simulink model "Adaptive_CT_ur10v"  (R2021b)
(part 5 of 20)

Y = ft_5({t100,t1002,t1003,t1004,t1005,t1006,t1007,t1008,t1009,t101,t1010,t1011,t1012,t1013,t1014,t1015,t1016,t1017,t1018,t1019,t1020,t1021,t1022,t1023,t1024,t1025,t1026,t1028,t1029,t1030,t1033,t1034,t1035,t1036,t1038,t104,t1041,t1045,t1046,t1047,t1048,t1049,t1050,t1051,t1052,t1053,t1054,t1055,t1056,t1058,t1059,t106,t1062,t1065,t1066,t1068,t1069,t107,t1070,t1071,t1073,t1074,t1079,t108,t1080,t1082,t1085,t1086,t1087,t1089,t1092,t1093,t1094,t1096,t1097,t1098,t1099,t1106,t1108,t111,t1111,t1119,t112,t1121,t1122,t1123,t1125,t1126,t1128,t1129,t113,t1130,t1131,t1133,t1134,t1135,t1137,t1138,t1139,t1140,t1152,t1153,t1155,t1156,t1157,t1158,t1159,t1161,t1164,t1166,t1167,t1168,t1171,t1172,t1173,t1174,t1178,t1179,t1183,t1184,t1185,t1186,t1187,t1189,t1192,t1193,t1196,t1198,t1199,t12,t1201,t1202,t1203,t1204,t1205,t1208,t1209,t1210,t1211,t1216,t1218,t1219,t1220,t1221,t1222,t1224,t1225,t1226,t1227,t1229,t1230,t1231,t1232,t1233,t1235,t1236,t1237,t1238,t124,t1242,t1245,t1246,t1248,t1250,t1251,t1252,t1255,t1261,t1264,t1265,t1267,t1268,t1269,t127,t1270,t1274,t1277,t1278,t128,t1280,t1283,t1284,t1285,t1287,t1288,t1292,t1294,t1297,t1298,t13,t1300,t1302,t1306,t1307,t131,t1310,t1311,t1313,t1314,t1315,t1316,t1318,t132,t1321,t1323,t1324,t1325,t1328,t1329,t1330,t1331,t1332,t1333,t1334,t1335,t1336,t1337,t1338,t1339,t134,t1341,t1343,t1344,t1345,t1352,t1353,t1354,t1355,t1357,t1358,t136,t1360,t1362,t1366,t1368,t1369,t137,t1370,t1371,t1374,t1375,t1376,t1378,t138,t1382,t1383,t1387,t1389,t1390,t1391,t1392,t1393,t1396,t1398,t1399,t14,t1400,t1402,t1403,t1406,t1407,t1409,t1410,t1411,t1413,t1414,t1415,t1416,t1417,t1418,t1419,t1420,t1421,t1422,t1423,t1425,t1426,t1427,t1434,t1435,t1436,t1437,t1440,t1445,t1446,t1451,t1456,t1458,t1459,t1461,t1462,t1463,t1468,t1470,t1471,t1472,t1474,t1475,t1478,t1483,t1485,t1486,t1491,t1492,t1493,t1494,t1495,t1497,t1499,t15,t150,t1500,t1501,t1503,t1504,t1506,t1507,t1508,t1509,t1516,t1517,t1518,t1519,t152,t1520,t1521,t1523,t1524,t1525,t1527,t1528,t1529,t1531,t1532,t1533,t1534,t1535,t1536,t1537,t1538,t1543,t1545,t1546,t1547,t155,t1552,t1553,t1554,t156,t1574,t158,t1580,t1583,t1585,t1586,t1587,t1588,t1589,t159,t1590,t1591,t1593,t1594,t1599,t1606,t1607,t1610,t1615,t1616,t1618,t162,t1625,t1627,t1628,t163,t1630,t1631,t1632,t1633,t1634,t1635,t1636,t1637,t164,t1644,t1645,t1646,t165,t1650,t1651,t1652,t1653,t1655,t1657,t1659,t1661,t1666,t1667,t1668,t1669,t1670,t1672,t1674,t1675,t1676,t1677,t1678,t1680,t1683,t1684,t1687,t1688,t1690,t1692,t1693,t1695,t1699,t1701,t1704,t1706,t1708,t1709,t171,t1710,t1713,t1714,t1715,t1723,t1724,t1726,t1727,t173,t1733,t1736,t1739,t174,t1740,t1741,t1742,t1743,t1749,t175,t1750,t1751,t1752,t1754,t1755,t1756,t1758,t1759,t1761,t1762,t1768,t1769,t177,t1770,t1771,t1773,t1774,t1775,t1776,t1777,t1778,t1779,t1780,t1781,t1783,t1784,t1786,t1792,t1793,t1794,t1795,t1797,t1799,t18,t1800,t1801,t1805,t1806,t1807,t1808,t1809,t1814,t1815,t1816,t1818,t1819,t1820,t1825,t1826,t1827,t1829,t1830,t1832,t1834,t1835,t1837,t1840,t1844,t1845,t1846,t1848,t1855,t1856,t1861,t1862,t1863,t1865,t1866,t1867,t1868,t1869,t187,t1871,t1874,t1875,t1876,t1877,t1878,t1880,t1881,t1882,t1886,t1888,t1889,t1890,t1891,t1893,t1895,t1897,t1898,t19,t1905,t1907,t1909,t191,t1910,t1916,t1919,t1920,t1921,t1922,t1924,t1925,t1928,t1930,t1931,t1932,t1935,t1937,t1938,t1944,t1947,t1949,t1953,t1959,t196,t1961,t1962,t1963,t1965,t1966,t1968,t1969,t1971,t1972,t1973,t1976,t1977,t1983,t1984,t1985,t1988,t199,t1990,t1995,t1996,t1999,t1d,t1dd,t200,t201,t2017,t202,t2023,t2027,t2028,t2030,t2032,t2037,t2044,t2049,t2058,t2059,t206,t2060,t2061,t2063,t2064,t2067,t2068,t2070,t2074,t2075,t2078,t2079,t2080,t2081,t2082,t2085,t2086,t2087,t2090,t2091,t2092,t2093,t2094,t2096,t2097,t21,t210,t2100,t2101,t2103,t2109,t2110,t2112,t2113,t2117,t2118,t2119,t2121,t2122,t2123,t2124,t2127,t2128,t2131,t2132,t2133,t2134,t2135,t2136,t2137,t2138,t2139,t2140,t2141,t2142,t2144,t2145,t2147,t215,t2150,t2153,t2155,t2156,t2159,t2160,t2161,t2162,t2167,t2168,t2169,t2170,t2171,t2172,t2173,t2174,t2177,t2178,t2180,t2181,t2183,t2184,t2189,t219,t2190,t2193,t2194,t2196,t2198,t2199,t22,t220,t2200,t2202,t2204,t2206,t2207,t221,t2210,t2211,t2212,t2216,t2219,t2221,t2222,t2225,t2227,t2228,t2233,t2235,t2240,t2241,t2243,t2244,t2245,t2247,t2256,t2257,t2259,t226,t2260,t2261,t2262,t2263,t2264,t2265,t2267,t2270,t2279,t2281,t2283,t2286,t229,t2292,t2294,t2298,t23,t2300,t231,t2311,t2315,t2318,t232,t2323,t233,t2335,t2339,t2340,t2343,t2344,t2345,t2346,t2347,t2348,t2352,t2353,t2354,t2357,t2359,t2363,t2365,t2366,t2368,t2370,t2371,t2372,t2374,t2379,t2380,t2382,t2385,t2388,t2389,t2390,t2391,t2393,t2395,t2397,t2398,t2399,t24,t2400,t2401,t2402,t2403,t2405,t2406,t2407,t2408,t2409,t2410,t2412,t2413,t2414,t2416,t2417,t2423,t2424,t2426,t2428,t243,t2434,t2438,t2439,t244,t2440,t2441,t2447,t2448,t245,t2453,t2454,t2457,t2458,t2462,t2467,t247,t2471,t2472,t2473,t2474,t2475,t2477,t2478,t248,t2480,t2481,t2484,t2485,t249,t2490,t2497,t25,t2505,t2507,t2508,t2509,t2511,t2515,t2516,t2518,t2519,t2520,t2523,t2524,t2527,t2529,t2530,t2547,t255,t2553,t2554,t2557,t256,t2560,t2565,t2571,t2572,t2576,t2578,t258,t2580,t2581,t2593,t2599,t26,t2606,t2608,t2611,t2619,t2623,t2628,t2630,t2631,t2635,t2642,t2644,t2648,t2649,t2650,t2651,t2653,t2654,t2655,t2658,t2659,t2662,t2663,t2664,t2666,t2671,t2672,t2678,t2680,t2682,t2686,t2687,t2688,t2690,t2694,t2695,t27,t2702,t2704,t2705,t2708,t2711,t2715,t2718,t2719,t2723,t2724,t2727,t2729,t2731,t2736,t2737,t2739,t2741,t2743,t2744,t2745,t2747,t2749,t2750,t2753,t2755,t2760,t2761,t2762,t2764,t2765,t2766,t2768,t2772,t2775,t2776,t2777,t2779,t2780,t2781,t2783,t279,t2790,t2794,t2796,t2798,t2799,t28,t2807,t2813,t2824,t2826,t283,t2838,t2839,t2841,t2843,t2849,t2860,t2862,t2863,t2868,t2871,t2876,t2877,t2879,t2894,t2897,t29,t2901,t2912,t2914,t2915,t2916,t2919,t2925,t2927,t2929,t2934,t2936,t2937,t2946,t2947,t2951,t2952,t2953,t2954,t2956,t2959,t2966,t2970,t2971,t2978,t2979,t2983,t2985,t2989,t299,t2992,t2995,t2996,t2999,t2d,t2dd,t30,t3007,t3008,t301,t3012,t3013,t3014,t3018,t3023,t3028,t303,t3030,t3031,t3032,t3033,t3035,t3038,t3039,t3042,t3043,t3059,t3060,t3066,t3069,t3071,t3072,t3073,t3078,t3079,t308,t3080,t3082,t3083,t3086,t3087,t3088,t309,t3099,t31,t3101,t3102,t3103,t3122,t3123,t3125,t3129,t3130,t3148,t315,t3154,t3160,t3163,t3166,t3168,t3169,t317,t3175,t3176,t3177,t318,t3183,t3185,t319,t320,t3207,t321,t3214,t3230,t3232,t3234,t3237,t325,t3250,t3251,t3259,t3260,t3272,t3288,t3289,t329,t3291,t3292,t3298,t330,t3306,t3308,t331,t3318,t332,t3321,t333,t3330,t3331,t3332,t3335,t334,t3340,t3341,t3342,t3343,t3345,t3348,t3349,t3351,t3354,t3355,t3360,t3368,t3381,t3383,t3384,t3388,t3391,t3399,t34,t3400,t3401,t3404,t3405,t341,t3414,t3415,t3416,t342,t3421,t3429,t343,t3431,t3432,t3433,t3439,t344,t3440,t3445,t345,t3452,t3456,t3457,t3458,t3459,t346,t3460,t3461,t3466,t3467,t3468,t3469,t347,t3488,t3498,t35,t3500,t3504,t3509,t3510,t3513,t3516,t3517,t3523,t3531,t354,t3543,t3544,t3546,t3556,t3557,t3567,t3568,t3574,t3575,t3578,t3579,t3580,t3582,t3590,t3598,t36,t3601,t3606,t3612,t3617,t3622,t3628,t3630,t364,t3649,t365,t3674,t3678,t368,t3683,t3685,t3686,t3687,t3697,t37,t3701,t3704,t3712,t3716,t3721,t3724,t3734,t3741,t3743,t3744,t3745,t3747,t3750,t3751,t3758,t3761,t3768,t3769,t3770,t3771,t3779,t3785,t3786,t3792,t3796,t38,t3813,t3817,t3821,t3822,t3830,t384,t3840,t3843,t3846,t3852,t3853,t3871,t3872,t3875,t3877,t3878,t3897,t39,t3903,t3906,t3907,t392,t3923,t393,t394,t3940,t3941,t3943,t395,t3d,t3dd,t401,t402,t4025,t403,t404,t4059,t4069,t4071,t4075,t4076,t4084,t4086,t4098,t41,t410,t411,t412,t4126,t4129,t413,t4133,t4134,t4135,t4139,t414,t4140,t4144,t4146,t4147,t415,t4150,t4152,t4157,t4159,t416,t4172,t418,t419,t42,t420,t4203,t4207,t4212,t4230,t4236,t425,t4299,t43,t4304,t431,t4325,t4332,t434,t437,t441,t442,t443,t444,t446,t4466,t453,t4538,t454,t455,t4551,t4579,t459,t467,t470,t478,t48,t483,t484,t486,t487,t488,t489,t492,t493,t494,t495,t496,t497,t498,t499,t4d,t4dd,t50,t501,t502,t503,t508,t51,t514,t515,t516,t519,t523,t524,t529,t53,t530,t531,t532,t537,t542,t543,t544,t546,t547,t548,t549,t55,t550,t552,t553,t554,t56,t562,t566,t569,t57,t570,t58,t580,t582,t587,t588,t589,t590,t591,t593,t595,t596,t598,t5d,t5dd,t600,t601,t602,t604,t605,t608,t609,t61,t612,t614,t615,t616,t617,t623,t627,t63,t631,t632,t633,t634,t635,t636,t637,t639,t641,t642,t643,t644,t645,t646,t647,t648,t649,t650,t651,t652,t653,t654,t655,t658,t659,t660,t662,t663,t664,t665,t667,t668,t669,t670,t671,t673,t675,t680,t681,t682,t684,t685,t687,t689,t69,t690,t694,t695,t696,t698,t699,t6d,t6dd,t701,t702,t703,t705,t706,t71,t711,t712,t713,t714,t720,t721,t723,t724,t725,t726,t729,t731,t732,t733,t735,t736,t738,t739,t740,t742,t745,t746,t747,t748,t749,t75,t752,t755,t759,t760,t761,t763,t764,t772,t774,t775,t776,t780,t781,t782,t785,t788,t789,t793,t799,t8,t802,t805,t806,t807,t808,t817,t82,t820,t823,t824,t825,t826,t827,t828,t830,t831,t832,t833,t835,t836,t838,t842,t843,t844,t846,t848,t849,t850,t851,t852,t853,t854,t855,t859,t861,t865,t866,t869,t870,t871,t873,t874,t879,t88,t880,t882,t883,t884,t885,t887,t888,t889,t890,t891,t892,t895,t896,t897,t898,t899,t9,t900,t904,t907,t908,t909,t910,t911,t912,t915,t917,t919,t922,t923,t927,t928,t931,t932,t937,t938,t943,t944,t945,t952,t954,t955,t956,t959,t960,t961,t962,t963,t964,t965,t966,t968,t969,t970,t972,t973,t974,t975,t978,t979,t980,t981,t982,t983,t984,t985,t986,t987,t989,t992,t993,t994,t997,t999});
end
function Y = ft_5(ct)
t100 = ct{1};
t1002 = ct{2};
t1003 = ct{3};
t1004 = ct{4};
t1005 = ct{5};
t1006 = ct{6};
t1007 = ct{7};
t1008 = ct{8};
t1009 = ct{9};
t101 = ct{10};
t1010 = ct{11};
t1011 = ct{12};
t1012 = ct{13};
t1013 = ct{14};
t1014 = ct{15};
t1015 = ct{16};
t1016 = ct{17};
t1017 = ct{18};
t1018 = ct{19};
t1019 = ct{20};
t1020 = ct{21};
t1021 = ct{22};
t1022 = ct{23};
t1023 = ct{24};
t1024 = ct{25};
t1025 = ct{26};
t1026 = ct{27};
t1028 = ct{28};
t1029 = ct{29};
t1030 = ct{30};
t1033 = ct{31};
t1034 = ct{32};
t1035 = ct{33};
t1036 = ct{34};
t1038 = ct{35};
t104 = ct{36};
t1041 = ct{37};
t1045 = ct{38};
t1046 = ct{39};
t1047 = ct{40};
t1048 = ct{41};
t1049 = ct{42};
t1050 = ct{43};
t1051 = ct{44};
t1052 = ct{45};
t1053 = ct{46};
t1054 = ct{47};
t1055 = ct{48};
t1056 = ct{49};
t1058 = ct{50};
t1059 = ct{51};
t106 = ct{52};
t1062 = ct{53};
t1065 = ct{54};
t1066 = ct{55};
t1068 = ct{56};
t1069 = ct{57};
t107 = ct{58};
t1070 = ct{59};
t1071 = ct{60};
t1073 = ct{61};
t1074 = ct{62};
t1079 = ct{63};
t108 = ct{64};
t1080 = ct{65};
t1082 = ct{66};
t1085 = ct{67};
t1086 = ct{68};
t1087 = ct{69};
t1089 = ct{70};
t1092 = ct{71};
t1093 = ct{72};
t1094 = ct{73};
t1096 = ct{74};
t1097 = ct{75};
t1098 = ct{76};
t1099 = ct{77};
t1106 = ct{78};
t1108 = ct{79};
t111 = ct{80};
t1111 = ct{81};
t1119 = ct{82};
t112 = ct{83};
t1121 = ct{84};
t1122 = ct{85};
t1123 = ct{86};
t1125 = ct{87};
t1126 = ct{88};
t1128 = ct{89};
t1129 = ct{90};
t113 = ct{91};
t1130 = ct{92};
t1131 = ct{93};
t1133 = ct{94};
t1134 = ct{95};
t1135 = ct{96};
t1137 = ct{97};
t1138 = ct{98};
t1139 = ct{99};
t1140 = ct{100};
t1152 = ct{101};
t1153 = ct{102};
t1155 = ct{103};
t1156 = ct{104};
t1157 = ct{105};
t1158 = ct{106};
t1159 = ct{107};
t1161 = ct{108};
t1164 = ct{109};
t1166 = ct{110};
t1167 = ct{111};
t1168 = ct{112};
t1171 = ct{113};
t1172 = ct{114};
t1173 = ct{115};
t1174 = ct{116};
t1178 = ct{117};
t1179 = ct{118};
t1183 = ct{119};
t1184 = ct{120};
t1185 = ct{121};
t1186 = ct{122};
t1187 = ct{123};
t1189 = ct{124};
t1192 = ct{125};
t1193 = ct{126};
t1196 = ct{127};
t1198 = ct{128};
t1199 = ct{129};
t12 = ct{130};
t1201 = ct{131};
t1202 = ct{132};
t1203 = ct{133};
t1204 = ct{134};
t1205 = ct{135};
t1208 = ct{136};
t1209 = ct{137};
t1210 = ct{138};
t1211 = ct{139};
t1216 = ct{140};
t1218 = ct{141};
t1219 = ct{142};
t1220 = ct{143};
t1221 = ct{144};
t1222 = ct{145};
t1224 = ct{146};
t1225 = ct{147};
t1226 = ct{148};
t1227 = ct{149};
t1229 = ct{150};
t1230 = ct{151};
t1231 = ct{152};
t1232 = ct{153};
t1233 = ct{154};
t1235 = ct{155};
t1236 = ct{156};
t1237 = ct{157};
t1238 = ct{158};
t124 = ct{159};
t1242 = ct{160};
t1245 = ct{161};
t1246 = ct{162};
t1248 = ct{163};
t1250 = ct{164};
t1251 = ct{165};
t1252 = ct{166};
t1255 = ct{167};
t1261 = ct{168};
t1264 = ct{169};
t1265 = ct{170};
t1267 = ct{171};
t1268 = ct{172};
t1269 = ct{173};
t127 = ct{174};
t1270 = ct{175};
t1274 = ct{176};
t1277 = ct{177};
t1278 = ct{178};
t128 = ct{179};
t1280 = ct{180};
t1283 = ct{181};
t1284 = ct{182};
t1285 = ct{183};
t1287 = ct{184};
t1288 = ct{185};
t1292 = ct{186};
t1294 = ct{187};
t1297 = ct{188};
t1298 = ct{189};
t13 = ct{190};
t1300 = ct{191};
t1302 = ct{192};
t1306 = ct{193};
t1307 = ct{194};
t131 = ct{195};
t1310 = ct{196};
t1311 = ct{197};
t1313 = ct{198};
t1314 = ct{199};
t1315 = ct{200};
t1316 = ct{201};
t1318 = ct{202};
t132 = ct{203};
t1321 = ct{204};
t1323 = ct{205};
t1324 = ct{206};
t1325 = ct{207};
t1328 = ct{208};
t1329 = ct{209};
t1330 = ct{210};
t1331 = ct{211};
t1332 = ct{212};
t1333 = ct{213};
t1334 = ct{214};
t1335 = ct{215};
t1336 = ct{216};
t1337 = ct{217};
t1338 = ct{218};
t1339 = ct{219};
t134 = ct{220};
t1341 = ct{221};
t1343 = ct{222};
t1344 = ct{223};
t1345 = ct{224};
t1352 = ct{225};
t1353 = ct{226};
t1354 = ct{227};
t1355 = ct{228};
t1357 = ct{229};
t1358 = ct{230};
t136 = ct{231};
t1360 = ct{232};
t1362 = ct{233};
t1366 = ct{234};
t1368 = ct{235};
t1369 = ct{236};
t137 = ct{237};
t1370 = ct{238};
t1371 = ct{239};
t1374 = ct{240};
t1375 = ct{241};
t1376 = ct{242};
t1378 = ct{243};
t138 = ct{244};
t1382 = ct{245};
t1383 = ct{246};
t1387 = ct{247};
t1389 = ct{248};
t1390 = ct{249};
t1391 = ct{250};
t1392 = ct{251};
t1393 = ct{252};
t1396 = ct{253};
t1398 = ct{254};
t1399 = ct{255};
t14 = ct{256};
t1400 = ct{257};
t1402 = ct{258};
t1403 = ct{259};
t1406 = ct{260};
t1407 = ct{261};
t1409 = ct{262};
t1410 = ct{263};
t1411 = ct{264};
t1413 = ct{265};
t1414 = ct{266};
t1415 = ct{267};
t1416 = ct{268};
t1417 = ct{269};
t1418 = ct{270};
t1419 = ct{271};
t1420 = ct{272};
t1421 = ct{273};
t1422 = ct{274};
t1423 = ct{275};
t1425 = ct{276};
t1426 = ct{277};
t1427 = ct{278};
t1434 = ct{279};
t1435 = ct{280};
t1436 = ct{281};
t1437 = ct{282};
t1440 = ct{283};
t1445 = ct{284};
t1446 = ct{285};
t1451 = ct{286};
t1456 = ct{287};
t1458 = ct{288};
t1459 = ct{289};
t1461 = ct{290};
t1462 = ct{291};
t1463 = ct{292};
t1468 = ct{293};
t1470 = ct{294};
t1471 = ct{295};
t1472 = ct{296};
t1474 = ct{297};
t1475 = ct{298};
t1478 = ct{299};
t1483 = ct{300};
t1485 = ct{301};
t1486 = ct{302};
t1491 = ct{303};
t1492 = ct{304};
t1493 = ct{305};
t1494 = ct{306};
t1495 = ct{307};
t1497 = ct{308};
t1499 = ct{309};
t15 = ct{310};
t150 = ct{311};
t1500 = ct{312};
t1501 = ct{313};
t1503 = ct{314};
t1504 = ct{315};
t1506 = ct{316};
t1507 = ct{317};
t1508 = ct{318};
t1509 = ct{319};
t1516 = ct{320};
t1517 = ct{321};
t1518 = ct{322};
t1519 = ct{323};
t152 = ct{324};
t1520 = ct{325};
t1521 = ct{326};
t1523 = ct{327};
t1524 = ct{328};
t1525 = ct{329};
t1527 = ct{330};
t1528 = ct{331};
t1529 = ct{332};
t1531 = ct{333};
t1532 = ct{334};
t1533 = ct{335};
t1534 = ct{336};
t1535 = ct{337};
t1536 = ct{338};
t1537 = ct{339};
t1538 = ct{340};
t1543 = ct{341};
t1545 = ct{342};
t1546 = ct{343};
t1547 = ct{344};
t155 = ct{345};
t1552 = ct{346};
t1553 = ct{347};
t1554 = ct{348};
t156 = ct{349};
t1574 = ct{350};
t158 = ct{351};
t1580 = ct{352};
t1583 = ct{353};
t1585 = ct{354};
t1586 = ct{355};
t1587 = ct{356};
t1588 = ct{357};
t1589 = ct{358};
t159 = ct{359};
t1590 = ct{360};
t1591 = ct{361};
t1593 = ct{362};
t1594 = ct{363};
t1599 = ct{364};
t1606 = ct{365};
t1607 = ct{366};
t1610 = ct{367};
t1615 = ct{368};
t1616 = ct{369};
t1618 = ct{370};
t162 = ct{371};
t1625 = ct{372};
t1627 = ct{373};
t1628 = ct{374};
t163 = ct{375};
t1630 = ct{376};
t1631 = ct{377};
t1632 = ct{378};
t1633 = ct{379};
t1634 = ct{380};
t1635 = ct{381};
t1636 = ct{382};
t1637 = ct{383};
t164 = ct{384};
t1644 = ct{385};
t1645 = ct{386};
t1646 = ct{387};
t165 = ct{388};
t1650 = ct{389};
t1651 = ct{390};
t1652 = ct{391};
t1653 = ct{392};
t1655 = ct{393};
t1657 = ct{394};
t1659 = ct{395};
t1661 = ct{396};
t1666 = ct{397};
t1667 = ct{398};
t1668 = ct{399};
t1669 = ct{400};
t1670 = ct{401};
t1672 = ct{402};
t1674 = ct{403};
t1675 = ct{404};
t1676 = ct{405};
t1677 = ct{406};
t1678 = ct{407};
t1680 = ct{408};
t1683 = ct{409};
t1684 = ct{410};
t1687 = ct{411};
t1688 = ct{412};
t1690 = ct{413};
t1692 = ct{414};
t1693 = ct{415};
t1695 = ct{416};
t1699 = ct{417};
t1701 = ct{418};
t1704 = ct{419};
t1706 = ct{420};
t1708 = ct{421};
t1709 = ct{422};
t171 = ct{423};
t1710 = ct{424};
t1713 = ct{425};
t1714 = ct{426};
t1715 = ct{427};
t1723 = ct{428};
t1724 = ct{429};
t1726 = ct{430};
t1727 = ct{431};
t173 = ct{432};
t1733 = ct{433};
t1736 = ct{434};
t1739 = ct{435};
t174 = ct{436};
t1740 = ct{437};
t1741 = ct{438};
t1742 = ct{439};
t1743 = ct{440};
t1749 = ct{441};
t175 = ct{442};
t1750 = ct{443};
t1751 = ct{444};
t1752 = ct{445};
t1754 = ct{446};
t1755 = ct{447};
t1756 = ct{448};
t1758 = ct{449};
t1759 = ct{450};
t1761 = ct{451};
t1762 = ct{452};
t1768 = ct{453};
t1769 = ct{454};
t177 = ct{455};
t1770 = ct{456};
t1771 = ct{457};
t1773 = ct{458};
t1774 = ct{459};
t1775 = ct{460};
t1776 = ct{461};
t1777 = ct{462};
t1778 = ct{463};
t1779 = ct{464};
t1780 = ct{465};
t1781 = ct{466};
t1783 = ct{467};
t1784 = ct{468};
t1786 = ct{469};
t1792 = ct{470};
t1793 = ct{471};
t1794 = ct{472};
t1795 = ct{473};
t1797 = ct{474};
t1799 = ct{475};
t18 = ct{476};
t1800 = ct{477};
t1801 = ct{478};
t1805 = ct{479};
t1806 = ct{480};
t1807 = ct{481};
t1808 = ct{482};
t1809 = ct{483};
t1814 = ct{484};
t1815 = ct{485};
t1816 = ct{486};
t1818 = ct{487};
t1819 = ct{488};
t1820 = ct{489};
t1825 = ct{490};
t1826 = ct{491};
t1827 = ct{492};
t1829 = ct{493};
t1830 = ct{494};
t1832 = ct{495};
t1834 = ct{496};
t1835 = ct{497};
t1837 = ct{498};
t1840 = ct{499};
t1844 = ct{500};
t1845 = ct{501};
t1846 = ct{502};
t1848 = ct{503};
t1855 = ct{504};
t1856 = ct{505};
t1861 = ct{506};
t1862 = ct{507};
t1863 = ct{508};
t1865 = ct{509};
t1866 = ct{510};
t1867 = ct{511};
t1868 = ct{512};
t1869 = ct{513};
t187 = ct{514};
t1871 = ct{515};
t1874 = ct{516};
t1875 = ct{517};
t1876 = ct{518};
t1877 = ct{519};
t1878 = ct{520};
t1880 = ct{521};
t1881 = ct{522};
t1882 = ct{523};
t1886 = ct{524};
t1888 = ct{525};
t1889 = ct{526};
t1890 = ct{527};
t1891 = ct{528};
t1893 = ct{529};
t1895 = ct{530};
t1897 = ct{531};
t1898 = ct{532};
t19 = ct{533};
t1905 = ct{534};
t1907 = ct{535};
t1909 = ct{536};
t191 = ct{537};
t1910 = ct{538};
t1916 = ct{539};
t1919 = ct{540};
t1920 = ct{541};
t1921 = ct{542};
t1922 = ct{543};
t1924 = ct{544};
t1925 = ct{545};
t1928 = ct{546};
t1930 = ct{547};
t1931 = ct{548};
t1932 = ct{549};
t1935 = ct{550};
t1937 = ct{551};
t1938 = ct{552};
t1944 = ct{553};
t1947 = ct{554};
t1949 = ct{555};
t1953 = ct{556};
t1959 = ct{557};
t196 = ct{558};
t1961 = ct{559};
t1962 = ct{560};
t1963 = ct{561};
t1965 = ct{562};
t1966 = ct{563};
t1968 = ct{564};
t1969 = ct{565};
t1971 = ct{566};
t1972 = ct{567};
t1973 = ct{568};
t1976 = ct{569};
t1977 = ct{570};
t1983 = ct{571};
t1984 = ct{572};
t1985 = ct{573};
t1988 = ct{574};
t199 = ct{575};
t1990 = ct{576};
t1995 = ct{577};
t1996 = ct{578};
t1999 = ct{579};
t1d = ct{580};
t1dd = ct{581};
t200 = ct{582};
t201 = ct{583};
t2017 = ct{584};
t202 = ct{585};
t2023 = ct{586};
t2027 = ct{587};
t2028 = ct{588};
t2030 = ct{589};
t2032 = ct{590};
t2037 = ct{591};
t2044 = ct{592};
t2049 = ct{593};
t2058 = ct{594};
t2059 = ct{595};
t206 = ct{596};
t2060 = ct{597};
t2061 = ct{598};
t2063 = ct{599};
t2064 = ct{600};
t2067 = ct{601};
t2068 = ct{602};
t2070 = ct{603};
t2074 = ct{604};
t2075 = ct{605};
t2078 = ct{606};
t2079 = ct{607};
t2080 = ct{608};
t2081 = ct{609};
t2082 = ct{610};
t2085 = ct{611};
t2086 = ct{612};
t2087 = ct{613};
t2090 = ct{614};
t2091 = ct{615};
t2092 = ct{616};
t2093 = ct{617};
t2094 = ct{618};
t2096 = ct{619};
t2097 = ct{620};
t21 = ct{621};
t210 = ct{622};
t2100 = ct{623};
t2101 = ct{624};
t2103 = ct{625};
t2109 = ct{626};
t2110 = ct{627};
t2112 = ct{628};
t2113 = ct{629};
t2117 = ct{630};
t2118 = ct{631};
t2119 = ct{632};
t2121 = ct{633};
t2122 = ct{634};
t2123 = ct{635};
t2124 = ct{636};
t2127 = ct{637};
t2128 = ct{638};
t2131 = ct{639};
t2132 = ct{640};
t2133 = ct{641};
t2134 = ct{642};
t2135 = ct{643};
t2136 = ct{644};
t2137 = ct{645};
t2138 = ct{646};
t2139 = ct{647};
t2140 = ct{648};
t2141 = ct{649};
t2142 = ct{650};
t2144 = ct{651};
t2145 = ct{652};
t2147 = ct{653};
t215 = ct{654};
t2150 = ct{655};
t2153 = ct{656};
t2155 = ct{657};
t2156 = ct{658};
t2159 = ct{659};
t2160 = ct{660};
t2161 = ct{661};
t2162 = ct{662};
t2167 = ct{663};
t2168 = ct{664};
t2169 = ct{665};
t2170 = ct{666};
t2171 = ct{667};
t2172 = ct{668};
t2173 = ct{669};
t2174 = ct{670};
t2177 = ct{671};
t2178 = ct{672};
t2180 = ct{673};
t2181 = ct{674};
t2183 = ct{675};
t2184 = ct{676};
t2189 = ct{677};
t219 = ct{678};
t2190 = ct{679};
t2193 = ct{680};
t2194 = ct{681};
t2196 = ct{682};
t2198 = ct{683};
t2199 = ct{684};
t22 = ct{685};
t220 = ct{686};
t2200 = ct{687};
t2202 = ct{688};
t2204 = ct{689};
t2206 = ct{690};
t2207 = ct{691};
t221 = ct{692};
t2210 = ct{693};
t2211 = ct{694};
t2212 = ct{695};
t2216 = ct{696};
t2219 = ct{697};
t2221 = ct{698};
t2222 = ct{699};
t2225 = ct{700};
t2227 = ct{701};
t2228 = ct{702};
t2233 = ct{703};
t2235 = ct{704};
t2240 = ct{705};
t2241 = ct{706};
t2243 = ct{707};
t2244 = ct{708};
t2245 = ct{709};
t2247 = ct{710};
t2256 = ct{711};
t2257 = ct{712};
t2259 = ct{713};
t226 = ct{714};
t2260 = ct{715};
t2261 = ct{716};
t2262 = ct{717};
t2263 = ct{718};
t2264 = ct{719};
t2265 = ct{720};
t2267 = ct{721};
t2270 = ct{722};
t2279 = ct{723};
t2281 = ct{724};
t2283 = ct{725};
t2286 = ct{726};
t229 = ct{727};
t2292 = ct{728};
t2294 = ct{729};
t2298 = ct{730};
t23 = ct{731};
t2300 = ct{732};
t231 = ct{733};
t2311 = ct{734};
t2315 = ct{735};
t2318 = ct{736};
t232 = ct{737};
t2323 = ct{738};
t233 = ct{739};
t2335 = ct{740};
t2339 = ct{741};
t2340 = ct{742};
t2343 = ct{743};
t2344 = ct{744};
t2345 = ct{745};
t2346 = ct{746};
t2347 = ct{747};
t2348 = ct{748};
t2352 = ct{749};
t2353 = ct{750};
t2354 = ct{751};
t2357 = ct{752};
t2359 = ct{753};
t2363 = ct{754};
t2365 = ct{755};
t2366 = ct{756};
t2368 = ct{757};
t2370 = ct{758};
t2371 = ct{759};
t2372 = ct{760};
t2374 = ct{761};
t2379 = ct{762};
t2380 = ct{763};
t2382 = ct{764};
t2385 = ct{765};
t2388 = ct{766};
t2389 = ct{767};
t2390 = ct{768};
t2391 = ct{769};
t2393 = ct{770};
t2395 = ct{771};
t2397 = ct{772};
t2398 = ct{773};
t2399 = ct{774};
t24 = ct{775};
t2400 = ct{776};
t2401 = ct{777};
t2402 = ct{778};
t2403 = ct{779};
t2405 = ct{780};
t2406 = ct{781};
t2407 = ct{782};
t2408 = ct{783};
t2409 = ct{784};
t2410 = ct{785};
t2412 = ct{786};
t2413 = ct{787};
t2414 = ct{788};
t2416 = ct{789};
t2417 = ct{790};
t2423 = ct{791};
t2424 = ct{792};
t2426 = ct{793};
t2428 = ct{794};
t243 = ct{795};
t2434 = ct{796};
t2438 = ct{797};
t2439 = ct{798};
t244 = ct{799};
t2440 = ct{800};
t2441 = ct{801};
t2447 = ct{802};
t2448 = ct{803};
t245 = ct{804};
t2453 = ct{805};
t2454 = ct{806};
t2457 = ct{807};
t2458 = ct{808};
t2462 = ct{809};
t2467 = ct{810};
t247 = ct{811};
t2471 = ct{812};
t2472 = ct{813};
t2473 = ct{814};
t2474 = ct{815};
t2475 = ct{816};
t2477 = ct{817};
t2478 = ct{818};
t248 = ct{819};
t2480 = ct{820};
t2481 = ct{821};
t2484 = ct{822};
t2485 = ct{823};
t249 = ct{824};
t2490 = ct{825};
t2497 = ct{826};
t25 = ct{827};
t2505 = ct{828};
t2507 = ct{829};
t2508 = ct{830};
t2509 = ct{831};
t2511 = ct{832};
t2515 = ct{833};
t2516 = ct{834};
t2518 = ct{835};
t2519 = ct{836};
t2520 = ct{837};
t2523 = ct{838};
t2524 = ct{839};
t2527 = ct{840};
t2529 = ct{841};
t2530 = ct{842};
t2547 = ct{843};
t255 = ct{844};
t2553 = ct{845};
t2554 = ct{846};
t2557 = ct{847};
t256 = ct{848};
t2560 = ct{849};
t2565 = ct{850};
t2571 = ct{851};
t2572 = ct{852};
t2576 = ct{853};
t2578 = ct{854};
t258 = ct{855};
t2580 = ct{856};
t2581 = ct{857};
t2593 = ct{858};
t2599 = ct{859};
t26 = ct{860};
t2606 = ct{861};
t2608 = ct{862};
t2611 = ct{863};
t2619 = ct{864};
t2623 = ct{865};
t2628 = ct{866};
t2630 = ct{867};
t2631 = ct{868};
t2635 = ct{869};
t2642 = ct{870};
t2644 = ct{871};
t2648 = ct{872};
t2649 = ct{873};
t2650 = ct{874};
t2651 = ct{875};
t2653 = ct{876};
t2654 = ct{877};
t2655 = ct{878};
t2658 = ct{879};
t2659 = ct{880};
t2662 = ct{881};
t2663 = ct{882};
t2664 = ct{883};
t2666 = ct{884};
t2671 = ct{885};
t2672 = ct{886};
t2678 = ct{887};
t2680 = ct{888};
t2682 = ct{889};
t2686 = ct{890};
t2687 = ct{891};
t2688 = ct{892};
t2690 = ct{893};
t2694 = ct{894};
t2695 = ct{895};
t27 = ct{896};
t2702 = ct{897};
t2704 = ct{898};
t2705 = ct{899};
t2708 = ct{900};
t2711 = ct{901};
t2715 = ct{902};
t2718 = ct{903};
t2719 = ct{904};
t2723 = ct{905};
t2724 = ct{906};
t2727 = ct{907};
t2729 = ct{908};
t2731 = ct{909};
t2736 = ct{910};
t2737 = ct{911};
t2739 = ct{912};
t2741 = ct{913};
t2743 = ct{914};
t2744 = ct{915};
t2745 = ct{916};
t2747 = ct{917};
t2749 = ct{918};
t2750 = ct{919};
t2753 = ct{920};
t2755 = ct{921};
t2760 = ct{922};
t2761 = ct{923};
t2762 = ct{924};
t2764 = ct{925};
t2765 = ct{926};
t2766 = ct{927};
t2768 = ct{928};
t2772 = ct{929};
t2775 = ct{930};
t2776 = ct{931};
t2777 = ct{932};
t2779 = ct{933};
t2780 = ct{934};
t2781 = ct{935};
t2783 = ct{936};
t279 = ct{937};
t2790 = ct{938};
t2794 = ct{939};
t2796 = ct{940};
t2798 = ct{941};
t2799 = ct{942};
t28 = ct{943};
t2807 = ct{944};
t2813 = ct{945};
t2824 = ct{946};
t2826 = ct{947};
t283 = ct{948};
t2838 = ct{949};
t2839 = ct{950};
t2841 = ct{951};
t2843 = ct{952};
t2849 = ct{953};
t2860 = ct{954};
t2862 = ct{955};
t2863 = ct{956};
t2868 = ct{957};
t2871 = ct{958};
t2876 = ct{959};
t2877 = ct{960};
t2879 = ct{961};
t2894 = ct{962};
t2897 = ct{963};
t29 = ct{964};
t2901 = ct{965};
t2912 = ct{966};
t2914 = ct{967};
t2915 = ct{968};
t2916 = ct{969};
t2919 = ct{970};
t2925 = ct{971};
t2927 = ct{972};
t2929 = ct{973};
t2934 = ct{974};
t2936 = ct{975};
t2937 = ct{976};
t2946 = ct{977};
t2947 = ct{978};
t2951 = ct{979};
t2952 = ct{980};
t2953 = ct{981};
t2954 = ct{982};
t2956 = ct{983};
t2959 = ct{984};
t2966 = ct{985};
t2970 = ct{986};
t2971 = ct{987};
t2978 = ct{988};
t2979 = ct{989};
t2983 = ct{990};
t2985 = ct{991};
t2989 = ct{992};
t299 = ct{993};
t2992 = ct{994};
t2995 = ct{995};
t2996 = ct{996};
t2999 = ct{997};
t2d = ct{998};
t2dd = ct{999};
t30 = ct{1000};
t3007 = ct{1001};
t3008 = ct{1002};
t301 = ct{1003};
t3012 = ct{1004};
t3013 = ct{1005};
t3014 = ct{1006};
t3018 = ct{1007};
t3023 = ct{1008};
t3028 = ct{1009};
t303 = ct{1010};
t3030 = ct{1011};
t3031 = ct{1012};
t3032 = ct{1013};
t3033 = ct{1014};
t3035 = ct{1015};
t3038 = ct{1016};
t3039 = ct{1017};
t3042 = ct{1018};
t3043 = ct{1019};
t3059 = ct{1020};
t3060 = ct{1021};
t3066 = ct{1022};
t3069 = ct{1023};
t3071 = ct{1024};
t3072 = ct{1025};
t3073 = ct{1026};
t3078 = ct{1027};
t3079 = ct{1028};
t308 = ct{1029};
t3080 = ct{1030};
t3082 = ct{1031};
t3083 = ct{1032};
t3086 = ct{1033};
t3087 = ct{1034};
t3088 = ct{1035};
t309 = ct{1036};
t3099 = ct{1037};
t31 = ct{1038};
t3101 = ct{1039};
t3102 = ct{1040};
t3103 = ct{1041};
t3122 = ct{1042};
t3123 = ct{1043};
t3125 = ct{1044};
t3129 = ct{1045};
t3130 = ct{1046};
t3148 = ct{1047};
t315 = ct{1048};
t3154 = ct{1049};
t3160 = ct{1050};
t3163 = ct{1051};
t3166 = ct{1052};
t3168 = ct{1053};
t3169 = ct{1054};
t317 = ct{1055};
t3175 = ct{1056};
t3176 = ct{1057};
t3177 = ct{1058};
t318 = ct{1059};
t3183 = ct{1060};
t3185 = ct{1061};
t319 = ct{1062};
t320 = ct{1063};
t3207 = ct{1064};
t321 = ct{1065};
t3214 = ct{1066};
t3230 = ct{1067};
t3232 = ct{1068};
t3234 = ct{1069};
t3237 = ct{1070};
t325 = ct{1071};
t3250 = ct{1072};
t3251 = ct{1073};
t3259 = ct{1074};
t3260 = ct{1075};
t3272 = ct{1076};
t3288 = ct{1077};
t3289 = ct{1078};
t329 = ct{1079};
t3291 = ct{1080};
t3292 = ct{1081};
t3298 = ct{1082};
t330 = ct{1083};
t3306 = ct{1084};
t3308 = ct{1085};
t331 = ct{1086};
t3318 = ct{1087};
t332 = ct{1088};
t3321 = ct{1089};
t333 = ct{1090};
t3330 = ct{1091};
t3331 = ct{1092};
t3332 = ct{1093};
t3335 = ct{1094};
t334 = ct{1095};
t3340 = ct{1096};
t3341 = ct{1097};
t3342 = ct{1098};
t3343 = ct{1099};
t3345 = ct{1100};
t3348 = ct{1101};
t3349 = ct{1102};
t3351 = ct{1103};
t3354 = ct{1104};
t3355 = ct{1105};
t3360 = ct{1106};
t3368 = ct{1107};
t3381 = ct{1108};
t3383 = ct{1109};
t3384 = ct{1110};
t3388 = ct{1111};
t3391 = ct{1112};
t3399 = ct{1113};
t34 = ct{1114};
t3400 = ct{1115};
t3401 = ct{1116};
t3404 = ct{1117};
t3405 = ct{1118};
t341 = ct{1119};
t3414 = ct{1120};
t3415 = ct{1121};
t3416 = ct{1122};
t342 = ct{1123};
t3421 = ct{1124};
t3429 = ct{1125};
t343 = ct{1126};
t3431 = ct{1127};
t3432 = ct{1128};
t3433 = ct{1129};
t3439 = ct{1130};
t344 = ct{1131};
t3440 = ct{1132};
t3445 = ct{1133};
t345 = ct{1134};
t3452 = ct{1135};
t3456 = ct{1136};
t3457 = ct{1137};
t3458 = ct{1138};
t3459 = ct{1139};
t346 = ct{1140};
t3460 = ct{1141};
t3461 = ct{1142};
t3466 = ct{1143};
t3467 = ct{1144};
t3468 = ct{1145};
t3469 = ct{1146};
t347 = ct{1147};
t3488 = ct{1148};
t3498 = ct{1149};
t35 = ct{1150};
t3500 = ct{1151};
t3504 = ct{1152};
t3509 = ct{1153};
t3510 = ct{1154};
t3513 = ct{1155};
t3516 = ct{1156};
t3517 = ct{1157};
t3523 = ct{1158};
t3531 = ct{1159};
t354 = ct{1160};
t3543 = ct{1161};
t3544 = ct{1162};
t3546 = ct{1163};
t3556 = ct{1164};
t3557 = ct{1165};
t3567 = ct{1166};
t3568 = ct{1167};
t3574 = ct{1168};
t3575 = ct{1169};
t3578 = ct{1170};
t3579 = ct{1171};
t3580 = ct{1172};
t3582 = ct{1173};
t3590 = ct{1174};
t3598 = ct{1175};
t36 = ct{1176};
t3601 = ct{1177};
t3606 = ct{1178};
t3612 = ct{1179};
t3617 = ct{1180};
t3622 = ct{1181};
t3628 = ct{1182};
t3630 = ct{1183};
t364 = ct{1184};
t3649 = ct{1185};
t365 = ct{1186};
t3674 = ct{1187};
t3678 = ct{1188};
t368 = ct{1189};
t3683 = ct{1190};
t3685 = ct{1191};
t3686 = ct{1192};
t3687 = ct{1193};
t3697 = ct{1194};
t37 = ct{1195};
t3701 = ct{1196};
t3704 = ct{1197};
t3712 = ct{1198};
t3716 = ct{1199};
t3721 = ct{1200};
t3724 = ct{1201};
t3734 = ct{1202};
t3741 = ct{1203};
t3743 = ct{1204};
t3744 = ct{1205};
t3745 = ct{1206};
t3747 = ct{1207};
t3750 = ct{1208};
t3751 = ct{1209};
t3758 = ct{1210};
t3761 = ct{1211};
t3768 = ct{1212};
t3769 = ct{1213};
t3770 = ct{1214};
t3771 = ct{1215};
t3779 = ct{1216};
t3785 = ct{1217};
t3786 = ct{1218};
t3792 = ct{1219};
t3796 = ct{1220};
t38 = ct{1221};
t3813 = ct{1222};
t3817 = ct{1223};
t3821 = ct{1224};
t3822 = ct{1225};
t3830 = ct{1226};
t384 = ct{1227};
t3840 = ct{1228};
t3843 = ct{1229};
t3846 = ct{1230};
t3852 = ct{1231};
t3853 = ct{1232};
t3871 = ct{1233};
t3872 = ct{1234};
t3875 = ct{1235};
t3877 = ct{1236};
t3878 = ct{1237};
t3897 = ct{1238};
t39 = ct{1239};
t3903 = ct{1240};
t3906 = ct{1241};
t3907 = ct{1242};
t392 = ct{1243};
t3923 = ct{1244};
t393 = ct{1245};
t394 = ct{1246};
t3940 = ct{1247};
t3941 = ct{1248};
t3943 = ct{1249};
t395 = ct{1250};
t3d = ct{1251};
t3dd = ct{1252};
t401 = ct{1253};
t402 = ct{1254};
t4025 = ct{1255};
t403 = ct{1256};
t404 = ct{1257};
t4059 = ct{1258};
t4069 = ct{1259};
t4071 = ct{1260};
t4075 = ct{1261};
t4076 = ct{1262};
t4084 = ct{1263};
t4086 = ct{1264};
t4098 = ct{1265};
t41 = ct{1266};
t410 = ct{1267};
t411 = ct{1268};
t412 = ct{1269};
t4126 = ct{1270};
t4129 = ct{1271};
t413 = ct{1272};
t4133 = ct{1273};
t4134 = ct{1274};
t4135 = ct{1275};
t4139 = ct{1276};
t414 = ct{1277};
t4140 = ct{1278};
t4144 = ct{1279};
t4146 = ct{1280};
t4147 = ct{1281};
t415 = ct{1282};
t4150 = ct{1283};
t4152 = ct{1284};
t4157 = ct{1285};
t4159 = ct{1286};
t416 = ct{1287};
t4172 = ct{1288};
t418 = ct{1289};
t419 = ct{1290};
t42 = ct{1291};
t420 = ct{1292};
t4203 = ct{1293};
t4207 = ct{1294};
t4212 = ct{1295};
t4230 = ct{1296};
t4236 = ct{1297};
t425 = ct{1298};
t4299 = ct{1299};
t43 = ct{1300};
t4304 = ct{1301};
t431 = ct{1302};
t4325 = ct{1303};
t4332 = ct{1304};
t434 = ct{1305};
t437 = ct{1306};
t441 = ct{1307};
t442 = ct{1308};
t443 = ct{1309};
t444 = ct{1310};
t446 = ct{1311};
t4466 = ct{1312};
t453 = ct{1313};
t4538 = ct{1314};
t454 = ct{1315};
t455 = ct{1316};
t4551 = ct{1317};
t4579 = ct{1318};
t459 = ct{1319};
t467 = ct{1320};
t470 = ct{1321};
t478 = ct{1322};
t48 = ct{1323};
t483 = ct{1324};
t484 = ct{1325};
t486 = ct{1326};
t487 = ct{1327};
t488 = ct{1328};
t489 = ct{1329};
t492 = ct{1330};
t493 = ct{1331};
t494 = ct{1332};
t495 = ct{1333};
t496 = ct{1334};
t497 = ct{1335};
t498 = ct{1336};
t499 = ct{1337};
t4d = ct{1338};
t4dd = ct{1339};
t50 = ct{1340};
t501 = ct{1341};
t502 = ct{1342};
t503 = ct{1343};
t508 = ct{1344};
t51 = ct{1345};
t514 = ct{1346};
t515 = ct{1347};
t516 = ct{1348};
t519 = ct{1349};
t523 = ct{1350};
t524 = ct{1351};
t529 = ct{1352};
t53 = ct{1353};
t530 = ct{1354};
t531 = ct{1355};
t532 = ct{1356};
t537 = ct{1357};
t542 = ct{1358};
t543 = ct{1359};
t544 = ct{1360};
t546 = ct{1361};
t547 = ct{1362};
t548 = ct{1363};
t549 = ct{1364};
t55 = ct{1365};
t550 = ct{1366};
t552 = ct{1367};
t553 = ct{1368};
t554 = ct{1369};
t56 = ct{1370};
t562 = ct{1371};
t566 = ct{1372};
t569 = ct{1373};
t57 = ct{1374};
t570 = ct{1375};
t58 = ct{1376};
t580 = ct{1377};
t582 = ct{1378};
t587 = ct{1379};
t588 = ct{1380};
t589 = ct{1381};
t590 = ct{1382};
t591 = ct{1383};
t593 = ct{1384};
t595 = ct{1385};
t596 = ct{1386};
t598 = ct{1387};
t5d = ct{1388};
t5dd = ct{1389};
t600 = ct{1390};
t601 = ct{1391};
t602 = ct{1392};
t604 = ct{1393};
t605 = ct{1394};
t608 = ct{1395};
t609 = ct{1396};
t61 = ct{1397};
t612 = ct{1398};
t614 = ct{1399};
t615 = ct{1400};
t616 = ct{1401};
t617 = ct{1402};
t623 = ct{1403};
t627 = ct{1404};
t63 = ct{1405};
t631 = ct{1406};
t632 = ct{1407};
t633 = ct{1408};
t634 = ct{1409};
t635 = ct{1410};
t636 = ct{1411};
t637 = ct{1412};
t639 = ct{1413};
t641 = ct{1414};
t642 = ct{1415};
t643 = ct{1416};
t644 = ct{1417};
t645 = ct{1418};
t646 = ct{1419};
t647 = ct{1420};
t648 = ct{1421};
t649 = ct{1422};
t650 = ct{1423};
t651 = ct{1424};
t652 = ct{1425};
t653 = ct{1426};
t654 = ct{1427};
t655 = ct{1428};
t658 = ct{1429};
t659 = ct{1430};
t660 = ct{1431};
t662 = ct{1432};
t663 = ct{1433};
t664 = ct{1434};
t665 = ct{1435};
t667 = ct{1436};
t668 = ct{1437};
t669 = ct{1438};
t670 = ct{1439};
t671 = ct{1440};
t673 = ct{1441};
t675 = ct{1442};
t680 = ct{1443};
t681 = ct{1444};
t682 = ct{1445};
t684 = ct{1446};
t685 = ct{1447};
t687 = ct{1448};
t689 = ct{1449};
t69 = ct{1450};
t690 = ct{1451};
t694 = ct{1452};
t695 = ct{1453};
t696 = ct{1454};
t698 = ct{1455};
t699 = ct{1456};
t6d = ct{1457};
t6dd = ct{1458};
t701 = ct{1459};
t702 = ct{1460};
t703 = ct{1461};
t705 = ct{1462};
t706 = ct{1463};
t71 = ct{1464};
t711 = ct{1465};
t712 = ct{1466};
t713 = ct{1467};
t714 = ct{1468};
t720 = ct{1469};
t721 = ct{1470};
t723 = ct{1471};
t724 = ct{1472};
t725 = ct{1473};
t726 = ct{1474};
t729 = ct{1475};
t731 = ct{1476};
t732 = ct{1477};
t733 = ct{1478};
t735 = ct{1479};
t736 = ct{1480};
t738 = ct{1481};
t739 = ct{1482};
t740 = ct{1483};
t742 = ct{1484};
t745 = ct{1485};
t746 = ct{1486};
t747 = ct{1487};
t748 = ct{1488};
t749 = ct{1489};
t75 = ct{1490};
t752 = ct{1491};
t755 = ct{1492};
t759 = ct{1493};
t760 = ct{1494};
t761 = ct{1495};
t763 = ct{1496};
t764 = ct{1497};
t772 = ct{1498};
t774 = ct{1499};
t775 = ct{1500};
t776 = ct{1501};
t780 = ct{1502};
t781 = ct{1503};
t782 = ct{1504};
t785 = ct{1505};
t788 = ct{1506};
t789 = ct{1507};
t793 = ct{1508};
t799 = ct{1509};
t8 = ct{1510};
t802 = ct{1511};
t805 = ct{1512};
t806 = ct{1513};
t807 = ct{1514};
t808 = ct{1515};
t817 = ct{1516};
t82 = ct{1517};
t820 = ct{1518};
t823 = ct{1519};
t824 = ct{1520};
t825 = ct{1521};
t826 = ct{1522};
t827 = ct{1523};
t828 = ct{1524};
t830 = ct{1525};
t831 = ct{1526};
t832 = ct{1527};
t833 = ct{1528};
t835 = ct{1529};
t836 = ct{1530};
t838 = ct{1531};
t842 = ct{1532};
t843 = ct{1533};
t844 = ct{1534};
t846 = ct{1535};
t848 = ct{1536};
t849 = ct{1537};
t850 = ct{1538};
t851 = ct{1539};
t852 = ct{1540};
t853 = ct{1541};
t854 = ct{1542};
t855 = ct{1543};
t859 = ct{1544};
t861 = ct{1545};
t865 = ct{1546};
t866 = ct{1547};
t869 = ct{1548};
t870 = ct{1549};
t871 = ct{1550};
t873 = ct{1551};
t874 = ct{1552};
t879 = ct{1553};
t88 = ct{1554};
t880 = ct{1555};
t882 = ct{1556};
t883 = ct{1557};
t884 = ct{1558};
t885 = ct{1559};
t887 = ct{1560};
t888 = ct{1561};
t889 = ct{1562};
t890 = ct{1563};
t891 = ct{1564};
t892 = ct{1565};
t895 = ct{1566};
t896 = ct{1567};
t897 = ct{1568};
t898 = ct{1569};
t899 = ct{1570};
t9 = ct{1571};
t900 = ct{1572};
t904 = ct{1573};
t907 = ct{1574};
t908 = ct{1575};
t909 = ct{1576};
t910 = ct{1577};
t911 = ct{1578};
t912 = ct{1579};
t915 = ct{1580};
t917 = ct{1581};
t919 = ct{1582};
t922 = ct{1583};
t923 = ct{1584};
t927 = ct{1585};
t928 = ct{1586};
t931 = ct{1587};
t932 = ct{1588};
t937 = ct{1589};
t938 = ct{1590};
t943 = ct{1591};
t944 = ct{1592};
t945 = ct{1593};
t952 = ct{1594};
t954 = ct{1595};
t955 = ct{1596};
t956 = ct{1597};
t959 = ct{1598};
t960 = ct{1599};
t961 = ct{1600};
t962 = ct{1601};
t963 = ct{1602};
t964 = ct{1603};
t965 = ct{1604};
t966 = ct{1605};
t968 = ct{1606};
t969 = ct{1607};
t970 = ct{1608};
t972 = ct{1609};
t973 = ct{1610};
t974 = ct{1611};
t975 = ct{1612};
t978 = ct{1613};
t979 = ct{1614};
t980 = ct{1615};
t981 = ct{1616};
t982 = ct{1617};
t983 = ct{1618};
t984 = ct{1619};
t985 = ct{1620};
t986 = ct{1621};
t987 = ct{1622};
t989 = ct{1623};
t992 = ct{1624};
t993 = ct{1625};
t994 = ct{1626};
t997 = ct{1627};
t999 = ct{1628};
t3949 = t8.*t2113.*t2658;
t3956 = (t14.*(t1070.*(t100-t364)+t330.*(t544-t1021+t330.*(t100-t364))))./2.0;
t3967 = -t8.*t37.*(t1070.*(t100-t364)+t330.*(t544-t1021+t330.*(t100-t364)));
t3970 = -t8.*t39.*(t1070.*(t100-t364)+t330.*(t544-t1021+t330.*(t100-t364)));
t3976 = t8.*t2140.*t2658;
t3987 = -t35.*t39.*(t1070.*(t100-t364)+t330.*(t544-t1021+t330.*(t100-t364)));
t3997 = t8.*t37.*(t1070.*(t100-t364)+t330.*(t544-t1021+t330.*(t100-t364))).*(-1.0./2.0);
t4004 = (t2169.*t2658)./2.0;
t4006 = t35.*t39.*(t1070.*(t100-t364)+t330.*(t544-t1021+t330.*(t100-t364)));
t4028 = t8.*t2279.*t2658;
t4050 = t2519+t2572;
t4058 = (t8.*t2357.*t2658)./2.0;
t4080 = -t2655.*(t859-t1704);
t4096 = t8.*t1807.*t3230;
t4103 = t8.*t1818.*t3230;
t4107 = t4098.*(-1.0./2.0);
t4112 = t4098./2.0;
t4125 = t1976.*t3230;
t4130 = t2662+t2671;
t4131 = t2663+t2672;
t4142 = t2169.*(t873-t2434).*(-1.0./2.0);
t4143 = -t4135;
t4149 = t4135./2.0;
t4153 = t4150.*(-1.0./2.0);
t4158 = t4150./2.0;
t4160 = t8.*t2113.*t3230;
t4165 = t2270.*(t503.*1.383e-1+t731+t981+t999);
t4166 = t2173.*t3230;
t4169 = t8.*t2140.*t3230;
t4170 = (t2666.*t2749)./2.0;
t4176 = (t2300.*t3083)./2.0;
t4177 = t909+t938+t1470+t2505;
t4178 = t874+t955+t1506+t2474;
t4221 = -t4207;
t4226 = t8.*t2279.*t3230;
t4231 = t4207./2.0;
t4256 = (t2749.*t2813)./2.0;
t4290 = (t8.*t2357.*t3230)./2.0;
t4309 = -t4299;
t4321 = t4299./2.0;
t4326 = -t2658.*(t873-t2434);
t4334 = t1463+t1495+t1750+t1769;
t4335 = t489+t869+t2315+t2458;
t4348 = t2270.*t3404;
t4353 = t467+t904+t2347+t2485;
t4379 = t2749.*t3083;
t4381 = t2658.*t3230;
t4389 = t2813.*t3083;
t4416 = (t2270.*t3686)./2.0;
t4470 = -t5d.*(t8.*(t729-t785-t806+t18.*t61.*(t101-t401))+t14.*(t752-t781-t838+t18.*t63.*(t100-t364)));
t4475 = t2270.*t3821;
t4486 = -t3230.*(t873-t2434);
t4541 = t4538.*2.0;
t4547 = -t4538;
t4556 = t4551.*2.0;
t4580 = -t2655.*(t855-t885-t1427+t1706);
t4589 = -t4579;
t4591 = t2655.*(t855-t885-t1427+t1706);
t4595 = t4579./2.0;
t4785 = t1910+t1937+t2393+t2395;
t4787 = -t2658.*(t870-t909-t1470+t2472);
t4801 = t2658.*(t870-t909-t1470+t2472).*(-1.0./2.0);
t4831 = t8.*t1807.*t4466;
t4858 = t931+t954+t956+t2063+t2127+t2133;
t4862 = t8.*t2113.*t4466;
t4881 = t8.*t2279.*t4466;
t4903 = t3230.*(t870-t909-t1470+t2472).*(-1.0./2.0);
t4908 = (t3230.*(t870-t909-t1470+t2472))./2.0;
t4931 = t2658.*t4466;
t4950 = t2298+t2318+t2560+t2565;
t4979 = -t4466.*(t873-t2434);
t4985 = t4466.*(t873-t2434);
t5006 = t3230.*t4466;
t691 = -t680;
t930 = t210+t590;
t947 = -t889;
t949 = t215+t605;
t967 = t882./2.0;
t976 = t888./2.0;
t977 = t889./2.0;
t1031 = t1013.*t1dd;
t1032 = t1020.*t1dd;
t1039 = -t1006;
t1042 = t1013.*2.0;
t1043 = t1020.*2.0;
t1044 = t455+t531;
t1060 = -t1009;
t1063 = -t1011;
t1064 = -t1014;
t1067 = -t1019;
t1072 = -t1026;
t1078 = t997./2.0;
t1083 = -t1049;
t1084 = -t1050;
t1088 = t1010./2.0;
t1090 = t1011./2.0;
t1091 = t1014./2.0;
t1095 = t1019./2.0;
t1100 = t1025./2.0;
t1101 = t1026./2.0;
t1109 = (t1009.*t1d)./2.0;
t1110 = (t1012.*t1d)./2.0;
t1120 = t35.*t1023;
t1124 = t38.*t1023;
t1145 = -t1073;
t1146 = -t1074;
t1147 = t1073.*-2.0;
t1148 = t1074.*-2.0;
t1181 = -t1159;
t1182 = -t1161;
t1191 = -t1119;
t1206 = t28.*t1074;
t1207 = t1111./2.0;
t1212 = t1119./2.0;
t1217 = t8.*t1126;
t1234 = t43+t1033;
t1239 = t1192.*t2d;
t1240 = t1192.*t3d;
t1241 = t1192.*t4d;
t1247 = -t1221;
t1259 = t1216.*t2d;
t1260 = t1216.*t3d;
t1271 = -t1231;
t1272 = -t1232;
t1273 = -t1233;
t1282 = t1218./2.0;
t1286 = t1220./2.0;
t1289 = t566+t631;
t1290 = t595+t604;
t1301 = t580+t600;
t1304 = -t1261;
t1308 = t1269.*t1d;
t1312 = t14.*t37.*t1126;
t1317 = t14.*t39.*t1126;
t1326 = t1261./2.0;
t1361 = -t1336;
t1367 = t1300./2.0;
t1377 = -t1328;
t1379 = -t1354;
t1395 = t1328./2.0;
t1408 = -t1390;
t1429 = -t37.*(t569-t604);
t1430 = t1374./2.0;
t1438 = -t1402;
t1447 = -t1407;
t1448 = -t1421;
t1449 = t18.*t39.*t1274;
t1457 = t1402./2.0;
t1460 = t1407./2.0;
t1465 = -t18.*t39.*(t569-t604);
t1473 = -t1456;
t1476 = -t1459;
t1480 = t37.*(t569-t604).*(-1.0./2.0);
t1484 = t1437./2.0;
t1487 = t1446./2.0;
t1514 = t18.*t39.*(t569-t604).*(-1.0./2.0);
t1539 = -t1509;
t1549 = t1508./2.0;
t1550 = t1509./2.0;
t1555 = t8.*t1525;
t1556 = t12.*t1525;
t1557 = t8.*t1528;
t1558 = t14.*t1525;
t1559 = t8.*t1529;
t1560 = t12.*t1528;
t1561 = t18.*t1525;
t1562 = t14.*t1528;
t1563 = t8.*t1533;
t1564 = t14.*t1529;
t1565 = t18.*t1528;
t1566 = t12.*t1533;
t1567 = t18.*t1529;
t1568 = t14.*t1533;
t1569 = -t1529;
t1571 = -t1533;
t1572 = -t1543;
t1573 = t18.*t1533.*t1dd;
t1578 = t12.*t1529.*2.0;
t1579 = t18.*t1533.*2.0;
t1581 = t1529./2.0;
t1582 = t1533./2.0;
t1597 = t34.*t1529;
t1598 = t255.*t1274;
t1600 = t34.*t1533;
t1601 = t35.*t1529;
t1602 = t36.*t1529;
t1603 = t35.*t1533;
t1604 = t36.*t1533;
t1605 = t38.*t1529;
t1609 = t38.*t1533;
t1626 = -t1580;
t1639 = t330.*t1274;
t1641 = -t1606;
t1643 = t1580./2.0;
t1647 = t1586./2.0;
t1648 = t1588./2.0;
t1649 = t1589./2.0;
t1654 = t1599./2.0;
t1656 = t18.*t37.*t1503;
t1658 = t12.*t39.*t1503;
t1660 = t1607./2.0;
t1662 = t18.*t39.*t1503;
t1663 = t698+t817;
t1664 = t341.*t1274;
t1671 = -t1644;
t1673 = t1615./2.0;
t1682 = t1625./2.0;
t1686 = t28.*t39.*t1528;
t1689 = t35.*t39.*t1503;
t1691 = t18.*t61.*t1503;
t1694 = t38.*t39.*t1503;
t1696 = t18.*t63.*t1503;
t1697 = -t1655;
t1698 = -t1657;
t1702 = t402.*t1274;
t1707 = -t1684;
t1716 = t1655./2.0;
t1718 = t1657./2.0;
t1720 = t1661./2.0;
t1735 = t1687.*t5d;
t1737 = t1692.*t5d;
t1738 = t740+t895;
t1763 = t1690./2.0;
t1765 = t1695./2.0;
t1785 = -t1743;
t1790 = t1726./2.0;
t1791 = t1727./2.0;
t1798 = t14.*t1742;
t1810 = -t1784;
t1813 = t1774./2.0;
t1821 = t255.*t1503;
t1822 = t256.*t1503;
t1824 = -t1794;
t1828 = t8.*t1786;
t1842 = t1800./2.0;
t1843 = t882+t883;
t1851 = t13.*t1819;
t1853 = t19.*t1819;
t1857 = t329.*t1503;
t1858 = t330.*t1503;
t1859 = -t1820;
t1864 = t609.*t1274;
t1873 = -t1830;
t1879 = t1815./2.0;
t1884 = -t1832;
t1887 = -t1835;
t1892 = t1826./2.0;
t1894 = t341.*t1503;
t1896 = t342.*t1503;
t1903 = t37.*t1776;
t1904 = t1830./2.0;
t1911 = t1832./2.0;
t1912 = t13.*t1856;
t1914 = t19.*t1856;
t1917 = -t1855;
t1923 = -t1862;
t1926 = -t1274.*(t100-t364);
t1929 = t641.*t1274;
t1936 = t1844./2.0;
t1943 = t1861./2.0;
t1945 = t1867./2.0;
t1948 = t402.*t1503;
t1950 = t403.*t1503;
t1951 = -t1893;
t1954 = t18.*t39.*t1776;
t1960 = -t1909;
t1967 = -t1920;
t1970 = -t1924;
t1974 = -t1274.*(t101-t401);
t1978 = t1893./2.0;
t1979 = t1895./2.0;
t1981 = t1947.*2.0;
t1986 = t1909./2.0;
t1987 = t1947.*t1dd;
t1991 = t453.*t1503;
t1992 = t1920./2.0;
t1993 = t1921./2.0;
t1997 = t459.*t1503;
t1998 = t1924./2.0;
t2009 = -t1985;
t2015 = t1949./2.0;
t2020 = t494.*t1503;
t2021 = t496.*t1503;
t2024 = -t1983;
t2029 = t499.*t1503;
t2031 = t1966./2.0;
t2033 = t502.*t1503;
t2042 = t1983./2.0;
t2053 = t542.*t1503;
t2054 = t543.*t1503;
t2057 = t544.*t1503;
t2072 = t2023./2.0;
t2073 = t1013+t1020;
t2083 = t593.*t1503;
t2095 = -t2068;
t2104 = t2060./2.0;
t2111 = t609.*t1503;
t2114 = -t2097;
t2125 = t2079./2.0;
t2126 = t2080./2.0;
t2146 = t2103./2.0;
t2151 = t1503.*(t100-t364).*-2.0;
t2152 = t641.*t1503.*2.0;
t2163 = t694.*t1503;
t2164 = t695.*t1503;
t2165 = t1503.*(t100-t364).*2.0;
t2166 = -t1503.*(t101-t401);
t2195 = t1130+t1131;
t2208 = -t2180;
t2209 = t2161./2.0;
t2213 = t1178+t1179;
t2220 = -t2193;
t2226 = t8.*t2171;
t2229 = t2180./2.0;
t2246 = t782.*t1503;
t2248 = t749.*t1503;
t2249 = t755.*t1503;
t2250 = t764.*t1503;
t2258 = t1153+t1199;
t2268 = t14.*t2204;
t2271 = -t2235;
t2274 = t2211./2.0;
t2278 = t2221./2.0;
t2284 = t2228./2.0;
t2287 = t836.*t1503;
t2288 = t2235./2.0;
t2291 = t802.*t1503;
t2293 = t805.*t1503;
t2295 = t808.*t1503;
t2297 = t1218+t1220;
t2304 = t2240./2.0;
t2305 = t2241./2.0;
t2306 = t775+t1525;
t2307 = -t2265;
t2308 = t776+t1528;
t2313 = t2243./2.0;
t2316 = t8.*t37.*t1503.*(t100-t364).*(-1.0./2.0);
t2319 = t2257./2.0;
t2320 = t2261./2.0;
t2324 = t8.*t2259;
t2325 = t2263./2.0;
t2326 = t2265./2.0;
t2330 = t892.*t1503;
t2332 = (t8.*t37.*t1503.*(t100-t364))./2.0;
t2355 = t18.*t37.*t2198;
t2356 = t12.*t39.*t2198;
t2358 = t18.*t39.*t2198;
t2361 = t1242+t1280;
t2367 = -t2339;
t2373 = t2363.*(-1.0./2.0);
t2375 = t35.*t39.*t2198;
t2376 = t18.*t61.*t2198;
t2377 = t38.*t39.*t2198;
t2378 = t18.*t63.*t2198;
t2384 = t2339./2.0;
t2387 = t2343./2.0;
t2418 = -t2379;
t2420 = t2365./2.0;
t2421 = t2366./2.0;
t2427 = t1016.*t1503;
t2429 = t1021.*t1503;
t2432 = t2379./2.0;
t2437 = t2389./2.0;
t2442 = -t2408;
t2443 = t1277+t1345;
t2444 = t1278+t1344;
t2449 = -t2417;
t2451 = t8.*t2390;
t2452 = t14.*t2391;
t2455 = t2402./2.0;
t2459 = t1065.*t1503;
t2463 = t1068.*t1503;
t2464 = t2439.*(-1.0./2.0);
t2476 = t1066.*t1503.*(-1.0./2.0);
t2479 = t2439./2.0;
t2486 = t2475.*(-1.0./2.0);
t2488 = t255.*t2198;
t2489 = t256.*t2198;
t2498 = -t2471;
t2499 = t2480.*t2dd;
t2500 = t2481.*t2dd;
t2501 = t2480.*t3dd;
t2502 = t2481.*t3dd;
t2503 = t2480.*t4dd;
t2504 = t2481.*t4dd;
t2517 = t2471./2.0;
t2525 = t329.*t2198;
t2526 = t330.*t2198;
t2531 = t8.*t37.*t2391;
t2532 = t14.*t37.*t2390;
t2533 = t8.*t39.*t2391;
t2534 = t14.*t39.*t2390;
t2535 = -t2497;
t2538 = t2520.*(-1.0./2.0);
t2543 = t342.*t2198;
t2546 = t2516.*t5d;
t2548 = t2497./2.0;
t2549 = t2520./2.0;
t2550 = t19.*t2523;
t2555 = -t2524;
t2558 = t341.*t2198.*2.0;
t2559 = t2515./2.0;
t2573 = t13.*t2523;
t2582 = t402.*t2198;
t2583 = t403.*t2198;
t2590 = t19.*t2554;
t2592 = -t2553;
t2604 = t13.*t2554;
t2607 = t453.*t2198;
t2609 = t459.*t2198;
t2610 = t742.*t1935;
t2620 = t2580./2.0;
t2621 = t2581./2.0;
t2625 = t496.*t2198;
t2629 = t499.*t2198;
t2632 = t502.*t2198;
t2636 = -t2623;
t2646 = t2611./2.0;
t2647 = t542.*t2198;
t2652 = t255.*t2390;
t2673 = t330.*t2391;
t2677 = t18.*t37.*t2578;
t2679 = t12.*t39.*t2578;
t2681 = t18.*t39.*t2578;
t2684 = t609.*t2198;
t2693 = t8.*t2654;
t2696 = t2664./2.0;
t2697 = t35.*t39.*t2578;
t2699 = t18.*t61.*t2578;
t2701 = t38.*t39.*t2578;
t2703 = t18.*t63.*t2578;
t2709 = -t2690;
t2713 = -t2694;
t2716 = t2198.*(t100-t364).*-2.0;
t2717 = t641.*t2198.*2.0;
t2720 = t8.*t2688;
t2721 = t2690./2.0;
t2722 = t1267+t1727;
t2728 = -t2198.*(t101-t401);
t2734 = t1370+t1661;
t2735 = t915+t984+t1023;
t2738 = t694.*t2198;
t2740 = t695.*t2198;
t2742 = t917+t985+t1024;
t2751 = t2198.*(t101-t401);
t2769 = t14.*t2741;
t2782 = t255.*t2578;
t2784 = t256.*t2578;
t2789 = t14.*t39.*t2688;
t2795 = t231+t394+t395+t1897;
t2797 = t755.*t2198;
t2803 = t8.*t2753;
t2808 = t782.*t2198;
t2817 = t13.*t2783;
t2819 = t19.*t2783;
t2820 = t1446+t1695;
t2821 = t329.*t2578;
t2823 = t330.*t2578;
t2829 = t805.*t2198;
t2830 = t808.*t2198;
t2836 = t341.*t2578;
t2837 = t342.*t2578;
t2842 = t836.*t2198;
t2854 = t13.*t2824;
t2856 = t19.*t2824;
t2857 = t8.*t39.*t2741;
t2865 = t2807./2.0;
t2866 = t8.*t37.*t2198.*(t100-t364).*(-1.0./2.0);
t2878 = t403.*t2578;
t2882 = -t2841;
t2884 = (t8.*t37.*t2198.*(t100-t364))./2.0;
t2891 = t14.*t39.*t2753;
t2895 = t402.*t2578.*2.0;
t2899 = t2841./2.0;
t2900 = t892.*t2198.*(-1.0./2.0);
t2911 = t453.*t2578;
t2913 = t459.*t2578;
t2920 = t1310+t1953;
t2921 = t1362+t1898;
t2932 = t2916.*(-1.0./2.0);
t2940 = t255.*t2688;
t2942 = t499.*t2578;
t2944 = t502.*t2578;
t2949 = t2916./2.0;
t2964 = t1318+t1988;
t2967 = -t2952;
t2969 = t548.*t2578;
t2974 = -t8.*(t1315-t1898);
t2976 = t2946.*t5dd;
t2977 = t2947.*t5dd;
t2982 = t2970.*(-1.0./2.0);
t2991 = t587.*t2578;
t3002 = t2992.*(-1.0./2.0);
t3005 = t8.*(t1315-t1898).*(-1.0./2.0);
t3010 = t2992./2.0;
t3011 = t330.*t2741;
t3015 = t255.*t2753;
t3016 = t609.*t2578.*2.0;
t3020 = t669.*t2578;
t3021 = -t2578.*(t100-t364);
Y = ft_6({t100,t1002,t1003,t1004,t1005,t1007,t1008,t1009,t101,t1010,t1012,t1014,t1015,t1016,t1017,t1018,t1019,t1021,t1022,t1025,t1026,t1028,t1029,t1030,t1031,t1032,t1034,t1035,t1036,t1038,t1039,t104,t1041,t1042,t1043,t1044,t1045,t1046,t1047,t1048,t1049,t1051,t1052,t1053,t1054,t1055,t1056,t1058,t1059,t106,t1060,t1062,t1063,t1064,t1066,t1067,t1068,t1069,t107,t1070,t1071,t1072,t1078,t1079,t108,t1080,t1082,t1083,t1084,t1085,t1086,t1087,t1088,t1089,t1090,t1091,t1092,t1093,t1094,t1095,t1096,t1097,t1098,t1099,t1100,t1101,t1106,t1108,t1109,t111,t1110,t1111,t1119,t112,t1120,t1121,t1122,t1123,t1124,t1125,t1126,t1128,t1129,t113,t1133,t1134,t1135,t1137,t1138,t1139,t1140,t1145,t1146,t1147,t1148,t1152,t1155,t1156,t1157,t1158,t1164,t1166,t1167,t1168,t1171,t1172,t1173,t1174,t1181,t1182,t1183,t1184,t1185,t1186,t1187,t1189,t1191,t1193,t1196,t1198,t12,t1201,t1202,t1203,t1204,t1205,t1206,t1207,t1208,t1209,t1210,t1211,t1212,t1217,t1219,t1222,t1224,t1225,t1226,t1227,t1229,t1230,t1234,t1235,t1236,t1237,t1238,t1239,t124,t1240,t1241,t1245,t1246,t1247,t1248,t1250,t1251,t1252,t1255,t1259,t1260,t1264,t1265,t1268,t1269,t127,t1270,t1271,t1272,t1273,t1274,t128,t1282,t1283,t1284,t1285,t1286,t1287,t1288,t1289,t1292,t1294,t1297,t1298,t13,t1300,t1301,t1302,t1304,t1306,t1307,t1308,t131,t1311,t1312,t1313,t1314,t1315,t1316,t1317,t132,t1321,t1323,t1324,t1325,t1326,t1328,t1329,t1330,t1331,t1332,t1333,t1334,t1335,t1336,t1337,t1338,t1339,t134,t1341,t1343,t1352,t1353,t1355,t1357,t1358,t136,t1360,t1361,t1366,t1367,t1368,t1369,t137,t1371,t1374,t1375,t1376,t1377,t1378,t1379,t138,t1382,t1383,t1387,t1389,t1391,t1392,t1393,t1395,t1396,t1398,t1399,t14,t1400,t1402,t1403,t1406,t1408,t1409,t1410,t1411,t1413,t1414,t1415,t1416,t1417,t1418,t1419,t1420,t1422,t1423,t1425,t1426,t1427,t1429,t1430,t1434,t1435,t1436,t1437,t1438,t1440,t1445,t1447,t1448,t1449,t1451,t1457,t1458,t1460,t1461,t1462,t1465,t1468,t1470,t1471,t1472,t1473,t1474,t1475,t1476,t1478,t1480,t1483,t1484,t1485,t1486,t1487,t1491,t1492,t1493,t1494,t1497,t1499,t15,t150,t1500,t1501,t1503,t1504,t1507,t1508,t1514,t1516,t1517,t1518,t1519,t152,t1520,t1521,t1523,t1524,t1525,t1527,t1528,t1529,t1531,t1532,t1534,t1535,t1536,t1537,t1538,t1539,t1545,t1546,t1547,t1549,t155,t1550,t1552,t1553,t1554,t1555,t1556,t1557,t1558,t1559,t156,t1560,t1561,t1562,t1563,t1564,t1565,t1566,t1567,t1568,t1569,t1571,t1572,t1574,t1578,t1579,t158,t1580,t1581,t1582,t1583,t1585,t1586,t1587,t1588,t1589,t159,t1590,t1591,t1593,t1594,t1597,t1598,t1599,t1600,t1601,t1602,t1603,t1604,t1605,t1606,t1607,t1609,t1610,t1615,t1616,t1618,t162,t1625,t1626,t1627,t1628,t163,t1630,t1631,t1632,t1633,t1634,t1635,t1636,t1637,t1639,t164,t1641,t1643,t1645,t1646,t1647,t1648,t1649,t165,t1650,t1651,t1652,t1653,t1654,t1656,t1657,t1658,t1659,t1660,t1662,t1663,t1664,t1666,t1667,t1668,t1669,t1670,t1671,t1672,t1673,t1674,t1675,t1676,t1677,t1678,t1680,t1682,t1683,t1686,t1687,t1688,t1689,t1690,t1691,t1692,t1693,t1694,t1696,t1697,t1698,t1699,t1701,t1702,t1704,t1706,t1707,t1708,t1709,t171,t1710,t1713,t1714,t1715,t1716,t1718,t1720,t1723,t1724,t1726,t173,t1733,t1735,t1736,t1737,t1738,t1739,t174,t1740,t1741,t1742,t1743,t1749,t175,t1751,t1752,t1754,t1755,t1756,t1758,t1759,t1761,t1762,t1763,t1765,t1768,t177,t1770,t1771,t1773,t1774,t1775,t1776,t1777,t1778,t1779,t1780,t1781,t1783,t1784,t1785,t1786,t1790,t1791,t1792,t1793,t1794,t1795,t1797,t1798,t1799,t18,t1800,t1801,t1805,t1806,t1807,t1808,t1809,t1810,t1813,t1814,t1815,t1816,t1818,t1819,t1821,t1822,t1824,t1825,t1826,t1827,t1828,t1829,t1830,t1832,t1834,t1835,t1837,t1840,t1842,t1843,t1844,t1845,t1846,t1848,t1851,t1853,t1856,t1857,t1858,t1859,t1862,t1863,t1864,t1865,t1866,t1867,t1868,t1869,t187,t1871,t1873,t1874,t1875,t1876,t1877,t1878,t1879,t1880,t1881,t1882,t1884,t1886,t1887,t1888,t1889,t1890,t1891,t1892,t1893,t1894,t1895,t1896,t1898,t19,t1903,t1904,t1905,t1907,t191,t1911,t1912,t1914,t1916,t1917,t1919,t1920,t1921,t1922,t1923,t1925,t1926,t1928,t1929,t1930,t1931,t1932,t1935,t1936,t1938,t1943,t1944,t1945,t1947,t1948,t1949,t1950,t1951,t1954,t1959,t196,t1960,t1961,t1962,t1963,t1965,t1966,t1967,t1968,t1969,t1970,t1971,t1972,t1973,t1974,t1976,t1977,t1978,t1979,t1981,t1983,t1984,t1985,t1986,t1987,t1988,t199,t1990,t1991,t1992,t1993,t1995,t1996,t1997,t1998,t1999,t1d,t1dd,t200,t2009,t201,t2015,t2017,t202,t2020,t2021,t2023,t2024,t2027,t2028,t2029,t2030,t2031,t2032,t2033,t2037,t2042,t2044,t2049,t2053,t2054,t2057,t2058,t2059,t206,t2060,t2061,t2064,t2067,t2068,t2070,t2072,t2073,t2074,t2075,t2078,t2079,t2080,t2081,t2082,t2083,t2085,t2086,t2087,t2090,t2091,t2092,t2093,t2094,t2095,t2096,t21,t2100,t2101,t2103,t2104,t2109,t2110,t2111,t2112,t2113,t2114,t2117,t2118,t2119,t2121,t2122,t2123,t2124,t2125,t2126,t2128,t2131,t2132,t2134,t2135,t2136,t2137,t2138,t2139,t2140,t2141,t2142,t2144,t2145,t2146,t2147,t215,t2150,t2152,t2153,t2155,t2156,t2159,t2160,t2161,t2162,t2163,t2164,t2165,t2166,t2167,t2168,t2169,t2170,t2171,t2172,t2173,t2174,t2177,t2178,t2180,t2181,t2183,t2184,t2189,t219,t2190,t2193,t2194,t2195,t2196,t2198,t2199,t22,t220,t2200,t2202,t2204,t2206,t2207,t2208,t2209,t221,t2210,t2212,t2213,t2216,t2219,t2220,t2221,t2222,t2225,t2226,t2227,t2228,t2229,t2233,t2235,t2240,t2241,t2243,t2244,t2245,t2246,t2247,t2249,t2250,t2256,t2257,t2259,t226,t2260,t2261,t2262,t2263,t2264,t2265,t2267,t2268,t2270,t2271,t2274,t2278,t2279,t2281,t2283,t2284,t2286,t2288,t229,t2291,t2292,t2293,t2294,t2295,t2297,t23,t2300,t2304,t2305,t2306,t2307,t2308,t2311,t2313,t2319,t232,t2320,t2323,t2324,t2325,t2326,t233,t2330,t2332,t2335,t2339,t2340,t2343,t2344,t2345,t2346,t2348,t2352,t2353,t2354,t2355,t2356,t2357,t2358,t2359,t2361,t2363,t2365,t2366,t2367,t2368,t2370,t2371,t2372,t2373,t2374,t2375,t2376,t2377,t2378,t2379,t2380,t2382,t2384,t2385,t2387,t2388,t2393,t2395,t2397,t2398,t2399,t24,t2400,t2401,t2402,t2403,t2405,t2406,t2407,t2409,t2410,t2412,t2413,t2414,t2416,t2418,t2420,t2421,t2423,t2424,t2426,t2427,t2428,t2429,t243,t2432,t2434,t2437,t2438,t2439,t244,t2440,t2441,t2442,t2443,t2444,t2447,t2448,t2449,t245,t2451,t2452,t2453,t2454,t2455,t2457,t2459,t2462,t2463,t2467,t247,t2471,t2472,t2473,t2475,t2476,t2477,t2478,t2479,t248,t2484,t2486,t2488,t2489,t249,t2490,t2497,t2498,t2499,t25,t2500,t2501,t2502,t2503,t2504,t2507,t2508,t2509,t2511,t2515,t2517,t2518,t2520,t2523,t2525,t2526,t2527,t2529,t2530,t2531,t2532,t2533,t2534,t2535,t2543,t2546,t2547,t2548,t2549,t255,t2550,t2554,t2555,t2557,t2558,t2559,t256,t2571,t2573,t2576,t2578,t258,t2580,t2581,t2582,t2583,t2590,t2592,t2593,t2599,t26,t2604,t2606,t2607,t2608,t2609,t2610,t2611,t2619,t2620,t2621,t2625,t2628,t2629,t2630,t2631,t2632,t2635,t2636,t2642,t2644,t2646,t2647,t2648,t2649,t2650,t2651,t2652,t2653,t2654,t2655,t2658,t2659,t2664,t2666,t2673,t2677,t2678,t2679,t2680,t2681,t2682,t2684,t2686,t2687,t2690,t2693,t2695,t2696,t2697,t2699,t27,t2701,t2702,t2703,t2704,t2705,t2708,t2709,t2711,t2713,t2715,t2716,t2717,t2718,t2719,t2720,t2721,t2722,t2723,t2724,t2727,t2729,t2731,t2734,t2736,t2737,t2738,t2739,t2740,t2743,t2744,t2745,t2747,t2749,t2750,t2751,t2755,t2760,t2761,t2762,t2764,t2765,t2766,t2768,t2769,t2772,t2775,t2776,t2777,t2779,t2780,t2781,t2782,t2783,t2784,t2789,t279,t2790,t2794,t2795,t2796,t2797,t2798,t2799,t28,t2803,t2807,t2808,t2813,t2817,t2819,t2820,t2821,t2823,t2824,t2826,t2829,t283,t2830,t2836,t2837,t2838,t2839,t2841,t2842,t2843,t2849,t2854,t2856,t2857,t2860,t2862,t2863,t2865,t2868,t2871,t2876,t2877,t2878,t2879,t2882,t2884,t2891,t2894,t2895,t2897,t2899,t29,t2900,t2901,t2911,t2912,t2913,t2914,t2915,t2916,t2919,t2920,t2925,t2927,t2929,t2934,t2936,t2937,t2940,t2942,t2944,t2946,t2947,t2949,t2951,t2953,t2954,t2956,t2959,t2966,t2967,t2969,t2970,t2971,t2974,t2976,t2977,t2978,t2979,t2982,t2983,t2985,t2989,t299,t2991,t2992,t2995,t2996,t2999,t2d,t2dd,t30,t3005,t3007,t3008,t301,t3010,t3011,t3012,t3013,t3014,t3015,t3016,t3018,t3020,t3021,t3023,t3028,t303,t3030,t3031,t3032,t3033,t3035,t3038,t3039,t3042,t3043,t3059,t3060,t3066,t3069,t3071,t3072,t3073,t3078,t3079,t308,t3080,t3082,t3083,t3086,t3087,t3088,t309,t3099,t31,t3101,t3102,t3103,t3122,t3123,t3125,t3129,t3130,t3148,t315,t3154,t3160,t3163,t3166,t3168,t3169,t317,t3175,t3176,t3177,t318,t3183,t3185,t319,t320,t3207,t321,t3214,t3230,t3232,t3234,t3237,t325,t3250,t3251,t3259,t3260,t3272,t3288,t3289,t329,t3291,t3292,t3298,t330,t3306,t3308,t331,t3318,t332,t3321,t333,t3330,t3331,t3332,t3335,t334,t3340,t3341,t3342,t3343,t3345,t3348,t3349,t3351,t3354,t3355,t3360,t3368,t3381,t3383,t3384,t3388,t3391,t3399,t34,t3400,t3401,t3404,t3405,t341,t3414,t3415,t3416,t342,t3421,t3429,t343,t3431,t3432,t3433,t3439,t344,t3440,t3445,t345,t3452,t3456,t3457,t3458,t3459,t346,t3460,t3461,t3466,t3467,t3468,t3469,t347,t3488,t3498,t35,t3500,t3504,t3509,t3510,t3513,t3516,t3517,t3523,t3531,t354,t3543,t3544,t3546,t3556,t3557,t3567,t3568,t3574,t3575,t3578,t3579,t3580,t3582,t3590,t3598,t36,t3601,t3606,t3612,t3617,t3622,t3628,t3630,t364,t3649,t365,t3674,t3678,t368,t3683,t3685,t3686,t3687,t3697,t37,t3701,t3704,t3712,t3716,t3721,t3724,t3734,t3741,t3743,t3744,t3745,t3747,t3750,t3751,t3758,t3761,t3768,t3769,t3770,t3771,t3779,t3785,t3786,t3792,t3796,t38,t3813,t3817,t3821,t3822,t3830,t384,t3840,t3843,t3846,t3852,t3853,t3871,t3872,t3875,t3877,t3878,t3897,t39,t3903,t3906,t3907,t392,t3923,t393,t3940,t3941,t3943,t3949,t3956,t3967,t3976,t3997,t3d,t3dd,t4004,t4006,t401,t402,t4025,t4028,t403,t404,t4050,t4058,t4059,t4069,t4071,t4075,t4076,t4080,t4084,t4086,t4096,t4098,t41,t410,t4103,t411,t4112,t412,t4125,t4126,t4129,t413,t4130,t4131,t4133,t4134,t4139,t414,t4140,t4142,t4143,t4144,t4146,t4147,t4149,t415,t4150,t4152,t4157,t4158,t4159,t416,t4160,t4165,t4166,t4169,t4170,t4172,t4176,t4178,t418,t419,t42,t420,t4203,t4212,t4221,t4226,t4230,t4231,t4236,t425,t4256,t4290,t4299,t4304,t4309,t431,t4321,t4325,t4326,t4332,t4334,t4335,t434,t4348,t4353,t437,t4379,t4381,t4389,t441,t4416,t442,t443,t444,t446,t4470,t4475,t4486,t453,t4538,t454,t4541,t4547,t4551,t4556,t4579,t459,t4591,t4595,t470,t478,t4785,t4787,t48,t4801,t483,t4831,t484,t4858,t486,t4862,t487,t488,t4881,t4908,t492,t493,t4931,t494,t495,t4950,t496,t497,t4979,t498,t4985,t4d,t4dd,t50,t5006,t501,t503,t508,t51,t514,t515,t516,t519,t523,t524,t529,t53,t530,t532,t537,t543,t544,t546,t547,t548,t549,t55,t550,t552,t553,t554,t56,t562,t569,t57,t570,t58,t582,t588,t589,t591,t593,t596,t598,t5d,t5dd,t601,t602,t604,t608,t609,t61,t612,t614,t615,t616,t617,t623,t627,t63,t632,t633,t634,t635,t636,t637,t639,t641,t642,t643,t644,t645,t646,t647,t648,t649,t650,t651,t652,t653,t654,t655,t658,t659,t660,t662,t663,t664,t665,t667,t668,t670,t671,t673,t675,t680,t681,t682,t684,t685,t687,t689,t69,t690,t691,t694,t695,t696,t698,t699,t6d,t6dd,t701,t702,t703,t705,t706,t71,t711,t712,t713,t714,t720,t721,t723,t724,t725,t726,t729,t731,t732,t733,t735,t736,t738,t739,t742,t745,t746,t747,t748,t75,t752,t755,t759,t760,t761,t763,t764,t772,t774,t775,t776,t780,t781,t782,t785,t788,t789,t793,t799,t8,t802,t805,t806,t807,t808,t82,t820,t823,t824,t825,t826,t827,t828,t830,t831,t832,t833,t835,t838,t842,t843,t844,t846,t848,t849,t850,t851,t852,t853,t854,t855,t859,t861,t865,t866,t870,t871,t873,t879,t88,t880,t884,t885,t887,t888,t890,t891,t892,t896,t897,t898,t899,t9,t900,t907,t908,t909,t910,t911,t912,t915,t917,t919,t922,t923,t927,t928,t930,t932,t937,t943,t944,t945,t947,t949,t952,t959,t960,t961,t962,t963,t964,t965,t966,t967,t968,t969,t970,t972,t973,t974,t975,t976,t977,t978,t979,t980,t981,t982,t983,t986,t987,t989,t992,t993,t994,t997,t999});
end
function Y = ft_6(ct)
t100 = ct{1};
t1002 = ct{2};
t1003 = ct{3};
t1004 = ct{4};
t1005 = ct{5};
t1007 = ct{6};
t1008 = ct{7};
t1009 = ct{8};
t101 = ct{9};
t1010 = ct{10};
t1012 = ct{11};
t1014 = ct{12};
t1015 = ct{13};
t1016 = ct{14};
t1017 = ct{15};
t1018 = ct{16};
t1019 = ct{17};
t1021 = ct{18};
t1022 = ct{19};
t1025 = ct{20};
t1026 = ct{21};
t1028 = ct{22};
t1029 = ct{23};
t1030 = ct{24};
t1031 = ct{25};
t1032 = ct{26};
t1034 = ct{27};
t1035 = ct{28};
t1036 = ct{29};
t1038 = ct{30};
t1039 = ct{31};
t104 = ct{32};
t1041 = ct{33};
t1042 = ct{34};
t1043 = ct{35};
t1044 = ct{36};
t1045 = ct{37};
t1046 = ct{38};
t1047 = ct{39};
t1048 = ct{40};
t1049 = ct{41};
t1051 = ct{42};
t1052 = ct{43};
t1053 = ct{44};
t1054 = ct{45};
t1055 = ct{46};
t1056 = ct{47};
t1058 = ct{48};
t1059 = ct{49};
t106 = ct{50};
t1060 = ct{51};
t1062 = ct{52};
t1063 = ct{53};
t1064 = ct{54};
t1066 = ct{55};
t1067 = ct{56};
t1068 = ct{57};
t1069 = ct{58};
t107 = ct{59};
t1070 = ct{60};
t1071 = ct{61};
t1072 = ct{62};
t1078 = ct{63};
t1079 = ct{64};
t108 = ct{65};
t1080 = ct{66};
t1082 = ct{67};
t1083 = ct{68};
t1084 = ct{69};
t1085 = ct{70};
t1086 = ct{71};
t1087 = ct{72};
t1088 = ct{73};
t1089 = ct{74};
t1090 = ct{75};
t1091 = ct{76};
t1092 = ct{77};
t1093 = ct{78};
t1094 = ct{79};
t1095 = ct{80};
t1096 = ct{81};
t1097 = ct{82};
t1098 = ct{83};
t1099 = ct{84};
t1100 = ct{85};
t1101 = ct{86};
t1106 = ct{87};
t1108 = ct{88};
t1109 = ct{89};
t111 = ct{90};
t1110 = ct{91};
t1111 = ct{92};
t1119 = ct{93};
t112 = ct{94};
t1120 = ct{95};
t1121 = ct{96};
t1122 = ct{97};
t1123 = ct{98};
t1124 = ct{99};
t1125 = ct{100};
t1126 = ct{101};
t1128 = ct{102};
t1129 = ct{103};
t113 = ct{104};
t1133 = ct{105};
t1134 = ct{106};
t1135 = ct{107};
t1137 = ct{108};
t1138 = ct{109};
t1139 = ct{110};
t1140 = ct{111};
t1145 = ct{112};
t1146 = ct{113};
t1147 = ct{114};
t1148 = ct{115};
t1152 = ct{116};
t1155 = ct{117};
t1156 = ct{118};
t1157 = ct{119};
t1158 = ct{120};
t1164 = ct{121};
t1166 = ct{122};
t1167 = ct{123};
t1168 = ct{124};
t1171 = ct{125};
t1172 = ct{126};
t1173 = ct{127};
t1174 = ct{128};
t1181 = ct{129};
t1182 = ct{130};
t1183 = ct{131};
t1184 = ct{132};
t1185 = ct{133};
t1186 = ct{134};
t1187 = ct{135};
t1189 = ct{136};
t1191 = ct{137};
t1193 = ct{138};
t1196 = ct{139};
t1198 = ct{140};
t12 = ct{141};
t1201 = ct{142};
t1202 = ct{143};
t1203 = ct{144};
t1204 = ct{145};
t1205 = ct{146};
t1206 = ct{147};
t1207 = ct{148};
t1208 = ct{149};
t1209 = ct{150};
t1210 = ct{151};
t1211 = ct{152};
t1212 = ct{153};
t1217 = ct{154};
t1219 = ct{155};
t1222 = ct{156};
t1224 = ct{157};
t1225 = ct{158};
t1226 = ct{159};
t1227 = ct{160};
t1229 = ct{161};
t1230 = ct{162};
t1234 = ct{163};
t1235 = ct{164};
t1236 = ct{165};
t1237 = ct{166};
t1238 = ct{167};
t1239 = ct{168};
t124 = ct{169};
t1240 = ct{170};
t1241 = ct{171};
t1245 = ct{172};
t1246 = ct{173};
t1247 = ct{174};
t1248 = ct{175};
t1250 = ct{176};
t1251 = ct{177};
t1252 = ct{178};
t1255 = ct{179};
t1259 = ct{180};
t1260 = ct{181};
t1264 = ct{182};
t1265 = ct{183};
t1268 = ct{184};
t1269 = ct{185};
t127 = ct{186};
t1270 = ct{187};
t1271 = ct{188};
t1272 = ct{189};
t1273 = ct{190};
t1274 = ct{191};
t128 = ct{192};
t1282 = ct{193};
t1283 = ct{194};
t1284 = ct{195};
t1285 = ct{196};
t1286 = ct{197};
t1287 = ct{198};
t1288 = ct{199};
t1289 = ct{200};
t1292 = ct{201};
t1294 = ct{202};
t1297 = ct{203};
t1298 = ct{204};
t13 = ct{205};
t1300 = ct{206};
t1301 = ct{207};
t1302 = ct{208};
t1304 = ct{209};
t1306 = ct{210};
t1307 = ct{211};
t1308 = ct{212};
t131 = ct{213};
t1311 = ct{214};
t1312 = ct{215};
t1313 = ct{216};
t1314 = ct{217};
t1315 = ct{218};
t1316 = ct{219};
t1317 = ct{220};
t132 = ct{221};
t1321 = ct{222};
t1323 = ct{223};
t1324 = ct{224};
t1325 = ct{225};
t1326 = ct{226};
t1328 = ct{227};
t1329 = ct{228};
t1330 = ct{229};
t1331 = ct{230};
t1332 = ct{231};
t1333 = ct{232};
t1334 = ct{233};
t1335 = ct{234};
t1336 = ct{235};
t1337 = ct{236};
t1338 = ct{237};
t1339 = ct{238};
t134 = ct{239};
t1341 = ct{240};
t1343 = ct{241};
t1352 = ct{242};
t1353 = ct{243};
t1355 = ct{244};
t1357 = ct{245};
t1358 = ct{246};
t136 = ct{247};
t1360 = ct{248};
t1361 = ct{249};
t1366 = ct{250};
t1367 = ct{251};
t1368 = ct{252};
t1369 = ct{253};
t137 = ct{254};
t1371 = ct{255};
t1374 = ct{256};
t1375 = ct{257};
t1376 = ct{258};
t1377 = ct{259};
t1378 = ct{260};
t1379 = ct{261};
t138 = ct{262};
t1382 = ct{263};
t1383 = ct{264};
t1387 = ct{265};
t1389 = ct{266};
t1391 = ct{267};
t1392 = ct{268};
t1393 = ct{269};
t1395 = ct{270};
t1396 = ct{271};
t1398 = ct{272};
t1399 = ct{273};
t14 = ct{274};
t1400 = ct{275};
t1402 = ct{276};
t1403 = ct{277};
t1406 = ct{278};
t1408 = ct{279};
t1409 = ct{280};
t1410 = ct{281};
t1411 = ct{282};
t1413 = ct{283};
t1414 = ct{284};
t1415 = ct{285};
t1416 = ct{286};
t1417 = ct{287};
t1418 = ct{288};
t1419 = ct{289};
t1420 = ct{290};
t1422 = ct{291};
t1423 = ct{292};
t1425 = ct{293};
t1426 = ct{294};
t1427 = ct{295};
t1429 = ct{296};
t1430 = ct{297};
t1434 = ct{298};
t1435 = ct{299};
t1436 = ct{300};
t1437 = ct{301};
t1438 = ct{302};
t1440 = ct{303};
t1445 = ct{304};
t1447 = ct{305};
t1448 = ct{306};
t1449 = ct{307};
t1451 = ct{308};
t1457 = ct{309};
t1458 = ct{310};
t1460 = ct{311};
t1461 = ct{312};
t1462 = ct{313};
t1465 = ct{314};
t1468 = ct{315};
t1470 = ct{316};
t1471 = ct{317};
t1472 = ct{318};
t1473 = ct{319};
t1474 = ct{320};
t1475 = ct{321};
t1476 = ct{322};
t1478 = ct{323};
t1480 = ct{324};
t1483 = ct{325};
t1484 = ct{326};
t1485 = ct{327};
t1486 = ct{328};
t1487 = ct{329};
t1491 = ct{330};
t1492 = ct{331};
t1493 = ct{332};
t1494 = ct{333};
t1497 = ct{334};
t1499 = ct{335};
t15 = ct{336};
t150 = ct{337};
t1500 = ct{338};
t1501 = ct{339};
t1503 = ct{340};
t1504 = ct{341};
t1507 = ct{342};
t1508 = ct{343};
t1514 = ct{344};
t1516 = ct{345};
t1517 = ct{346};
t1518 = ct{347};
t1519 = ct{348};
t152 = ct{349};
t1520 = ct{350};
t1521 = ct{351};
t1523 = ct{352};
t1524 = ct{353};
t1525 = ct{354};
t1527 = ct{355};
t1528 = ct{356};
t1529 = ct{357};
t1531 = ct{358};
t1532 = ct{359};
t1534 = ct{360};
t1535 = ct{361};
t1536 = ct{362};
t1537 = ct{363};
t1538 = ct{364};
t1539 = ct{365};
t1545 = ct{366};
t1546 = ct{367};
t1547 = ct{368};
t1549 = ct{369};
t155 = ct{370};
t1550 = ct{371};
t1552 = ct{372};
t1553 = ct{373};
t1554 = ct{374};
t1555 = ct{375};
t1556 = ct{376};
t1557 = ct{377};
t1558 = ct{378};
t1559 = ct{379};
t156 = ct{380};
t1560 = ct{381};
t1561 = ct{382};
t1562 = ct{383};
t1563 = ct{384};
t1564 = ct{385};
t1565 = ct{386};
t1566 = ct{387};
t1567 = ct{388};
t1568 = ct{389};
t1569 = ct{390};
t1571 = ct{391};
t1572 = ct{392};
t1574 = ct{393};
t1578 = ct{394};
t1579 = ct{395};
t158 = ct{396};
t1580 = ct{397};
t1581 = ct{398};
t1582 = ct{399};
t1583 = ct{400};
t1585 = ct{401};
t1586 = ct{402};
t1587 = ct{403};
t1588 = ct{404};
t1589 = ct{405};
t159 = ct{406};
t1590 = ct{407};
t1591 = ct{408};
t1593 = ct{409};
t1594 = ct{410};
t1597 = ct{411};
t1598 = ct{412};
t1599 = ct{413};
t1600 = ct{414};
t1601 = ct{415};
t1602 = ct{416};
t1603 = ct{417};
t1604 = ct{418};
t1605 = ct{419};
t1606 = ct{420};
t1607 = ct{421};
t1609 = ct{422};
t1610 = ct{423};
t1615 = ct{424};
t1616 = ct{425};
t1618 = ct{426};
t162 = ct{427};
t1625 = ct{428};
t1626 = ct{429};
t1627 = ct{430};
t1628 = ct{431};
t163 = ct{432};
t1630 = ct{433};
t1631 = ct{434};
t1632 = ct{435};
t1633 = ct{436};
t1634 = ct{437};
t1635 = ct{438};
t1636 = ct{439};
t1637 = ct{440};
t1639 = ct{441};
t164 = ct{442};
t1641 = ct{443};
t1643 = ct{444};
t1645 = ct{445};
t1646 = ct{446};
t1647 = ct{447};
t1648 = ct{448};
t1649 = ct{449};
t165 = ct{450};
t1650 = ct{451};
t1651 = ct{452};
t1652 = ct{453};
t1653 = ct{454};
t1654 = ct{455};
t1656 = ct{456};
t1657 = ct{457};
t1658 = ct{458};
t1659 = ct{459};
t1660 = ct{460};
t1662 = ct{461};
t1663 = ct{462};
t1664 = ct{463};
t1666 = ct{464};
t1667 = ct{465};
t1668 = ct{466};
t1669 = ct{467};
t1670 = ct{468};
t1671 = ct{469};
t1672 = ct{470};
t1673 = ct{471};
t1674 = ct{472};
t1675 = ct{473};
t1676 = ct{474};
t1677 = ct{475};
t1678 = ct{476};
t1680 = ct{477};
t1682 = ct{478};
t1683 = ct{479};
t1686 = ct{480};
t1687 = ct{481};
t1688 = ct{482};
t1689 = ct{483};
t1690 = ct{484};
t1691 = ct{485};
t1692 = ct{486};
t1693 = ct{487};
t1694 = ct{488};
t1696 = ct{489};
t1697 = ct{490};
t1698 = ct{491};
t1699 = ct{492};
t1701 = ct{493};
t1702 = ct{494};
t1704 = ct{495};
t1706 = ct{496};
t1707 = ct{497};
t1708 = ct{498};
t1709 = ct{499};
t171 = ct{500};
t1710 = ct{501};
t1713 = ct{502};
t1714 = ct{503};
t1715 = ct{504};
t1716 = ct{505};
t1718 = ct{506};
t1720 = ct{507};
t1723 = ct{508};
t1724 = ct{509};
t1726 = ct{510};
t173 = ct{511};
t1733 = ct{512};
t1735 = ct{513};
t1736 = ct{514};
t1737 = ct{515};
t1738 = ct{516};
t1739 = ct{517};
t174 = ct{518};
t1740 = ct{519};
t1741 = ct{520};
t1742 = ct{521};
t1743 = ct{522};
t1749 = ct{523};
t175 = ct{524};
t1751 = ct{525};
t1752 = ct{526};
t1754 = ct{527};
t1755 = ct{528};
t1756 = ct{529};
t1758 = ct{530};
t1759 = ct{531};
t1761 = ct{532};
t1762 = ct{533};
t1763 = ct{534};
t1765 = ct{535};
t1768 = ct{536};
t177 = ct{537};
t1770 = ct{538};
t1771 = ct{539};
t1773 = ct{540};
t1774 = ct{541};
t1775 = ct{542};
t1776 = ct{543};
t1777 = ct{544};
t1778 = ct{545};
t1779 = ct{546};
t1780 = ct{547};
t1781 = ct{548};
t1783 = ct{549};
t1784 = ct{550};
t1785 = ct{551};
t1786 = ct{552};
t1790 = ct{553};
t1791 = ct{554};
t1792 = ct{555};
t1793 = ct{556};
t1794 = ct{557};
t1795 = ct{558};
t1797 = ct{559};
t1798 = ct{560};
t1799 = ct{561};
t18 = ct{562};
t1800 = ct{563};
t1801 = ct{564};
t1805 = ct{565};
t1806 = ct{566};
t1807 = ct{567};
t1808 = ct{568};
t1809 = ct{569};
t1810 = ct{570};
t1813 = ct{571};
t1814 = ct{572};
t1815 = ct{573};
t1816 = ct{574};
t1818 = ct{575};
t1819 = ct{576};
t1821 = ct{577};
t1822 = ct{578};
t1824 = ct{579};
t1825 = ct{580};
t1826 = ct{581};
t1827 = ct{582};
t1828 = ct{583};
t1829 = ct{584};
t1830 = ct{585};
t1832 = ct{586};
t1834 = ct{587};
t1835 = ct{588};
t1837 = ct{589};
t1840 = ct{590};
t1842 = ct{591};
t1843 = ct{592};
t1844 = ct{593};
t1845 = ct{594};
t1846 = ct{595};
t1848 = ct{596};
t1851 = ct{597};
t1853 = ct{598};
t1856 = ct{599};
t1857 = ct{600};
t1858 = ct{601};
t1859 = ct{602};
t1862 = ct{603};
t1863 = ct{604};
t1864 = ct{605};
t1865 = ct{606};
t1866 = ct{607};
t1867 = ct{608};
t1868 = ct{609};
t1869 = ct{610};
t187 = ct{611};
t1871 = ct{612};
t1873 = ct{613};
t1874 = ct{614};
t1875 = ct{615};
t1876 = ct{616};
t1877 = ct{617};
t1878 = ct{618};
t1879 = ct{619};
t1880 = ct{620};
t1881 = ct{621};
t1882 = ct{622};
t1884 = ct{623};
t1886 = ct{624};
t1887 = ct{625};
t1888 = ct{626};
t1889 = ct{627};
t1890 = ct{628};
t1891 = ct{629};
t1892 = ct{630};
t1893 = ct{631};
t1894 = ct{632};
t1895 = ct{633};
t1896 = ct{634};
t1898 = ct{635};
t19 = ct{636};
t1903 = ct{637};
t1904 = ct{638};
t1905 = ct{639};
t1907 = ct{640};
t191 = ct{641};
t1911 = ct{642};
t1912 = ct{643};
t1914 = ct{644};
t1916 = ct{645};
t1917 = ct{646};
t1919 = ct{647};
t1920 = ct{648};
t1921 = ct{649};
t1922 = ct{650};
t1923 = ct{651};
t1925 = ct{652};
t1926 = ct{653};
t1928 = ct{654};
t1929 = ct{655};
t1930 = ct{656};
t1931 = ct{657};
t1932 = ct{658};
t1935 = ct{659};
t1936 = ct{660};
t1938 = ct{661};
t1943 = ct{662};
t1944 = ct{663};
t1945 = ct{664};
t1947 = ct{665};
t1948 = ct{666};
t1949 = ct{667};
t1950 = ct{668};
t1951 = ct{669};
t1954 = ct{670};
t1959 = ct{671};
t196 = ct{672};
t1960 = ct{673};
t1961 = ct{674};
t1962 = ct{675};
t1963 = ct{676};
t1965 = ct{677};
t1966 = ct{678};
t1967 = ct{679};
t1968 = ct{680};
t1969 = ct{681};
t1970 = ct{682};
t1971 = ct{683};
t1972 = ct{684};
t1973 = ct{685};
t1974 = ct{686};
t1976 = ct{687};
t1977 = ct{688};
t1978 = ct{689};
t1979 = ct{690};
t1981 = ct{691};
t1983 = ct{692};
t1984 = ct{693};
t1985 = ct{694};
t1986 = ct{695};
t1987 = ct{696};
t1988 = ct{697};
t199 = ct{698};
t1990 = ct{699};
t1991 = ct{700};
t1992 = ct{701};
t1993 = ct{702};
t1995 = ct{703};
t1996 = ct{704};
t1997 = ct{705};
t1998 = ct{706};
t1999 = ct{707};
t1d = ct{708};
t1dd = ct{709};
t200 = ct{710};
t2009 = ct{711};
t201 = ct{712};
t2015 = ct{713};
t2017 = ct{714};
t202 = ct{715};
t2020 = ct{716};
t2021 = ct{717};
t2023 = ct{718};
t2024 = ct{719};
t2027 = ct{720};
t2028 = ct{721};
t2029 = ct{722};
t2030 = ct{723};
t2031 = ct{724};
t2032 = ct{725};
t2033 = ct{726};
t2037 = ct{727};
t2042 = ct{728};
t2044 = ct{729};
t2049 = ct{730};
t2053 = ct{731};
t2054 = ct{732};
t2057 = ct{733};
t2058 = ct{734};
t2059 = ct{735};
t206 = ct{736};
t2060 = ct{737};
t2061 = ct{738};
t2064 = ct{739};
t2067 = ct{740};
t2068 = ct{741};
t2070 = ct{742};
t2072 = ct{743};
t2073 = ct{744};
t2074 = ct{745};
t2075 = ct{746};
t2078 = ct{747};
t2079 = ct{748};
t2080 = ct{749};
t2081 = ct{750};
t2082 = ct{751};
t2083 = ct{752};
t2085 = ct{753};
t2086 = ct{754};
t2087 = ct{755};
t2090 = ct{756};
t2091 = ct{757};
t2092 = ct{758};
t2093 = ct{759};
t2094 = ct{760};
t2095 = ct{761};
t2096 = ct{762};
t21 = ct{763};
t2100 = ct{764};
t2101 = ct{765};
t2103 = ct{766};
t2104 = ct{767};
t2109 = ct{768};
t2110 = ct{769};
t2111 = ct{770};
t2112 = ct{771};
t2113 = ct{772};
t2114 = ct{773};
t2117 = ct{774};
t2118 = ct{775};
t2119 = ct{776};
t2121 = ct{777};
t2122 = ct{778};
t2123 = ct{779};
t2124 = ct{780};
t2125 = ct{781};
t2126 = ct{782};
t2128 = ct{783};
t2131 = ct{784};
t2132 = ct{785};
t2134 = ct{786};
t2135 = ct{787};
t2136 = ct{788};
t2137 = ct{789};
t2138 = ct{790};
t2139 = ct{791};
t2140 = ct{792};
t2141 = ct{793};
t2142 = ct{794};
t2144 = ct{795};
t2145 = ct{796};
t2146 = ct{797};
t2147 = ct{798};
t215 = ct{799};
t2150 = ct{800};
t2152 = ct{801};
t2153 = ct{802};
t2155 = ct{803};
t2156 = ct{804};
t2159 = ct{805};
t2160 = ct{806};
t2161 = ct{807};
t2162 = ct{808};
t2163 = ct{809};
t2164 = ct{810};
t2165 = ct{811};
t2166 = ct{812};
t2167 = ct{813};
t2168 = ct{814};
t2169 = ct{815};
t2170 = ct{816};
t2171 = ct{817};
t2172 = ct{818};
t2173 = ct{819};
t2174 = ct{820};
t2177 = ct{821};
t2178 = ct{822};
t2180 = ct{823};
t2181 = ct{824};
t2183 = ct{825};
t2184 = ct{826};
t2189 = ct{827};
t219 = ct{828};
t2190 = ct{829};
t2193 = ct{830};
t2194 = ct{831};
t2195 = ct{832};
t2196 = ct{833};
t2198 = ct{834};
t2199 = ct{835};
t22 = ct{836};
t220 = ct{837};
t2200 = ct{838};
t2202 = ct{839};
t2204 = ct{840};
t2206 = ct{841};
t2207 = ct{842};
t2208 = ct{843};
t2209 = ct{844};
t221 = ct{845};
t2210 = ct{846};
t2212 = ct{847};
t2213 = ct{848};
t2216 = ct{849};
t2219 = ct{850};
t2220 = ct{851};
t2221 = ct{852};
t2222 = ct{853};
t2225 = ct{854};
t2226 = ct{855};
t2227 = ct{856};
t2228 = ct{857};
t2229 = ct{858};
t2233 = ct{859};
t2235 = ct{860};
t2240 = ct{861};
t2241 = ct{862};
t2243 = ct{863};
t2244 = ct{864};
t2245 = ct{865};
t2246 = ct{866};
t2247 = ct{867};
t2249 = ct{868};
t2250 = ct{869};
t2256 = ct{870};
t2257 = ct{871};
t2259 = ct{872};
t226 = ct{873};
t2260 = ct{874};
t2261 = ct{875};
t2262 = ct{876};
t2263 = ct{877};
t2264 = ct{878};
t2265 = ct{879};
t2267 = ct{880};
t2268 = ct{881};
t2270 = ct{882};
t2271 = ct{883};
t2274 = ct{884};
t2278 = ct{885};
t2279 = ct{886};
t2281 = ct{887};
t2283 = ct{888};
t2284 = ct{889};
t2286 = ct{890};
t2288 = ct{891};
t229 = ct{892};
t2291 = ct{893};
t2292 = ct{894};
t2293 = ct{895};
t2294 = ct{896};
t2295 = ct{897};
t2297 = ct{898};
t23 = ct{899};
t2300 = ct{900};
t2304 = ct{901};
t2305 = ct{902};
t2306 = ct{903};
t2307 = ct{904};
t2308 = ct{905};
t2311 = ct{906};
t2313 = ct{907};
t2319 = ct{908};
t232 = ct{909};
t2320 = ct{910};
t2323 = ct{911};
t2324 = ct{912};
t2325 = ct{913};
t2326 = ct{914};
t233 = ct{915};
t2330 = ct{916};
t2332 = ct{917};
t2335 = ct{918};
t2339 = ct{919};
t2340 = ct{920};
t2343 = ct{921};
t2344 = ct{922};
t2345 = ct{923};
t2346 = ct{924};
t2348 = ct{925};
t2352 = ct{926};
t2353 = ct{927};
t2354 = ct{928};
t2355 = ct{929};
t2356 = ct{930};
t2357 = ct{931};
t2358 = ct{932};
t2359 = ct{933};
t2361 = ct{934};
t2363 = ct{935};
t2365 = ct{936};
t2366 = ct{937};
t2367 = ct{938};
t2368 = ct{939};
t2370 = ct{940};
t2371 = ct{941};
t2372 = ct{942};
t2373 = ct{943};
t2374 = ct{944};
t2375 = ct{945};
t2376 = ct{946};
t2377 = ct{947};
t2378 = ct{948};
t2379 = ct{949};
t2380 = ct{950};
t2382 = ct{951};
t2384 = ct{952};
t2385 = ct{953};
t2387 = ct{954};
t2388 = ct{955};
t2393 = ct{956};
t2395 = ct{957};
t2397 = ct{958};
t2398 = ct{959};
t2399 = ct{960};
t24 = ct{961};
t2400 = ct{962};
t2401 = ct{963};
t2402 = ct{964};
t2403 = ct{965};
t2405 = ct{966};
t2406 = ct{967};
t2407 = ct{968};
t2409 = ct{969};
t2410 = ct{970};
t2412 = ct{971};
t2413 = ct{972};
t2414 = ct{973};
t2416 = ct{974};
t2418 = ct{975};
t2420 = ct{976};
t2421 = ct{977};
t2423 = ct{978};
t2424 = ct{979};
t2426 = ct{980};
t2427 = ct{981};
t2428 = ct{982};
t2429 = ct{983};
t243 = ct{984};
t2432 = ct{985};
t2434 = ct{986};
t2437 = ct{987};
t2438 = ct{988};
t2439 = ct{989};
t244 = ct{990};
t2440 = ct{991};
t2441 = ct{992};
t2442 = ct{993};
t2443 = ct{994};
t2444 = ct{995};
t2447 = ct{996};
t2448 = ct{997};
t2449 = ct{998};
t245 = ct{999};
t2451 = ct{1000};
t2452 = ct{1001};
t2453 = ct{1002};
t2454 = ct{1003};
t2455 = ct{1004};
t2457 = ct{1005};
t2459 = ct{1006};
t2462 = ct{1007};
t2463 = ct{1008};
t2467 = ct{1009};
t247 = ct{1010};
t2471 = ct{1011};
t2472 = ct{1012};
t2473 = ct{1013};
t2475 = ct{1014};
t2476 = ct{1015};
t2477 = ct{1016};
t2478 = ct{1017};
t2479 = ct{1018};
t248 = ct{1019};
t2484 = ct{1020};
t2486 = ct{1021};
t2488 = ct{1022};
t2489 = ct{1023};
t249 = ct{1024};
t2490 = ct{1025};
t2497 = ct{1026};
t2498 = ct{1027};
t2499 = ct{1028};
t25 = ct{1029};
t2500 = ct{1030};
t2501 = ct{1031};
t2502 = ct{1032};
t2503 = ct{1033};
t2504 = ct{1034};
t2507 = ct{1035};
t2508 = ct{1036};
t2509 = ct{1037};
t2511 = ct{1038};
t2515 = ct{1039};
t2517 = ct{1040};
t2518 = ct{1041};
t2520 = ct{1042};
t2523 = ct{1043};
t2525 = ct{1044};
t2526 = ct{1045};
t2527 = ct{1046};
t2529 = ct{1047};
t2530 = ct{1048};
t2531 = ct{1049};
t2532 = ct{1050};
t2533 = ct{1051};
t2534 = ct{1052};
t2535 = ct{1053};
t2543 = ct{1054};
t2546 = ct{1055};
t2547 = ct{1056};
t2548 = ct{1057};
t2549 = ct{1058};
t255 = ct{1059};
t2550 = ct{1060};
t2554 = ct{1061};
t2555 = ct{1062};
t2557 = ct{1063};
t2558 = ct{1064};
t2559 = ct{1065};
t256 = ct{1066};
t2571 = ct{1067};
t2573 = ct{1068};
t2576 = ct{1069};
t2578 = ct{1070};
t258 = ct{1071};
t2580 = ct{1072};
t2581 = ct{1073};
t2582 = ct{1074};
t2583 = ct{1075};
t2590 = ct{1076};
t2592 = ct{1077};
t2593 = ct{1078};
t2599 = ct{1079};
t26 = ct{1080};
t2604 = ct{1081};
t2606 = ct{1082};
t2607 = ct{1083};
t2608 = ct{1084};
t2609 = ct{1085};
t2610 = ct{1086};
t2611 = ct{1087};
t2619 = ct{1088};
t2620 = ct{1089};
t2621 = ct{1090};
t2625 = ct{1091};
t2628 = ct{1092};
t2629 = ct{1093};
t2630 = ct{1094};
t2631 = ct{1095};
t2632 = ct{1096};
t2635 = ct{1097};
t2636 = ct{1098};
t2642 = ct{1099};
t2644 = ct{1100};
t2646 = ct{1101};
t2647 = ct{1102};
t2648 = ct{1103};
t2649 = ct{1104};
t2650 = ct{1105};
t2651 = ct{1106};
t2652 = ct{1107};
t2653 = ct{1108};
t2654 = ct{1109};
t2655 = ct{1110};
t2658 = ct{1111};
t2659 = ct{1112};
t2664 = ct{1113};
t2666 = ct{1114};
t2673 = ct{1115};
t2677 = ct{1116};
t2678 = ct{1117};
t2679 = ct{1118};
t2680 = ct{1119};
t2681 = ct{1120};
t2682 = ct{1121};
t2684 = ct{1122};
t2686 = ct{1123};
t2687 = ct{1124};
t2690 = ct{1125};
t2693 = ct{1126};
t2695 = ct{1127};
t2696 = ct{1128};
t2697 = ct{1129};
t2699 = ct{1130};
t27 = ct{1131};
t2701 = ct{1132};
t2702 = ct{1133};
t2703 = ct{1134};
t2704 = ct{1135};
t2705 = ct{1136};
t2708 = ct{1137};
t2709 = ct{1138};
t2711 = ct{1139};
t2713 = ct{1140};
t2715 = ct{1141};
t2716 = ct{1142};
t2717 = ct{1143};
t2718 = ct{1144};
t2719 = ct{1145};
t2720 = ct{1146};
t2721 = ct{1147};
t2722 = ct{1148};
t2723 = ct{1149};
t2724 = ct{1150};
t2727 = ct{1151};
t2729 = ct{1152};
t2731 = ct{1153};
t2734 = ct{1154};
t2736 = ct{1155};
t2737 = ct{1156};
t2738 = ct{1157};
t2739 = ct{1158};
t2740 = ct{1159};
t2743 = ct{1160};
t2744 = ct{1161};
t2745 = ct{1162};
t2747 = ct{1163};
t2749 = ct{1164};
t2750 = ct{1165};
t2751 = ct{1166};
t2755 = ct{1167};
t2760 = ct{1168};
t2761 = ct{1169};
t2762 = ct{1170};
t2764 = ct{1171};
t2765 = ct{1172};
t2766 = ct{1173};
t2768 = ct{1174};
t2769 = ct{1175};
t2772 = ct{1176};
t2775 = ct{1177};
t2776 = ct{1178};
t2777 = ct{1179};
t2779 = ct{1180};
t2780 = ct{1181};
t2781 = ct{1182};
t2782 = ct{1183};
t2783 = ct{1184};
t2784 = ct{1185};
t2789 = ct{1186};
t279 = ct{1187};
t2790 = ct{1188};
t2794 = ct{1189};
t2795 = ct{1190};
t2796 = ct{1191};
t2797 = ct{1192};
t2798 = ct{1193};
t2799 = ct{1194};
t28 = ct{1195};
t2803 = ct{1196};
t2807 = ct{1197};
t2808 = ct{1198};
t2813 = ct{1199};
t2817 = ct{1200};
t2819 = ct{1201};
t2820 = ct{1202};
t2821 = ct{1203};
t2823 = ct{1204};
t2824 = ct{1205};
t2826 = ct{1206};
t2829 = ct{1207};
t283 = ct{1208};
t2830 = ct{1209};
t2836 = ct{1210};
t2837 = ct{1211};
t2838 = ct{1212};
t2839 = ct{1213};
t2841 = ct{1214};
t2842 = ct{1215};
t2843 = ct{1216};
t2849 = ct{1217};
t2854 = ct{1218};
t2856 = ct{1219};
t2857 = ct{1220};
t2860 = ct{1221};
t2862 = ct{1222};
t2863 = ct{1223};
t2865 = ct{1224};
t2868 = ct{1225};
t2871 = ct{1226};
t2876 = ct{1227};
t2877 = ct{1228};
t2878 = ct{1229};
t2879 = ct{1230};
t2882 = ct{1231};
t2884 = ct{1232};
t2891 = ct{1233};
t2894 = ct{1234};
t2895 = ct{1235};
t2897 = ct{1236};
t2899 = ct{1237};
t29 = ct{1238};
t2900 = ct{1239};
t2901 = ct{1240};
t2911 = ct{1241};
t2912 = ct{1242};
t2913 = ct{1243};
t2914 = ct{1244};
t2915 = ct{1245};
t2916 = ct{1246};
t2919 = ct{1247};
t2920 = ct{1248};
t2925 = ct{1249};
t2927 = ct{1250};
t2929 = ct{1251};
t2934 = ct{1252};
t2936 = ct{1253};
t2937 = ct{1254};
t2940 = ct{1255};
t2942 = ct{1256};
t2944 = ct{1257};
t2946 = ct{1258};
t2947 = ct{1259};
t2949 = ct{1260};
t2951 = ct{1261};
t2953 = ct{1262};
t2954 = ct{1263};
t2956 = ct{1264};
t2959 = ct{1265};
t2966 = ct{1266};
t2967 = ct{1267};
t2969 = ct{1268};
t2970 = ct{1269};
t2971 = ct{1270};
t2974 = ct{1271};
t2976 = ct{1272};
t2977 = ct{1273};
t2978 = ct{1274};
t2979 = ct{1275};
t2982 = ct{1276};
t2983 = ct{1277};
t2985 = ct{1278};
t2989 = ct{1279};
t299 = ct{1280};
t2991 = ct{1281};
t2992 = ct{1282};
t2995 = ct{1283};
t2996 = ct{1284};
t2999 = ct{1285};
t2d = ct{1286};
t2dd = ct{1287};
t30 = ct{1288};
t3005 = ct{1289};
t3007 = ct{1290};
t3008 = ct{1291};
t301 = ct{1292};
t3010 = ct{1293};
t3011 = ct{1294};
t3012 = ct{1295};
t3013 = ct{1296};
t3014 = ct{1297};
t3015 = ct{1298};
t3016 = ct{1299};
t3018 = ct{1300};
t3020 = ct{1301};
t3021 = ct{1302};
t3023 = ct{1303};
t3028 = ct{1304};
t303 = ct{1305};
t3030 = ct{1306};
t3031 = ct{1307};
t3032 = ct{1308};
t3033 = ct{1309};
t3035 = ct{1310};
t3038 = ct{1311};
t3039 = ct{1312};
t3042 = ct{1313};
t3043 = ct{1314};
t3059 = ct{1315};
t3060 = ct{1316};
t3066 = ct{1317};
t3069 = ct{1318};
t3071 = ct{1319};
t3072 = ct{1320};
t3073 = ct{1321};
t3078 = ct{1322};
t3079 = ct{1323};
t308 = ct{1324};
t3080 = ct{1325};
t3082 = ct{1326};
t3083 = ct{1327};
t3086 = ct{1328};
t3087 = ct{1329};
t3088 = ct{1330};
t309 = ct{1331};
t3099 = ct{1332};
t31 = ct{1333};
t3101 = ct{1334};
t3102 = ct{1335};
t3103 = ct{1336};
t3122 = ct{1337};
t3123 = ct{1338};
t3125 = ct{1339};
t3129 = ct{1340};
t3130 = ct{1341};
t3148 = ct{1342};
t315 = ct{1343};
t3154 = ct{1344};
t3160 = ct{1345};
t3163 = ct{1346};
t3166 = ct{1347};
t3168 = ct{1348};
t3169 = ct{1349};
t317 = ct{1350};
t3175 = ct{1351};
t3176 = ct{1352};
t3177 = ct{1353};
t318 = ct{1354};
t3183 = ct{1355};
t3185 = ct{1356};
t319 = ct{1357};
t320 = ct{1358};
t3207 = ct{1359};
t321 = ct{1360};
t3214 = ct{1361};
t3230 = ct{1362};
t3232 = ct{1363};
t3234 = ct{1364};
t3237 = ct{1365};
t325 = ct{1366};
t3250 = ct{1367};
t3251 = ct{1368};
t3259 = ct{1369};
t3260 = ct{1370};
t3272 = ct{1371};
t3288 = ct{1372};
t3289 = ct{1373};
t329 = ct{1374};
t3291 = ct{1375};
t3292 = ct{1376};
t3298 = ct{1377};
t330 = ct{1378};
t3306 = ct{1379};
t3308 = ct{1380};
t331 = ct{1381};
t3318 = ct{1382};
t332 = ct{1383};
t3321 = ct{1384};
t333 = ct{1385};
t3330 = ct{1386};
t3331 = ct{1387};
t3332 = ct{1388};
t3335 = ct{1389};
t334 = ct{1390};
t3340 = ct{1391};
t3341 = ct{1392};
t3342 = ct{1393};
t3343 = ct{1394};
t3345 = ct{1395};
t3348 = ct{1396};
t3349 = ct{1397};
t3351 = ct{1398};
t3354 = ct{1399};
t3355 = ct{1400};
t3360 = ct{1401};
t3368 = ct{1402};
t3381 = ct{1403};
t3383 = ct{1404};
t3384 = ct{1405};
t3388 = ct{1406};
t3391 = ct{1407};
t3399 = ct{1408};
t34 = ct{1409};
t3400 = ct{1410};
t3401 = ct{1411};
t3404 = ct{1412};
t3405 = ct{1413};
t341 = ct{1414};
t3414 = ct{1415};
t3415 = ct{1416};
t3416 = ct{1417};
t342 = ct{1418};
t3421 = ct{1419};
t3429 = ct{1420};
t343 = ct{1421};
t3431 = ct{1422};
t3432 = ct{1423};
t3433 = ct{1424};
t3439 = ct{1425};
t344 = ct{1426};
t3440 = ct{1427};
t3445 = ct{1428};
t345 = ct{1429};
t3452 = ct{1430};
t3456 = ct{1431};
t3457 = ct{1432};
t3458 = ct{1433};
t3459 = ct{1434};
t346 = ct{1435};
t3460 = ct{1436};
t3461 = ct{1437};
t3466 = ct{1438};
t3467 = ct{1439};
t3468 = ct{1440};
t3469 = ct{1441};
t347 = ct{1442};
t3488 = ct{1443};
t3498 = ct{1444};
t35 = ct{1445};
t3500 = ct{1446};
t3504 = ct{1447};
t3509 = ct{1448};
t3510 = ct{1449};
t3513 = ct{1450};
t3516 = ct{1451};
t3517 = ct{1452};
t3523 = ct{1453};
t3531 = ct{1454};
t354 = ct{1455};
t3543 = ct{1456};
t3544 = ct{1457};
t3546 = ct{1458};
t3556 = ct{1459};
t3557 = ct{1460};
t3567 = ct{1461};
t3568 = ct{1462};
t3574 = ct{1463};
t3575 = ct{1464};
t3578 = ct{1465};
t3579 = ct{1466};
t3580 = ct{1467};
t3582 = ct{1468};
t3590 = ct{1469};
t3598 = ct{1470};
t36 = ct{1471};
t3601 = ct{1472};
t3606 = ct{1473};
t3612 = ct{1474};
t3617 = ct{1475};
t3622 = ct{1476};
t3628 = ct{1477};
t3630 = ct{1478};
t364 = ct{1479};
t3649 = ct{1480};
t365 = ct{1481};
t3674 = ct{1482};
t3678 = ct{1483};
t368 = ct{1484};
t3683 = ct{1485};
t3685 = ct{1486};
t3686 = ct{1487};
t3687 = ct{1488};
t3697 = ct{1489};
t37 = ct{1490};
t3701 = ct{1491};
t3704 = ct{1492};
t3712 = ct{1493};
t3716 = ct{1494};
t3721 = ct{1495};
t3724 = ct{1496};
t3734 = ct{1497};
t3741 = ct{1498};
t3743 = ct{1499};
t3744 = ct{1500};
t3745 = ct{1501};
t3747 = ct{1502};
t3750 = ct{1503};
t3751 = ct{1504};
t3758 = ct{1505};
t3761 = ct{1506};
t3768 = ct{1507};
t3769 = ct{1508};
t3770 = ct{1509};
t3771 = ct{1510};
t3779 = ct{1511};
t3785 = ct{1512};
t3786 = ct{1513};
t3792 = ct{1514};
t3796 = ct{1515};
t38 = ct{1516};
t3813 = ct{1517};
t3817 = ct{1518};
t3821 = ct{1519};
t3822 = ct{1520};
t3830 = ct{1521};
t384 = ct{1522};
t3840 = ct{1523};
t3843 = ct{1524};
t3846 = ct{1525};
t3852 = ct{1526};
t3853 = ct{1527};
t3871 = ct{1528};
t3872 = ct{1529};
t3875 = ct{1530};
t3877 = ct{1531};
t3878 = ct{1532};
t3897 = ct{1533};
t39 = ct{1534};
t3903 = ct{1535};
t3906 = ct{1536};
t3907 = ct{1537};
t392 = ct{1538};
t3923 = ct{1539};
t393 = ct{1540};
t3940 = ct{1541};
t3941 = ct{1542};
t3943 = ct{1543};
t3949 = ct{1544};
t3956 = ct{1545};
t3967 = ct{1546};
t3976 = ct{1547};
t3997 = ct{1548};
t3d = ct{1549};
t3dd = ct{1550};
t4004 = ct{1551};
t4006 = ct{1552};
t401 = ct{1553};
t402 = ct{1554};
t4025 = ct{1555};
t4028 = ct{1556};
t403 = ct{1557};
t404 = ct{1558};
t4050 = ct{1559};
t4058 = ct{1560};
t4059 = ct{1561};
t4069 = ct{1562};
t4071 = ct{1563};
t4075 = ct{1564};
t4076 = ct{1565};
t4080 = ct{1566};
t4084 = ct{1567};
t4086 = ct{1568};
t4096 = ct{1569};
t4098 = ct{1570};
t41 = ct{1571};
t410 = ct{1572};
t4103 = ct{1573};
t411 = ct{1574};
t4112 = ct{1575};
t412 = ct{1576};
t4125 = ct{1577};
t4126 = ct{1578};
t4129 = ct{1579};
t413 = ct{1580};
t4130 = ct{1581};
t4131 = ct{1582};
t4133 = ct{1583};
t4134 = ct{1584};
t4139 = ct{1585};
t414 = ct{1586};
t4140 = ct{1587};
t4142 = ct{1588};
t4143 = ct{1589};
t4144 = ct{1590};
t4146 = ct{1591};
t4147 = ct{1592};
t4149 = ct{1593};
t415 = ct{1594};
t4150 = ct{1595};
t4152 = ct{1596};
t4157 = ct{1597};
t4158 = ct{1598};
t4159 = ct{1599};
t416 = ct{1600};
t4160 = ct{1601};
t4165 = ct{1602};
t4166 = ct{1603};
t4169 = ct{1604};
t4170 = ct{1605};
t4172 = ct{1606};
t4176 = ct{1607};
t4178 = ct{1608};
t418 = ct{1609};
t419 = ct{1610};
t42 = ct{1611};
t420 = ct{1612};
t4203 = ct{1613};
t4212 = ct{1614};
t4221 = ct{1615};
t4226 = ct{1616};
t4230 = ct{1617};
t4231 = ct{1618};
t4236 = ct{1619};
t425 = ct{1620};
t4256 = ct{1621};
t4290 = ct{1622};
t4299 = ct{1623};
t4304 = ct{1624};
t4309 = ct{1625};
t431 = ct{1626};
t4321 = ct{1627};
t4325 = ct{1628};
t4326 = ct{1629};
t4332 = ct{1630};
t4334 = ct{1631};
t4335 = ct{1632};
t434 = ct{1633};
t4348 = ct{1634};
t4353 = ct{1635};
t437 = ct{1636};
t4379 = ct{1637};
t4381 = ct{1638};
t4389 = ct{1639};
t441 = ct{1640};
t4416 = ct{1641};
t442 = ct{1642};
t443 = ct{1643};
t444 = ct{1644};
t446 = ct{1645};
t4470 = ct{1646};
t4475 = ct{1647};
t4486 = ct{1648};
t453 = ct{1649};
t4538 = ct{1650};
t454 = ct{1651};
t4541 = ct{1652};
t4547 = ct{1653};
t4551 = ct{1654};
t4556 = ct{1655};
t4579 = ct{1656};
t459 = ct{1657};
t4591 = ct{1658};
t4595 = ct{1659};
t470 = ct{1660};
t478 = ct{1661};
t4785 = ct{1662};
t4787 = ct{1663};
t48 = ct{1664};
t4801 = ct{1665};
t483 = ct{1666};
t4831 = ct{1667};
t484 = ct{1668};
t4858 = ct{1669};
t486 = ct{1670};
t4862 = ct{1671};
t487 = ct{1672};
t488 = ct{1673};
t4881 = ct{1674};
t4908 = ct{1675};
t492 = ct{1676};
t493 = ct{1677};
t4931 = ct{1678};
t494 = ct{1679};
t495 = ct{1680};
t4950 = ct{1681};
t496 = ct{1682};
t497 = ct{1683};
t4979 = ct{1684};
t498 = ct{1685};
t4985 = ct{1686};
t4d = ct{1687};
t4dd = ct{1688};
t50 = ct{1689};
t5006 = ct{1690};
t501 = ct{1691};
t503 = ct{1692};
t508 = ct{1693};
t51 = ct{1694};
t514 = ct{1695};
t515 = ct{1696};
t516 = ct{1697};
t519 = ct{1698};
t523 = ct{1699};
t524 = ct{1700};
t529 = ct{1701};
t53 = ct{1702};
t530 = ct{1703};
t532 = ct{1704};
t537 = ct{1705};
t543 = ct{1706};
t544 = ct{1707};
t546 = ct{1708};
t547 = ct{1709};
t548 = ct{1710};
t549 = ct{1711};
t55 = ct{1712};
t550 = ct{1713};
t552 = ct{1714};
t553 = ct{1715};
t554 = ct{1716};
t56 = ct{1717};
t562 = ct{1718};
t569 = ct{1719};
t57 = ct{1720};
t570 = ct{1721};
t58 = ct{1722};
t582 = ct{1723};
t588 = ct{1724};
t589 = ct{1725};
t591 = ct{1726};
t593 = ct{1727};
t596 = ct{1728};
t598 = ct{1729};
t5d = ct{1730};
t5dd = ct{1731};
t601 = ct{1732};
t602 = ct{1733};
t604 = ct{1734};
t608 = ct{1735};
t609 = ct{1736};
t61 = ct{1737};
t612 = ct{1738};
t614 = ct{1739};
t615 = ct{1740};
t616 = ct{1741};
t617 = ct{1742};
t623 = ct{1743};
t627 = ct{1744};
t63 = ct{1745};
t632 = ct{1746};
t633 = ct{1747};
t634 = ct{1748};
t635 = ct{1749};
t636 = ct{1750};
t637 = ct{1751};
t639 = ct{1752};
t641 = ct{1753};
t642 = ct{1754};
t643 = ct{1755};
t644 = ct{1756};
t645 = ct{1757};
t646 = ct{1758};
t647 = ct{1759};
t648 = ct{1760};
t649 = ct{1761};
t650 = ct{1762};
t651 = ct{1763};
t652 = ct{1764};
t653 = ct{1765};
t654 = ct{1766};
t655 = ct{1767};
t658 = ct{1768};
t659 = ct{1769};
t660 = ct{1770};
t662 = ct{1771};
t663 = ct{1772};
t664 = ct{1773};
t665 = ct{1774};
t667 = ct{1775};
t668 = ct{1776};
t670 = ct{1777};
t671 = ct{1778};
t673 = ct{1779};
t675 = ct{1780};
t680 = ct{1781};
t681 = ct{1782};
t682 = ct{1783};
t684 = ct{1784};
t685 = ct{1785};
t687 = ct{1786};
t689 = ct{1787};
t69 = ct{1788};
t690 = ct{1789};
t691 = ct{1790};
t694 = ct{1791};
t695 = ct{1792};
t696 = ct{1793};
t698 = ct{1794};
t699 = ct{1795};
t6d = ct{1796};
t6dd = ct{1797};
t701 = ct{1798};
t702 = ct{1799};
t703 = ct{1800};
t705 = ct{1801};
t706 = ct{1802};
t71 = ct{1803};
t711 = ct{1804};
t712 = ct{1805};
t713 = ct{1806};
t714 = ct{1807};
t720 = ct{1808};
t721 = ct{1809};
t723 = ct{1810};
t724 = ct{1811};
t725 = ct{1812};
t726 = ct{1813};
t729 = ct{1814};
t731 = ct{1815};
t732 = ct{1816};
t733 = ct{1817};
t735 = ct{1818};
t736 = ct{1819};
t738 = ct{1820};
t739 = ct{1821};
t742 = ct{1822};
t745 = ct{1823};
t746 = ct{1824};
t747 = ct{1825};
t748 = ct{1826};
t75 = ct{1827};
t752 = ct{1828};
t755 = ct{1829};
t759 = ct{1830};
t760 = ct{1831};
t761 = ct{1832};
t763 = ct{1833};
t764 = ct{1834};
t772 = ct{1835};
t774 = ct{1836};
t775 = ct{1837};
t776 = ct{1838};
t780 = ct{1839};
t781 = ct{1840};
t782 = ct{1841};
t785 = ct{1842};
t788 = ct{1843};
t789 = ct{1844};
t793 = ct{1845};
t799 = ct{1846};
t8 = ct{1847};
t802 = ct{1848};
t805 = ct{1849};
t806 = ct{1850};
t807 = ct{1851};
t808 = ct{1852};
t82 = ct{1853};
t820 = ct{1854};
t823 = ct{1855};
t824 = ct{1856};
t825 = ct{1857};
t826 = ct{1858};
t827 = ct{1859};
t828 = ct{1860};
t830 = ct{1861};
t831 = ct{1862};
t832 = ct{1863};
t833 = ct{1864};
t835 = ct{1865};
t838 = ct{1866};
t842 = ct{1867};
t843 = ct{1868};
t844 = ct{1869};
t846 = ct{1870};
t848 = ct{1871};
t849 = ct{1872};
t850 = ct{1873};
t851 = ct{1874};
t852 = ct{1875};
t853 = ct{1876};
t854 = ct{1877};
t855 = ct{1878};
t859 = ct{1879};
t861 = ct{1880};
t865 = ct{1881};
t866 = ct{1882};
t870 = ct{1883};
t871 = ct{1884};
t873 = ct{1885};
t879 = ct{1886};
t88 = ct{1887};
t880 = ct{1888};
t884 = ct{1889};
t885 = ct{1890};
t887 = ct{1891};
t888 = ct{1892};
t890 = ct{1893};
t891 = ct{1894};
t892 = ct{1895};
t896 = ct{1896};
t897 = ct{1897};
t898 = ct{1898};
t899 = ct{1899};
t9 = ct{1900};
t900 = ct{1901};
t907 = ct{1902};
t908 = ct{1903};
t909 = ct{1904};
t910 = ct{1905};
t911 = ct{1906};
t912 = ct{1907};
t915 = ct{1908};
t917 = ct{1909};
t919 = ct{1910};
t922 = ct{1911};
t923 = ct{1912};
t927 = ct{1913};
t928 = ct{1914};
t930 = ct{1915};
t932 = ct{1916};
t937 = ct{1917};
t943 = ct{1918};
t944 = ct{1919};
t945 = ct{1920};
t947 = ct{1921};
t949 = ct{1922};
t952 = ct{1923};
t959 = ct{1924};
t960 = ct{1925};
t961 = ct{1926};
t962 = ct{1927};
t963 = ct{1928};
t964 = ct{1929};
t965 = ct{1930};
t966 = ct{1931};
t967 = ct{1932};
t968 = ct{1933};
t969 = ct{1934};
t970 = ct{1935};
t972 = ct{1936};
t973 = ct{1937};
t974 = ct{1938};
t975 = ct{1939};
t976 = ct{1940};
t977 = ct{1941};
t978 = ct{1942};
t979 = ct{1943};
t980 = ct{1944};
t981 = ct{1945};
t982 = ct{1946};
t983 = ct{1947};
t986 = ct{1948};
t987 = ct{1949};
t989 = ct{1950};
t992 = ct{1951};
t993 = ct{1952};
t994 = ct{1953};
t997 = ct{1954};
t999 = ct{1955};
t3022 = t550+t2654;
t3024 = t641.*t2578;
t3026 = -t14.*t39.*(t1315-t1898);
t3027 = t1523+t1856;
t3036 = t1593+t1819;
t3041 = -t3030;
t3044 = t14.*t39.*(t1315-t1898);
t3051 = t2578.*(t101-t401).*-2.0;
t3056 = t8.*t3023;
t3058 = t1726+t1774;
t3061 = t724.*t2578;
t3064 = t2578.*(t101-t401).*2.0;
t3070 = t14.*t3033;
t3076 = t739.*t2578;
t3081 = t1752+t1771;
t3090 = -t3079;
t3097 = -t3071;
t3098 = t780.*t2578;
t3100 = t808.*(t544-t1021+t330.*(t100-t364));
t3106 = t1761+t1795;
t3107 = t1762+t1793;
t3121 = -t255.*(t1315-t1898);
t3128 = t807.*t2578;
t3140 = t3099./2.0;
t3151 = t1778+t1805;
t3152 = t1777+t1808;
t3158 = -t14.*(t1743-t1783);
t3162 = t866.*t2578;
t3165 = t14.*t37.*t2578.*(t101-t401);
t3179 = t255.*(t1315-t1898).*(-1.0./2.0);
t3182 = t3123./2.0;
t3189 = t3163.*(-1.0./2.0);
t3204 = t3163./2.0;
t3220 = t14.*(t1743-t1783).*(-1.0./2.0);
t3224 = t937.*t2578.*(-1.0./2.0);
t3231 = t3177./2.0;
t3235 = t8.*t3175;
t3236 = t3207.*t6dd;
t3238 = t14.*t3176;
t3240 = (t937.*t2578)./2.0;
t3246 = -t8.*t37.*(t1743-t1783);
t3283 = t8.*t37.*(t1743-t1783).*(-1.0./2.0);
t3285 = t8.*t39.*(t1743-t1783).*(-1.0./2.0);
t3326 = t1935.*(t890+t8.*(t553-t8.*t15.*(1.53e+2./2.5e+2))).*(-1.0./2.0);
t3357 = t3341.*t5dd;
t3358 = t3342.*t5dd;
t3359 = t14.*t1082.*t2654;
t3366 = -t3355;
t3377 = t187+t413+t444+t589+t1066+t1138;
t3380 = t3349./2.0;
t3390 = t3360./2.0;
t3428 = t196+t320+t654+t658+t997+t1025;
t3464 = t2049+t2078;
t3472 = -t3452;
t3473 = -t3458;
t3477 = t18.*t39.*t3368;
t3478 = t14.*t3433;
t3483 = -t3461;
t3485 = t496+t547+t651+t660+t782+t808;
t3487 = t911+t912+t1157+t1198;
t3521 = t8.*t39.*t3433;
t3522 = t2103+t2134;
t3532 = t1829+t2382;
t3555 = t255.*t3368;
t3562 = t2131+t2161;
t3577 = t330.*t3368;
t3600 = t3579.*(-1.0./2.0);
t3602 = t1504+t2705;
t3607 = t341.*t3368;
t3613 = -t3580;
t3614 = t2137+t2199;
t3623 = t3580./2.0;
t3625 = t402.*t3368;
t3634 = t1971+t2414;
t3651 = t330.*t3433;
t3688 = (t705.*t3251)./2.0;
t3722 = t609.*t3368;
t3732 = t258+t410+t411+t412+t2729;
t3754 = t334+t414+t415+t416+t2736;
t3755 = -t3368.*(t100-t364);
t3756 = -t3741;
t3757 = t641.*t3368;
t3762 = t2240+t2323;
t3765 = -t3751;
t3767 = t14.*t1807.*t2654;
t3781 = t14.*t1818.*t2654;
t3784 = -t3368.*(t101-t401);
t3789 = t2030+t2554;
t3803 = t2094+t2523;
t3804 = t805+t830+t835+t892+t1269;
t3812 = t3785./2.0;
t3826 = t673+t2059+t2061;
t3828 = t8.*(t2523-t1420.*(t101-t401));
t3833 = t1773+t2783;
t3845 = t780+t887+t891+t937+t1270;
t3848 = t14.*t1082.*t3251;
t3850 = t1770+t2824;
t3874 = t3843./2.0;
t3887 = t14.*t37.*(t2523-t1420.*(t101-t401));
t3888 = t14.*t39.*(t2523-t1420.*(t101-t401));
t3917 = t38.*t39.*(t2523-t1420.*(t101-t401));
t3936 = t1287.*t3251;
t3948 = t14.*t2113.*t2654;
t3954 = -t3923;
t3965 = t3923./2.0;
t3968 = -t3943;
t3972 = t14.*t2140.*t2654;
t3974 = (t2123.*t2654)./2.0;
t3982 = t3943./2.0;
t4003 = t3976./2.0;
t4007 = t255.*(t2523-t1420.*(t101-t401));
t4012 = t4006.*(-1.0./2.0);
t4018 = t1062+t1119+t1409+t1657;
t4024 = t14.*t2279.*t2654;
t4027 = -t3082.*(t746-t748);
t4042 = t3082.*(t746-t748).*(-1.0./2.0);
t4048 = (t3082.*(t746-t748))./2.0;
t4049 = t2518+t2571;
t4055 = (t14.*t2357.*t2654)./2.0;
t4077 = t1668+t1928+t1931;
t4085 = t799.*t3750;
t4102 = t14.*t1807.*t3251;
t4109 = t14.*t1818.*t3251;
t4115 = -t4103;
t4118 = t4103./2.0;
t4128 = t1961.*t3251;
t4132 = -t4125;
t4136 = t4125./2.0;
t4151 = -t4149;
t4162 = t14.*t2113.*t3251;
t4164 = t960+t2343+t2439;
t4171 = t4165.*2.0;
t4173 = t14.*t2140.*t3251;
t4175 = t2167.*t3251;
t4179 = -t4165;
t4183 = -t4169;
t4185 = -t4176;
t4186 = t4166./2.0;
t4188 = t4169./2.0;
t4204 = t2739+t2794;
t4233 = t14.*t2279.*t3251;
t4237 = -t4231;
t4252 = t2530.*t3082;
t4268 = t309+t663+t974+t993+t1018+t1041+t1167;
t4273 = t303+t662+t975+t994+t1008+t1034+t1168;
t4296 = (t14.*t2357.*t3251)./2.0;
t4324 = t1005+t2515+t2547;
t4327 = -t4321;
t4333 = t1462+t1494+t1749+t1768;
t4342 = -t2654.*(t910-t2473);
t4361 = -t4348;
t4367 = t4348./2.0;
t4386 = t2654.*t3251;
t4394 = -t4389;
t4395 = t4389./2.0;
t4397 = t2058+t2212+t2335;
t4403 = -t14.*(t2578.*(t100-t364)+t609.*(t544-t1021+t330.*(t100-t364)));
t4406 = t14.*(t2578.*(t100-t364)+t609.*(t544-t1021+t330.*(t100-t364))).*(-1.0./2.0);
t4409 = t3038+t3039;
t4413 = -t8.*t37.*(t2578.*(t100-t364)+t609.*(t544-t1021+t330.*(t100-t364)));
t4414 = -t8.*t39.*(t2578.*(t100-t364)+t609.*(t544-t1021+t330.*(t100-t364)));
t4418 = -t35.*t39.*(t2578.*(t100-t364)+t609.*(t544-t1021+t330.*(t100-t364)));
t4421 = t8.*t39.*(t2578.*(t100-t364)+t609.*(t544-t1021+t330.*(t100-t364)));
t4424 = -t4416;
t4425 = t8.*t37.*(t2578.*(t100-t364)+t609.*(t544-t1021+t330.*(t100-t364))).*(-1.0./2.0);
t4429 = t35.*t39.*(t2578.*(t100-t364)+t609.*(t544-t1021+t330.*(t100-t364)));
t4430 = (t8.*t37.*(t2578.*(t100-t364)+t609.*(t544-t1021+t330.*(t100-t364))))./2.0;
t4442 = t2300.*t3750;
t4443 = t2749.*t3383;
t4451 = -t4050.*(t746-t748);
t4458 = t3102+t3103;
t4468 = t4050.*(t746-t748).*(-1.0./2.0);
t4469 = t1426+t1756+t2017+t2037;
t4471 = t2082+t2426+t2462;
t4482 = -t4475;
t4483 = t330.*(t2578.*(t100-t364)+t609.*(t544-t1021+t330.*(t100-t364))).*(-1.0./2.0);
t4487 = t4475./2.0;
t4491 = t3154+t3160;
t4494 = (t1875.*t4050)./2.0;
t4499 = -t3251.*(t910-t2473);
t4513 = t2581+t3786;
t4528 = t1610+t1680+t1827+t2380;
t4534 = t3082.*t3405;
t4539 = (t2666.*t3750)./2.0;
t4540 = (t3083.*t3383)./2.0;
t4548 = -t4541;
t4560 = t2749.*t3750;
t4573 = t2649+t3907;
t4582 = t14.*t1807.*t4178;
t4584 = t2650+t3940;
t4596 = t3343+t3345;
t4597 = t4591.*(-1.0./2.0);
t4602 = -t4595;
t4604 = t4591./2.0;
t4627 = t2530.*t4050;
t4648 = t2270.*t4130;
t4665 = (t3082.*t3687)./2.0;
t4668 = t14.*t2113.*t4178;
t4669 = t3083.*t3750;
t4678 = t8.*t1807.*t4335;
t4695 = t3466+t3467;
t4704 = t3082.*t3822;
t4705 = t14.*t1807.*t4353;
t4707 = t14.*t2279.*t4178;
t4747 = t8.*t2113.*t4335;
t4759 = t14.*t2113.*t4353;
t4776 = t8.*t2279.*t4335;
t4789 = t2654.*t4178;
t4798 = t14.*t2279.*t4353;
t4800 = t3082.*t4050;
t4837 = -t4831;
t4838 = t4831./2.0;
t4853 = t2658.*t4335;
t4856 = t3082.*t4131;
t4863 = t2654.*t4353;
t4867 = -t4862;
t4870 = t4862./2.0;
t4887 = -t4881;
t4889 = t4881./2.0;
t4893 = t980+t1029+t1030+t2110+t2172+t2177;
t4907 = (t3251.*t4178)./2.0;
t4917 = t1666+t1669+t4379;
t4921 = -t4335.*(t873-t2434);
t4923 = t3082.*t4334;
t4924 = t4335.*(t873-t2434).*-2.0;
t4930 = (t3687.*t4050)./2.0;
t4937 = -t4931;
t4940 = -t4353.*(t910-t2473);
t4941 = t4931./2.0;
t4944 = t4353.*(t910-t2473).*-2.0;
t4949 = t3230.*t4335;
t4955 = t3251.*t4353;
t4957 = (t3822.*t4050)./2.0;
t4990 = t4985.*(-1.0./2.0);
t4992 = t4985./2.0;
t5010 = t5006.*2.0;
t5012 = -t5006;
t5018 = t4075+t4080;
t5020 = t4050.*t4131;
t5047 = -t37.*(-t1800+t2379+t2497+t18.*t39.*(-t495-t548+t650+t659+t739+t14.*t37.*(t101-t401)));
t5051 = -t18.*t39.*(-t1800+t2379+t2497+t18.*t39.*(-t495-t548+t650+t659+t739+t14.*t37.*(t101-t401)));
t5056 = t37.*(-t1800+t2379+t2497+t18.*t39.*(-t495-t548+t650+t659+t739+t14.*t37.*(t101-t401))).*(-1.0./2.0);
t5065 = t18.*t39.*(-t1800+t2379+t2497+t18.*t39.*(-t495-t548+t650+t659+t739+t14.*t37.*(t101-t401))).*(-1.0./2.0);
t5074 = (t18.*t39.*(-t1800+t2379+t2497+t18.*t39.*(-t495-t548+t650+t659+t739+t14.*t37.*(t101-t401))))./2.0;
t5093 = t4050.*t4334;
t5106 = t1922+t2410+t2635+t3779;
t5114 = t1932+t2413+t2695+t3721;
t5283 = t3060+t3072+t3513+t3531;
t5292 = t3122+t3148+t3498+t3500;
t5465 = -t6d.*(t4165+t4335.*(t873-t2434)+t4353.*(t910-t2473));
t996 = -t977;
t1081 = -t1032;
t1132 = -t1090;
t1136 = -t1095;
t1143 = -t1101;
t1160 = -t1109;
t1162 = -t1110;
t1249 = t28.*t1148;
t1266 = t1234.*t1d;
t1281 = t1217./2.0;
t1346 = t1301.*t2d;
t1347 = t1301.*t3d;
t1348 = t1301.*t4d;
t1350 = -t1326;
t1356 = -t1308;
t1359 = -t1312;
t1363 = -t1317;
t1385 = t1312./2.0;
t1388 = t1317./2.0;
t1412 = -t1395;
t1428 = t37.*t1289;
t1464 = t18.*t39.*t1289;
t1477 = -t1460;
t1496 = t1449./2.0;
t1577 = -t1550;
t1608 = -t1559;
t1611 = -t1565;
t1612 = -t1568;
t1613 = -t1581;
t1614 = -t1582;
t1617 = t18.*t1571.*t1dd;
t1619 = t1556./2.0;
t1620 = t1560./2.0;
t1621 = t1561./2.0;
t1622 = t1565./2.0;
t1623 = t1566./2.0;
t1624 = t1567./2.0;
t1638 = t34.*t1569;
t1642 = t38.*t1571;
t1665 = -t1643;
t1681 = -t1639;
t1685 = -t1673;
t1700 = -t1662;
t1717 = t1656./2.0;
t1719 = t1658./2.0;
t1721 = t1662./2.0;
t1722 = t1664./2.0;
t1725 = t8.*t1663;
t1744 = -t1691;
t1746 = -t1694;
t1747 = -t1716;
t1760 = t1686./2.0;
t1764 = t1691./2.0;
t1766 = t1696./2.0;
t1767 = t1702./2.0;
t1782 = -t1737;
t1796 = t8.*t1738;
t1802 = t14.*t37.*t1663;
t1803 = t14.*t39.*t1663;
t1841 = t1798./2.0;
t1849 = t38.*t39.*t1663;
t1852 = t13.*t1821;
t1854 = t19.*t1821;
t1860 = -t1822;
t1883 = t888+t947;
t1899 = t1843.*t2d;
t1900 = t1843.*t3d;
t1901 = t1843.*t4d;
t1902 = t1828./2.0;
t1913 = t13.*t1858;
t1915 = t19.*t1858;
t1918 = -t1857;
t1927 = -t1864;
t1933 = -t1892;
t1934 = t1894.*2.0;
t1940 = t1894.*t1dd;
t1941 = -t1911;
t1952 = -t1896;
t1964 = -t1943;
t1975 = -t1929;
t1980 = t1896./2.0;
t1982 = t1903./2.0;
t2000 = -t1948;
t2001 = -t1950;
t2004 = -t1954;
t2010 = -t1986;
t2012 = -t1992;
t2013 = -t1998;
t2014 = t1948./2.0;
t2016 = t1950./2.0;
t2018 = t1954./2.0;
t2022 = t255.*t1663;
t2026 = -t1987;
t2062 = -t2042;
t2065 = -t2029;
t2069 = -t2033;
t2071 = t2021./2.0;
t2098 = t2053./2.0;
t2099 = t2054./2.0;
t2102 = t2073.*t1d;
t2105 = t1010+t1063;
t2107 = t1014+t1067;
t2108 = t1042+t1043;
t2143 = -t2125;
t2154 = t1056+t1120;
t2157 = t1058+t1124;
t2223 = t2195.*t2d;
t2224 = t2195.*t3d;
t2230 = -t2209;
t2242 = -t2229;
t2282 = t2226./2.0;
t2289 = -t2274;
t2296 = t1217+t1219;
t2314 = -t2288;
t2317 = t2249./2.0;
t2321 = -t2304;
t2322 = -t2305;
t2327 = t2268./2.0;
t2329 = t2297.*t5d;
t2331 = -t2313;
t2349 = t2330.*(-1.0./2.0);
t2351 = t2293./2.0;
t2369 = t2324./2.0;
t2381 = -t2355;
t2392 = t39.*t2306;
t2394 = t39.*t2308;
t2396 = t2355./2.0;
t2411 = -t2375;
t2415 = -t2378;
t2433 = -t2421;
t2450 = -t2432;
t2460 = -t2437;
t2491 = t2451./2.0;
t2492 = t8.*t2444;
t2493 = t2452./2.0;
t2494 = t14.*t2443;
t2506 = t2463./2.0;
t2512 = t1051+t1564;
t2513 = t1052+t1563;
t2521 = t88+t1259+t1260;
t2522 = t19.*t2488;
t2536 = -t2517;
t2541 = t13.*t2488;
t2551 = t19.*t2526;
t2562 = -t2531;
t2566 = -t2533;
t2569 = -t2548;
t2574 = t13.*t2526;
t2584 = t2531./2.0;
t2585 = t2532./2.0;
t2586 = t2533./2.0;
t2587 = t8.*t39.*t2443;
t2588 = t2534./2.0;
t2589 = t14.*t39.*t2444;
t2595 = t2543./2.0;
t2622 = t2582./2.0;
t2624 = t2583./2.0;
t2645 = t2610./2.0;
t2656 = t2625./2.0;
t2661 = -t2647;
t2675 = t2647./2.0;
t2689 = t2652./2.0;
t2707 = t2673./2.0;
t2710 = t2677./2.0;
t2712 = -t2693;
t2725 = -t2701;
t2752 = t1508+t1539;
t2754 = -t5d.*(t1317+t37.*t200+t8.*t39.*(t478-t519));
t2757 = t2720./2.0;
t2759 = t2734.*t1dd;
t2774 = t967+t968+t1060;
t2800 = -t2d.*(-t967+t1009+(t14.*(t206-t470))./2.0);
t2801 = -t3d.*(-t967+t1009+(t14.*(t206-t470))./2.0);
t2802 = -t4d.*(-t967+t1009+(t14.*(t206-t470))./2.0);
t2804 = t1338+t1791;
t2806 = t37.*t2722;
t2810 = t37.*t2734;
t2812 = t2769./2.0;
t2815 = t39.*t2734;
t2816 = t13.*t2782;
t2818 = t19.*t2782;
t2825 = -t2784;
t2827 = t1422+t1720;
t2828 = t1566+t1567;
t2833 = -t2803;
t2835 = t2789./2.0;
t2840 = t18.*t39.*t2722;
t2848 = t2797./2.0;
t2853 = t13.*t2823;
t2855 = t19.*t2823;
t2858 = t2803./2.0;
t2859 = -t2821;
t2867 = -t2829;
t2880 = -t2836;
t2881 = -t2837;
t2883 = -t2865;
t2885 = t2829./2.0;
t2892 = t2836./2.0;
t2893 = t2837./2.0;
t2910 = t2857./2.0;
t2917 = -t2878;
t2928 = t1487+t1765;
t2933 = t2878./2.0;
t2935 = t37.*t2820;
t2948 = t2891./2.0;
t2961 = t742.*t2361;
t2968 = t18.*t39.*t2820;
t2975 = t14.*t2920;
t2988 = t2940./2.0;
t2994 = -t2969;
t2997 = -t2976;
t2998 = -t2977;
t3004 = t2969./2.0;
t3009 = -t2991;
t3017 = t2991./2.0;
t3019 = t1552+t1821;
t3025 = t8.*t39.*t2920;
t3029 = -t3015;
t3037 = t3011./2.0;
t3040 = t3015./2.0;
t3047 = t1545+t1858;
t3049 = t14.*t3027;
t3054 = t3044.*(-1.0./2.0);
t3055 = t8.*t3022;
t3065 = t3044./2.0;
t3067 = t1145+t1201+t1204;
t3068 = t1146+t1202+t1205;
t3074 = t8.*t3036;
t3091 = t1587+t1914;
t3095 = t3058.*t6d;
t3096 = -t3070;
t3104 = t1739+t1810;
t3105 = t1783+t1785;
t3110 = t8.*t37.*t3027;
t3111 = t3076./2.0;
t3112 = t8.*t39.*t3027;
t3117 = t1626+t1950;
t3118 = t1676+t1853;
t3124 = -t3098;
t3134 = t1239+t1240+t1241;
t3136 = t35.*t39.*t3027;
t3137 = t3098./2.0;
t3143 = t14.*t37.*t3036;
t3146 = t14.*t39.*t3036;
t3150 = t1702+t1895;
t3153 = t330.*t2920;
t3156 = t8.*t3107;
t3159 = t14.*t3106;
t3174 = t8.*(t1853-t908.*(t101-t401));
t3187 = t38.*t39.*t3036;
Y = ft_7({t100,t1002,t1003,t1004,t1007,t1009,t101,t1012,t1015,t1016,t1017,t1019,t1021,t1022,t1026,t1028,t1031,t1035,t1036,t1038,t1039,t104,t1044,t1045,t1046,t1047,t1048,t1049,t1053,t1054,t1055,t1059,t106,t1064,t1066,t1068,t1069,t107,t1070,t1071,t1072,t1078,t1079,t108,t1080,t1081,t1082,t1083,t1084,t1085,t1086,t1087,t1088,t1089,t1091,t1092,t1093,t1094,t1096,t1097,t1098,t1099,t1100,t1101,t1106,t1108,t1109,t111,t1110,t1111,t112,t1121,t1122,t1123,t1125,t1126,t1128,t1129,t113,t1132,t1133,t1134,t1135,t1136,t1137,t1138,t1139,t1140,t1143,t1147,t1148,t1152,t1155,t1156,t1158,t1160,t1162,t1164,t1166,t1171,t1172,t1173,t1174,t1181,t1182,t1183,t1184,t1185,t1186,t1187,t1189,t1191,t1193,t1196,t12,t1203,t1206,t1207,t1208,t1209,t1210,t1211,t1212,t1222,t1224,t1225,t1226,t1227,t1229,t1230,t1235,t1236,t1237,t1238,t124,t1245,t1246,t1247,t1248,t1249,t1250,t1251,t1252,t1255,t1264,t1265,t1266,t1268,t127,t1271,t1272,t1273,t1274,t128,t1281,t1282,t1283,t1284,t1285,t1286,t1287,t1288,t1289,t1292,t1294,t1297,t1298,t13,t1300,t1302,t1304,t1306,t1307,t131,t1311,t1312,t1313,t1314,t1316,t1317,t132,t1321,t1323,t1324,t1325,t1328,t1329,t1330,t1331,t1332,t1333,t1334,t1335,t1336,t1337,t1339,t134,t1341,t1343,t1346,t1347,t1348,t1350,t1352,t1353,t1355,t1356,t1357,t1358,t1359,t136,t1360,t1361,t1363,t1366,t1367,t1368,t1369,t137,t1371,t1374,t1375,t1376,t1377,t1378,t1379,t138,t1382,t1383,t1385,t1387,t1388,t1389,t1391,t1392,t1393,t1395,t1396,t1398,t1399,t14,t1400,t1402,t1403,t1406,t1408,t1410,t1411,t1412,t1413,t1414,t1415,t1416,t1417,t1418,t1419,t1420,t1423,t1425,t1427,t1428,t1429,t1430,t1434,t1435,t1436,t1437,t1438,t1440,t1445,t1447,t1448,t1449,t1451,t1457,t1458,t1461,t1464,t1465,t1468,t1470,t1471,t1472,t1473,t1474,t1475,t1476,t1477,t1478,t1480,t1483,t1484,t1485,t1486,t1491,t1492,t1493,t1496,t1497,t1499,t15,t150,t1500,t1501,t1503,t1504,t1507,t1514,t1516,t1517,t1518,t1519,t152,t1520,t1521,t1524,t1525,t1527,t1528,t1529,t1531,t1532,t1534,t1535,t1536,t1537,t1538,t1546,t1547,t1549,t155,t1553,t1554,t1555,t1556,t1557,t1558,t156,t1560,t1561,t1562,t1565,t1569,t1571,t1572,t1574,t1577,t1578,t1579,t158,t1580,t1583,t1585,t1586,t1588,t1589,t159,t1590,t1591,t1594,t1597,t1598,t1599,t1600,t1601,t1602,t1603,t1604,t1605,t1606,t1607,t1608,t1609,t1610,t1611,t1612,t1613,t1614,t1615,t1616,t1617,t1618,t1619,t162,t1620,t1621,t1622,t1623,t1624,t1625,t1627,t1628,t163,t1630,t1631,t1632,t1633,t1634,t1635,t1636,t1637,t1638,t164,t1641,t1642,t1643,t1645,t1646,t1647,t1648,t1649,t165,t1650,t1651,t1652,t1653,t1654,t1656,t1658,t1659,t1660,t1663,t1664,t1665,t1667,t1670,t1671,t1672,t1674,t1675,t1677,t1678,t1680,t1681,t1682,t1683,t1685,t1686,t1687,t1688,t1689,t1690,t1691,t1692,t1693,t1696,t1697,t1698,t1699,t1700,t1701,t1704,t1706,t1707,t1708,t1709,t171,t1710,t1713,t1714,t1715,t1717,t1718,t1719,t1721,t1722,t1723,t1724,t1725,t173,t1733,t1735,t1736,t1738,t174,t1740,t1741,t1742,t1743,t1744,t1746,t1747,t175,t1751,t1754,t1755,t1758,t1759,t1760,t1763,t1764,t1766,t1767,t177,t1775,t1776,t1779,t1780,t1781,t1782,t1783,t1784,t1786,t1790,t1792,t1794,t1796,t1797,t1798,t1799,t18,t1800,t1801,t1802,t1803,t1806,t1807,t1809,t1813,t1814,t1815,t1816,t1818,t1824,t1825,t1826,t1827,t1828,t1829,t1830,t1832,t1834,t1835,t1837,t1840,t1841,t1842,t1844,t1845,t1846,t1848,t1849,t1851,t1852,t1853,t1854,t1858,t1859,t1860,t1862,t1863,t1864,t1865,t1866,t1867,t1868,t1869,t187,t1871,t1873,t1874,t1875,t1876,t1877,t1878,t1879,t1880,t1881,t1882,t1883,t1884,t1886,t1887,t1888,t1889,t1890,t1891,t1892,t1893,t1894,t1899,t19,t1900,t1901,t1902,t1903,t1904,t1905,t1907,t191,t1911,t1912,t1913,t1915,t1916,t1917,t1918,t1919,t1920,t1921,t1923,t1925,t1926,t1927,t1929,t1930,t1933,t1934,t1935,t1936,t1938,t1940,t1941,t1944,t1945,t1947,t1948,t1949,t1951,t1952,t1959,t1960,t1961,t1962,t1963,t1964,t1965,t1966,t1967,t1968,t1969,t1970,t1971,t1972,t1973,t1974,t1975,t1976,t1977,t1978,t1979,t1980,t1981,t1982,t1983,t1984,t1985,t1988,t199,t1990,t1991,t1992,t1993,t1995,t1996,t1997,t1999,t1d,t1dd,t200,t2000,t2001,t2004,t2009,t201,t2010,t2012,t2013,t2014,t2015,t2016,t2018,t202,t2020,t2021,t2022,t2023,t2024,t2026,t2027,t2028,t2029,t2031,t2032,t2033,t2042,t2044,t2053,t2054,t2057,t2059,t206,t2060,t2061,t2062,t2064,t2065,t2067,t2068,t2069,t2070,t2071,t2072,t2074,t2075,t2079,t2080,t2081,t2083,t2085,t2086,t2087,t2090,t2091,t2092,t2093,t2095,t2096,t2098,t2099,t21,t2100,t2101,t2102,t2104,t2105,t2107,t2108,t2109,t2111,t2112,t2113,t2114,t2117,t2118,t2119,t2121,t2122,t2123,t2124,t2126,t2128,t2132,t2135,t2136,t2138,t2139,t2140,t2141,t2142,t2143,t2144,t2145,t2146,t2147,t215,t2150,t2152,t2153,t2154,t2155,t2156,t2157,t2159,t2160,t2162,t2163,t2164,t2165,t2166,t2167,t2168,t2169,t2170,t2171,t2173,t2174,t2178,t2180,t2181,t2183,t2184,t2189,t219,t2190,t2193,t2194,t2196,t2198,t22,t220,t2200,t2202,t2204,t2206,t2207,t2208,t221,t2210,t2213,t2216,t2219,t2220,t2221,t2222,t2223,t2224,t2225,t2226,t2227,t2228,t2229,t2230,t2233,t2235,t2241,t2242,t2243,t2244,t2245,t2246,t2247,t2249,t2250,t2256,t2257,t2259,t226,t2260,t2261,t2262,t2263,t2264,t2265,t2267,t2268,t2270,t2271,t2278,t2279,t2281,t2282,t2283,t2284,t2286,t2289,t229,t2291,t2292,t2293,t2294,t2295,t2296,t23,t2300,t2304,t2305,t2306,t2307,t2308,t2311,t2314,t2317,t2319,t232,t2320,t2321,t2322,t2324,t2325,t2326,t2327,t2329,t233,t2330,t2331,t2332,t2339,t2340,t2344,t2345,t2346,t2348,t2349,t2351,t2352,t2353,t2354,t2355,t2356,t2357,t2358,t2359,t2361,t2363,t2365,t2366,t2367,t2368,t2369,t2370,t2371,t2372,t2373,t2374,t2375,t2376,t2377,t2378,t2379,t2380,t2381,t2382,t2384,t2385,t2387,t2388,t2392,t2393,t2394,t2395,t2396,t2397,t2398,t2399,t24,t2400,t2401,t2402,t2403,t2405,t2406,t2407,t2409,t2411,t2412,t2414,t2415,t2416,t2418,t2420,t2421,t2423,t2424,t2427,t2428,t2429,t243,t2432,t2433,t2434,t2438,t244,t2440,t2441,t2442,t2447,t2448,t2449,t245,t2450,t2451,t2452,t2453,t2454,t2455,t2457,t2459,t2460,t2463,t2467,t247,t2471,t2472,t2473,t2475,t2476,t2477,t2478,t2479,t248,t2484,t2486,t2488,t2489,t249,t2490,t2491,t2492,t2493,t2494,t2497,t2498,t2499,t25,t2500,t2501,t2502,t2503,t2504,t2506,t2507,t2508,t2509,t2511,t2512,t2513,t2517,t2520,t2521,t2522,t2523,t2525,t2526,t2527,t2529,t2530,t2532,t2533,t2534,t2535,t2536,t2541,t2543,t2546,t2548,t2549,t255,t2550,t2551,t2555,t2557,t2558,t2559,t256,t2562,t2566,t2569,t2573,t2574,t2576,t2578,t2580,t2582,t2583,t2584,t2585,t2586,t2587,t2588,t2589,t2590,t2592,t2593,t2595,t2599,t26,t2604,t2606,t2607,t2608,t2609,t2610,t2611,t2619,t2620,t2621,t2622,t2624,t2625,t2628,t2629,t2630,t2631,t2632,t2636,t2642,t2644,t2645,t2646,t2647,t2648,t2651,t2652,t2653,t2654,t2655,t2656,t2658,t2659,t2661,t2664,t2666,t2673,t2675,t2677,t2678,t2679,t2680,t2681,t2682,t2684,t2686,t2687,t2689,t2690,t2696,t2697,t2699,t27,t2701,t2702,t2703,t2704,t2705,t2707,t2708,t2709,t2710,t2711,t2712,t2713,t2715,t2716,t2717,t2718,t2719,t2720,t2721,t2722,t2723,t2724,t2725,t2727,t2731,t2734,t2737,t2738,t2740,t2743,t2744,t2745,t2747,t2749,t2750,t2751,t2752,t2754,t2755,t2757,t2759,t2760,t2761,t2762,t2764,t2765,t2766,t2768,t2769,t2772,t2775,t2776,t2777,t2779,t2780,t2781,t2782,t2789,t279,t2790,t2795,t2796,t2797,t2798,t2799,t2800,t2801,t2802,t2804,t2806,t2807,t2808,t2810,t2812,t2813,t2815,t2816,t2817,t2818,t2819,t2820,t2823,t2825,t2826,t2827,t2828,t2829,t283,t2830,t2833,t2835,t2836,t2837,t2838,t2839,t2840,t2841,t2842,t2843,t2848,t2849,t2853,t2854,t2855,t2856,t2857,t2858,t2859,t2860,t2862,t2863,t2865,t2867,t2868,t2871,t2876,t2877,t2878,t2879,t2880,t2881,t2882,t2883,t2884,t2885,t2891,t2892,t2893,t2894,t2895,t2897,t2899,t29,t2900,t2901,t2910,t2911,t2912,t2913,t2914,t2915,t2916,t2917,t2919,t2925,t2927,t2928,t2929,t2933,t2934,t2935,t2936,t2937,t2940,t2942,t2944,t2946,t2947,t2948,t2949,t2951,t2953,t2954,t2956,t2959,t2961,t2966,t2967,t2968,t2970,t2971,t2974,t2975,t2978,t2979,t2982,t2983,t2985,t2988,t2989,t299,t2991,t2992,t2994,t2995,t2996,t2997,t2998,t2999,t2d,t2dd,t30,t3004,t3005,t3007,t3008,t3009,t301,t3010,t3011,t3012,t3013,t3014,t3016,t3017,t3018,t3019,t3020,t3021,t3024,t3025,t3027,t3028,t3029,t3031,t3032,t3035,t3036,t3037,t3040,t3041,t3042,t3043,t3044,t3047,t3049,t3055,t3056,t3058,t3059,t3061,t3064,t3065,t3066,t3067,t3068,t3069,t3073,t3074,t3076,t3078,t3079,t308,t3080,t3081,t3082,t3083,t3086,t3087,t3088,t3090,t3091,t3095,t3096,t3097,t3098,t3099,t31,t3100,t3101,t3104,t3106,t3107,t3110,t3111,t3112,t3121,t3123,t3124,t3125,t3129,t3130,t3134,t3136,t3137,t3140,t3143,t3146,t315,t3150,t3151,t3152,t3153,t3156,t3158,t3159,t3162,t3163,t3165,t3166,t3168,t3169,t317,t3174,t3175,t3176,t3177,t3179,t318,t3182,t3183,t3185,t3187,t319,t3204,t321,t3214,t3220,t3230,t3231,t3232,t3234,t3235,t3236,t3237,t3238,t3240,t3246,t325,t3250,t3251,t3259,t3260,t3272,t3283,t3285,t3288,t3289,t329,t3291,t3292,t3298,t330,t3306,t3308,t331,t3318,t332,t3321,t3326,t333,t3330,t3331,t3332,t3335,t3340,t3348,t3349,t3351,t3354,t3355,t3357,t3358,t3359,t3360,t3377,t3380,t3381,t3383,t3384,t3388,t3390,t3391,t3399,t34,t3400,t3401,t3404,t3405,t341,t3414,t3415,t3416,t342,t3421,t3428,t3429,t343,t3431,t3432,t3439,t344,t3440,t3445,t345,t3452,t3456,t3457,t3458,t3459,t346,t3460,t3461,t3464,t3468,t3469,t347,t3472,t3473,t3477,t3478,t3483,t3487,t3488,t35,t3504,t3509,t3510,t3516,t3517,t3521,t3522,t3523,t3532,t354,t3543,t3544,t3546,t3555,t3556,t3557,t3562,t3567,t3568,t3574,t3575,t3577,t3578,t3579,t3580,t3582,t3590,t3598,t36,t3600,t3601,t3602,t3606,t3607,t3612,t3613,t3614,t3617,t3622,t3623,t3625,t3628,t3630,t3634,t364,t3649,t365,t3651,t3674,t3678,t368,t3683,t3685,t3686,t3687,t3688,t3697,t37,t3701,t3704,t3712,t3716,t3722,t3724,t3732,t3734,t3741,t3743,t3744,t3745,t3747,t3750,t3751,t3754,t3755,t3756,t3757,t3758,t3761,t3762,t3767,t3768,t3769,t3770,t3771,t3781,t3784,t3785,t3789,t3792,t3796,t38,t3804,t3812,t3813,t3817,t3821,t3822,t3826,t3828,t3830,t3833,t384,t3840,t3843,t3845,t3846,t3848,t3852,t3853,t3871,t3872,t3874,t3875,t3877,t3878,t3887,t3888,t3897,t39,t3903,t3906,t3917,t392,t3923,t393,t3936,t3941,t3943,t3948,t3949,t3956,t3965,t3967,t3972,t3974,t3976,t3982,t3997,t3d,t3dd,t4003,t4004,t4006,t4007,t401,t4012,t4018,t402,t4024,t4025,t4027,t4028,t403,t404,t4042,t4048,t4049,t4050,t4055,t4058,t4059,t4069,t4071,t4076,t4077,t4084,t4085,t4086,t4096,t4098,t41,t4102,t4109,t4112,t4115,t4118,t4125,t4126,t4128,t4129,t4130,t4131,t4133,t4134,t4136,t4139,t4140,t4142,t4143,t4144,t4146,t4147,t4149,t4150,t4151,t4152,t4157,t4158,t4159,t4160,t4162,t4164,t4166,t4170,t4171,t4172,t4173,t4175,t4176,t4178,t4179,t418,t4183,t4185,t4186,t4188,t419,t42,t420,t4203,t4204,t4212,t4221,t4226,t4230,t4231,t4233,t4236,t4237,t425,t4252,t4256,t4268,t4273,t4290,t4296,t4299,t4304,t4309,t431,t4321,t4324,t4325,t4326,t4327,t4332,t4333,t4334,t4335,t434,t4342,t4348,t4353,t4361,t4367,t437,t4381,t4386,t4394,t4395,t4397,t4403,t4406,t441,t4413,t442,t4421,t4424,t4429,t443,t4430,t4442,t4443,t4451,t446,t4468,t4469,t4470,t4471,t4475,t4483,t4486,t4487,t4491,t4494,t4499,t4513,t4528,t453,t4534,t4538,t4539,t454,t4540,t4541,t4547,t4548,t4551,t4556,t4560,t4573,t4579,t4582,t4584,t459,t4591,t4595,t4596,t4604,t4627,t4648,t4665,t4668,t4669,t4678,t4695,t470,t4704,t4705,t4707,t4747,t4759,t4776,t478,t4785,t4787,t4789,t4798,t48,t4800,t4801,t483,t4831,t4837,t4838,t484,t4853,t4856,t4858,t486,t4862,t4863,t4867,t487,t4870,t488,t4881,t4887,t4889,t4893,t4907,t4908,t4917,t492,t4921,t4923,t4924,t493,t4930,t4931,t494,t4940,t4941,t4944,t4949,t495,t4950,t4955,t4957,t496,t497,t4979,t498,t4985,t4990,t4992,t4d,t4dd,t50,t5006,t501,t5010,t5012,t5018,t5020,t503,t5047,t5051,t5056,t5074,t508,t5093,t51,t5106,t5114,t514,t515,t516,t519,t523,t524,t5283,t529,t5292,t53,t530,t532,t537,t543,t544,t546,t5465,t547,t548,t549,t55,t552,t553,t554,t56,t562,t569,t57,t570,t58,t582,t588,t589,t591,t593,t596,t598,t5d,t5dd,t601,t602,t604,t608,t609,t61,t612,t614,t615,t616,t617,t623,t627,t63,t632,t633,t634,t635,t636,t637,t639,t641,t642,t643,t644,t645,t646,t647,t648,t649,t650,t652,t653,t655,t659,t664,t665,t667,t668,t670,t671,t675,t680,t681,t682,t684,t685,t687,t689,t69,t690,t691,t694,t695,t696,t698,t699,t6d,t6dd,t701,t702,t703,t705,t706,t71,t711,t712,t713,t714,t720,t721,t723,t725,t726,t729,t731,t732,t733,t735,t736,t738,t739,t745,t746,t747,t748,t75,t752,t755,t759,t760,t761,t763,t764,t772,t774,t775,t776,t781,t785,t788,t789,t793,t8,t802,t806,t82,t820,t823,t824,t825,t826,t827,t828,t831,t832,t833,t838,t842,t843,t844,t846,t848,t849,t850,t851,t852,t853,t854,t855,t859,t861,t865,t870,t871,t873,t879,t880,t884,t885,t890,t892,t896,t897,t898,t899,t9,t900,t907,t908,t909,t910,t915,t917,t919,t922,t923,t927,t928,t930,t932,t937,t943,t944,t945,t949,t952,t959,t961,t962,t963,t964,t965,t966,t967,t969,t970,t972,t973,t976,t978,t979,t981,t982,t983,t986,t987,t989,t992,t996,t999});
end
function Y = ft_7(ct)
t100 = ct{1};
t1002 = ct{2};
t1003 = ct{3};
t1004 = ct{4};
t1007 = ct{5};
t1009 = ct{6};
t101 = ct{7};
t1012 = ct{8};
t1015 = ct{9};
t1016 = ct{10};
t1017 = ct{11};
t1019 = ct{12};
t1021 = ct{13};
t1022 = ct{14};
t1026 = ct{15};
t1028 = ct{16};
t1031 = ct{17};
t1035 = ct{18};
t1036 = ct{19};
t1038 = ct{20};
t1039 = ct{21};
t104 = ct{22};
t1044 = ct{23};
t1045 = ct{24};
t1046 = ct{25};
t1047 = ct{26};
t1048 = ct{27};
t1049 = ct{28};
t1053 = ct{29};
t1054 = ct{30};
t1055 = ct{31};
t1059 = ct{32};
t106 = ct{33};
t1064 = ct{34};
t1066 = ct{35};
t1068 = ct{36};
t1069 = ct{37};
t107 = ct{38};
t1070 = ct{39};
t1071 = ct{40};
t1072 = ct{41};
t1078 = ct{42};
t1079 = ct{43};
t108 = ct{44};
t1080 = ct{45};
t1081 = ct{46};
t1082 = ct{47};
t1083 = ct{48};
t1084 = ct{49};
t1085 = ct{50};
t1086 = ct{51};
t1087 = ct{52};
t1088 = ct{53};
t1089 = ct{54};
t1091 = ct{55};
t1092 = ct{56};
t1093 = ct{57};
t1094 = ct{58};
t1096 = ct{59};
t1097 = ct{60};
t1098 = ct{61};
t1099 = ct{62};
t1100 = ct{63};
t1101 = ct{64};
t1106 = ct{65};
t1108 = ct{66};
t1109 = ct{67};
t111 = ct{68};
t1110 = ct{69};
t1111 = ct{70};
t112 = ct{71};
t1121 = ct{72};
t1122 = ct{73};
t1123 = ct{74};
t1125 = ct{75};
t1126 = ct{76};
t1128 = ct{77};
t1129 = ct{78};
t113 = ct{79};
t1132 = ct{80};
t1133 = ct{81};
t1134 = ct{82};
t1135 = ct{83};
t1136 = ct{84};
t1137 = ct{85};
t1138 = ct{86};
t1139 = ct{87};
t1140 = ct{88};
t1143 = ct{89};
t1147 = ct{90};
t1148 = ct{91};
t1152 = ct{92};
t1155 = ct{93};
t1156 = ct{94};
t1158 = ct{95};
t1160 = ct{96};
t1162 = ct{97};
t1164 = ct{98};
t1166 = ct{99};
t1171 = ct{100};
t1172 = ct{101};
t1173 = ct{102};
t1174 = ct{103};
t1181 = ct{104};
t1182 = ct{105};
t1183 = ct{106};
t1184 = ct{107};
t1185 = ct{108};
t1186 = ct{109};
t1187 = ct{110};
t1189 = ct{111};
t1191 = ct{112};
t1193 = ct{113};
t1196 = ct{114};
t12 = ct{115};
t1203 = ct{116};
t1206 = ct{117};
t1207 = ct{118};
t1208 = ct{119};
t1209 = ct{120};
t1210 = ct{121};
t1211 = ct{122};
t1212 = ct{123};
t1222 = ct{124};
t1224 = ct{125};
t1225 = ct{126};
t1226 = ct{127};
t1227 = ct{128};
t1229 = ct{129};
t1230 = ct{130};
t1235 = ct{131};
t1236 = ct{132};
t1237 = ct{133};
t1238 = ct{134};
t124 = ct{135};
t1245 = ct{136};
t1246 = ct{137};
t1247 = ct{138};
t1248 = ct{139};
t1249 = ct{140};
t1250 = ct{141};
t1251 = ct{142};
t1252 = ct{143};
t1255 = ct{144};
t1264 = ct{145};
t1265 = ct{146};
t1266 = ct{147};
t1268 = ct{148};
t127 = ct{149};
t1271 = ct{150};
t1272 = ct{151};
t1273 = ct{152};
t1274 = ct{153};
t128 = ct{154};
t1281 = ct{155};
t1282 = ct{156};
t1283 = ct{157};
t1284 = ct{158};
t1285 = ct{159};
t1286 = ct{160};
t1287 = ct{161};
t1288 = ct{162};
t1289 = ct{163};
t1292 = ct{164};
t1294 = ct{165};
t1297 = ct{166};
t1298 = ct{167};
t13 = ct{168};
t1300 = ct{169};
t1302 = ct{170};
t1304 = ct{171};
t1306 = ct{172};
t1307 = ct{173};
t131 = ct{174};
t1311 = ct{175};
t1312 = ct{176};
t1313 = ct{177};
t1314 = ct{178};
t1316 = ct{179};
t1317 = ct{180};
t132 = ct{181};
t1321 = ct{182};
t1323 = ct{183};
t1324 = ct{184};
t1325 = ct{185};
t1328 = ct{186};
t1329 = ct{187};
t1330 = ct{188};
t1331 = ct{189};
t1332 = ct{190};
t1333 = ct{191};
t1334 = ct{192};
t1335 = ct{193};
t1336 = ct{194};
t1337 = ct{195};
t1339 = ct{196};
t134 = ct{197};
t1341 = ct{198};
t1343 = ct{199};
t1346 = ct{200};
t1347 = ct{201};
t1348 = ct{202};
t1350 = ct{203};
t1352 = ct{204};
t1353 = ct{205};
t1355 = ct{206};
t1356 = ct{207};
t1357 = ct{208};
t1358 = ct{209};
t1359 = ct{210};
t136 = ct{211};
t1360 = ct{212};
t1361 = ct{213};
t1363 = ct{214};
t1366 = ct{215};
t1367 = ct{216};
t1368 = ct{217};
t1369 = ct{218};
t137 = ct{219};
t1371 = ct{220};
t1374 = ct{221};
t1375 = ct{222};
t1376 = ct{223};
t1377 = ct{224};
t1378 = ct{225};
t1379 = ct{226};
t138 = ct{227};
t1382 = ct{228};
t1383 = ct{229};
t1385 = ct{230};
t1387 = ct{231};
t1388 = ct{232};
t1389 = ct{233};
t1391 = ct{234};
t1392 = ct{235};
t1393 = ct{236};
t1395 = ct{237};
t1396 = ct{238};
t1398 = ct{239};
t1399 = ct{240};
t14 = ct{241};
t1400 = ct{242};
t1402 = ct{243};
t1403 = ct{244};
t1406 = ct{245};
t1408 = ct{246};
t1410 = ct{247};
t1411 = ct{248};
t1412 = ct{249};
t1413 = ct{250};
t1414 = ct{251};
t1415 = ct{252};
t1416 = ct{253};
t1417 = ct{254};
t1418 = ct{255};
t1419 = ct{256};
t1420 = ct{257};
t1423 = ct{258};
t1425 = ct{259};
t1427 = ct{260};
t1428 = ct{261};
t1429 = ct{262};
t1430 = ct{263};
t1434 = ct{264};
t1435 = ct{265};
t1436 = ct{266};
t1437 = ct{267};
t1438 = ct{268};
t1440 = ct{269};
t1445 = ct{270};
t1447 = ct{271};
t1448 = ct{272};
t1449 = ct{273};
t1451 = ct{274};
t1457 = ct{275};
t1458 = ct{276};
t1461 = ct{277};
t1464 = ct{278};
t1465 = ct{279};
t1468 = ct{280};
t1470 = ct{281};
t1471 = ct{282};
t1472 = ct{283};
t1473 = ct{284};
t1474 = ct{285};
t1475 = ct{286};
t1476 = ct{287};
t1477 = ct{288};
t1478 = ct{289};
t1480 = ct{290};
t1483 = ct{291};
t1484 = ct{292};
t1485 = ct{293};
t1486 = ct{294};
t1491 = ct{295};
t1492 = ct{296};
t1493 = ct{297};
t1496 = ct{298};
t1497 = ct{299};
t1499 = ct{300};
t15 = ct{301};
t150 = ct{302};
t1500 = ct{303};
t1501 = ct{304};
t1503 = ct{305};
t1504 = ct{306};
t1507 = ct{307};
t1514 = ct{308};
t1516 = ct{309};
t1517 = ct{310};
t1518 = ct{311};
t1519 = ct{312};
t152 = ct{313};
t1520 = ct{314};
t1521 = ct{315};
t1524 = ct{316};
t1525 = ct{317};
t1527 = ct{318};
t1528 = ct{319};
t1529 = ct{320};
t1531 = ct{321};
t1532 = ct{322};
t1534 = ct{323};
t1535 = ct{324};
t1536 = ct{325};
t1537 = ct{326};
t1538 = ct{327};
t1546 = ct{328};
t1547 = ct{329};
t1549 = ct{330};
t155 = ct{331};
t1553 = ct{332};
t1554 = ct{333};
t1555 = ct{334};
t1556 = ct{335};
t1557 = ct{336};
t1558 = ct{337};
t156 = ct{338};
t1560 = ct{339};
t1561 = ct{340};
t1562 = ct{341};
t1565 = ct{342};
t1569 = ct{343};
t1571 = ct{344};
t1572 = ct{345};
t1574 = ct{346};
t1577 = ct{347};
t1578 = ct{348};
t1579 = ct{349};
t158 = ct{350};
t1580 = ct{351};
t1583 = ct{352};
t1585 = ct{353};
t1586 = ct{354};
t1588 = ct{355};
t1589 = ct{356};
t159 = ct{357};
t1590 = ct{358};
t1591 = ct{359};
t1594 = ct{360};
t1597 = ct{361};
t1598 = ct{362};
t1599 = ct{363};
t1600 = ct{364};
t1601 = ct{365};
t1602 = ct{366};
t1603 = ct{367};
t1604 = ct{368};
t1605 = ct{369};
t1606 = ct{370};
t1607 = ct{371};
t1608 = ct{372};
t1609 = ct{373};
t1610 = ct{374};
t1611 = ct{375};
t1612 = ct{376};
t1613 = ct{377};
t1614 = ct{378};
t1615 = ct{379};
t1616 = ct{380};
t1617 = ct{381};
t1618 = ct{382};
t1619 = ct{383};
t162 = ct{384};
t1620 = ct{385};
t1621 = ct{386};
t1622 = ct{387};
t1623 = ct{388};
t1624 = ct{389};
t1625 = ct{390};
t1627 = ct{391};
t1628 = ct{392};
t163 = ct{393};
t1630 = ct{394};
t1631 = ct{395};
t1632 = ct{396};
t1633 = ct{397};
t1634 = ct{398};
t1635 = ct{399};
t1636 = ct{400};
t1637 = ct{401};
t1638 = ct{402};
t164 = ct{403};
t1641 = ct{404};
t1642 = ct{405};
t1643 = ct{406};
t1645 = ct{407};
t1646 = ct{408};
t1647 = ct{409};
t1648 = ct{410};
t1649 = ct{411};
t165 = ct{412};
t1650 = ct{413};
t1651 = ct{414};
t1652 = ct{415};
t1653 = ct{416};
t1654 = ct{417};
t1656 = ct{418};
t1658 = ct{419};
t1659 = ct{420};
t1660 = ct{421};
t1663 = ct{422};
t1664 = ct{423};
t1665 = ct{424};
t1667 = ct{425};
t1670 = ct{426};
t1671 = ct{427};
t1672 = ct{428};
t1674 = ct{429};
t1675 = ct{430};
t1677 = ct{431};
t1678 = ct{432};
t1680 = ct{433};
t1681 = ct{434};
t1682 = ct{435};
t1683 = ct{436};
t1685 = ct{437};
t1686 = ct{438};
t1687 = ct{439};
t1688 = ct{440};
t1689 = ct{441};
t1690 = ct{442};
t1691 = ct{443};
t1692 = ct{444};
t1693 = ct{445};
t1696 = ct{446};
t1697 = ct{447};
t1698 = ct{448};
t1699 = ct{449};
t1700 = ct{450};
t1701 = ct{451};
t1704 = ct{452};
t1706 = ct{453};
t1707 = ct{454};
t1708 = ct{455};
t1709 = ct{456};
t171 = ct{457};
t1710 = ct{458};
t1713 = ct{459};
t1714 = ct{460};
t1715 = ct{461};
t1717 = ct{462};
t1718 = ct{463};
t1719 = ct{464};
t1721 = ct{465};
t1722 = ct{466};
t1723 = ct{467};
t1724 = ct{468};
t1725 = ct{469};
t173 = ct{470};
t1733 = ct{471};
t1735 = ct{472};
t1736 = ct{473};
t1738 = ct{474};
t174 = ct{475};
t1740 = ct{476};
t1741 = ct{477};
t1742 = ct{478};
t1743 = ct{479};
t1744 = ct{480};
t1746 = ct{481};
t1747 = ct{482};
t175 = ct{483};
t1751 = ct{484};
t1754 = ct{485};
t1755 = ct{486};
t1758 = ct{487};
t1759 = ct{488};
t1760 = ct{489};
t1763 = ct{490};
t1764 = ct{491};
t1766 = ct{492};
t1767 = ct{493};
t177 = ct{494};
t1775 = ct{495};
t1776 = ct{496};
t1779 = ct{497};
t1780 = ct{498};
t1781 = ct{499};
t1782 = ct{500};
t1783 = ct{501};
t1784 = ct{502};
t1786 = ct{503};
t1790 = ct{504};
t1792 = ct{505};
t1794 = ct{506};
t1796 = ct{507};
t1797 = ct{508};
t1798 = ct{509};
t1799 = ct{510};
t18 = ct{511};
t1800 = ct{512};
t1801 = ct{513};
t1802 = ct{514};
t1803 = ct{515};
t1806 = ct{516};
t1807 = ct{517};
t1809 = ct{518};
t1813 = ct{519};
t1814 = ct{520};
t1815 = ct{521};
t1816 = ct{522};
t1818 = ct{523};
t1824 = ct{524};
t1825 = ct{525};
t1826 = ct{526};
t1827 = ct{527};
t1828 = ct{528};
t1829 = ct{529};
t1830 = ct{530};
t1832 = ct{531};
t1834 = ct{532};
t1835 = ct{533};
t1837 = ct{534};
t1840 = ct{535};
t1841 = ct{536};
t1842 = ct{537};
t1844 = ct{538};
t1845 = ct{539};
t1846 = ct{540};
t1848 = ct{541};
t1849 = ct{542};
t1851 = ct{543};
t1852 = ct{544};
t1853 = ct{545};
t1854 = ct{546};
t1858 = ct{547};
t1859 = ct{548};
t1860 = ct{549};
t1862 = ct{550};
t1863 = ct{551};
t1864 = ct{552};
t1865 = ct{553};
t1866 = ct{554};
t1867 = ct{555};
t1868 = ct{556};
t1869 = ct{557};
t187 = ct{558};
t1871 = ct{559};
t1873 = ct{560};
t1874 = ct{561};
t1875 = ct{562};
t1876 = ct{563};
t1877 = ct{564};
t1878 = ct{565};
t1879 = ct{566};
t1880 = ct{567};
t1881 = ct{568};
t1882 = ct{569};
t1883 = ct{570};
t1884 = ct{571};
t1886 = ct{572};
t1887 = ct{573};
t1888 = ct{574};
t1889 = ct{575};
t1890 = ct{576};
t1891 = ct{577};
t1892 = ct{578};
t1893 = ct{579};
t1894 = ct{580};
t1899 = ct{581};
t19 = ct{582};
t1900 = ct{583};
t1901 = ct{584};
t1902 = ct{585};
t1903 = ct{586};
t1904 = ct{587};
t1905 = ct{588};
t1907 = ct{589};
t191 = ct{590};
t1911 = ct{591};
t1912 = ct{592};
t1913 = ct{593};
t1915 = ct{594};
t1916 = ct{595};
t1917 = ct{596};
t1918 = ct{597};
t1919 = ct{598};
t1920 = ct{599};
t1921 = ct{600};
t1923 = ct{601};
t1925 = ct{602};
t1926 = ct{603};
t1927 = ct{604};
t1929 = ct{605};
t1930 = ct{606};
t1933 = ct{607};
t1934 = ct{608};
t1935 = ct{609};
t1936 = ct{610};
t1938 = ct{611};
t1940 = ct{612};
t1941 = ct{613};
t1944 = ct{614};
t1945 = ct{615};
t1947 = ct{616};
t1948 = ct{617};
t1949 = ct{618};
t1951 = ct{619};
t1952 = ct{620};
t1959 = ct{621};
t1960 = ct{622};
t1961 = ct{623};
t1962 = ct{624};
t1963 = ct{625};
t1964 = ct{626};
t1965 = ct{627};
t1966 = ct{628};
t1967 = ct{629};
t1968 = ct{630};
t1969 = ct{631};
t1970 = ct{632};
t1971 = ct{633};
t1972 = ct{634};
t1973 = ct{635};
t1974 = ct{636};
t1975 = ct{637};
t1976 = ct{638};
t1977 = ct{639};
t1978 = ct{640};
t1979 = ct{641};
t1980 = ct{642};
t1981 = ct{643};
t1982 = ct{644};
t1983 = ct{645};
t1984 = ct{646};
t1985 = ct{647};
t1988 = ct{648};
t199 = ct{649};
t1990 = ct{650};
t1991 = ct{651};
t1992 = ct{652};
t1993 = ct{653};
t1995 = ct{654};
t1996 = ct{655};
t1997 = ct{656};
t1999 = ct{657};
t1d = ct{658};
t1dd = ct{659};
t200 = ct{660};
t2000 = ct{661};
t2001 = ct{662};
t2004 = ct{663};
t2009 = ct{664};
t201 = ct{665};
t2010 = ct{666};
t2012 = ct{667};
t2013 = ct{668};
t2014 = ct{669};
t2015 = ct{670};
t2016 = ct{671};
t2018 = ct{672};
t202 = ct{673};
t2020 = ct{674};
t2021 = ct{675};
t2022 = ct{676};
t2023 = ct{677};
t2024 = ct{678};
t2026 = ct{679};
t2027 = ct{680};
t2028 = ct{681};
t2029 = ct{682};
t2031 = ct{683};
t2032 = ct{684};
t2033 = ct{685};
t2042 = ct{686};
t2044 = ct{687};
t2053 = ct{688};
t2054 = ct{689};
t2057 = ct{690};
t2059 = ct{691};
t206 = ct{692};
t2060 = ct{693};
t2061 = ct{694};
t2062 = ct{695};
t2064 = ct{696};
t2065 = ct{697};
t2067 = ct{698};
t2068 = ct{699};
t2069 = ct{700};
t2070 = ct{701};
t2071 = ct{702};
t2072 = ct{703};
t2074 = ct{704};
t2075 = ct{705};
t2079 = ct{706};
t2080 = ct{707};
t2081 = ct{708};
t2083 = ct{709};
t2085 = ct{710};
t2086 = ct{711};
t2087 = ct{712};
t2090 = ct{713};
t2091 = ct{714};
t2092 = ct{715};
t2093 = ct{716};
t2095 = ct{717};
t2096 = ct{718};
t2098 = ct{719};
t2099 = ct{720};
t21 = ct{721};
t2100 = ct{722};
t2101 = ct{723};
t2102 = ct{724};
t2104 = ct{725};
t2105 = ct{726};
t2107 = ct{727};
t2108 = ct{728};
t2109 = ct{729};
t2111 = ct{730};
t2112 = ct{731};
t2113 = ct{732};
t2114 = ct{733};
t2117 = ct{734};
t2118 = ct{735};
t2119 = ct{736};
t2121 = ct{737};
t2122 = ct{738};
t2123 = ct{739};
t2124 = ct{740};
t2126 = ct{741};
t2128 = ct{742};
t2132 = ct{743};
t2135 = ct{744};
t2136 = ct{745};
t2138 = ct{746};
t2139 = ct{747};
t2140 = ct{748};
t2141 = ct{749};
t2142 = ct{750};
t2143 = ct{751};
t2144 = ct{752};
t2145 = ct{753};
t2146 = ct{754};
t2147 = ct{755};
t215 = ct{756};
t2150 = ct{757};
t2152 = ct{758};
t2153 = ct{759};
t2154 = ct{760};
t2155 = ct{761};
t2156 = ct{762};
t2157 = ct{763};
t2159 = ct{764};
t2160 = ct{765};
t2162 = ct{766};
t2163 = ct{767};
t2164 = ct{768};
t2165 = ct{769};
t2166 = ct{770};
t2167 = ct{771};
t2168 = ct{772};
t2169 = ct{773};
t2170 = ct{774};
t2171 = ct{775};
t2173 = ct{776};
t2174 = ct{777};
t2178 = ct{778};
t2180 = ct{779};
t2181 = ct{780};
t2183 = ct{781};
t2184 = ct{782};
t2189 = ct{783};
t219 = ct{784};
t2190 = ct{785};
t2193 = ct{786};
t2194 = ct{787};
t2196 = ct{788};
t2198 = ct{789};
t22 = ct{790};
t220 = ct{791};
t2200 = ct{792};
t2202 = ct{793};
t2204 = ct{794};
t2206 = ct{795};
t2207 = ct{796};
t2208 = ct{797};
t221 = ct{798};
t2210 = ct{799};
t2213 = ct{800};
t2216 = ct{801};
t2219 = ct{802};
t2220 = ct{803};
t2221 = ct{804};
t2222 = ct{805};
t2223 = ct{806};
t2224 = ct{807};
t2225 = ct{808};
t2226 = ct{809};
t2227 = ct{810};
t2228 = ct{811};
t2229 = ct{812};
t2230 = ct{813};
t2233 = ct{814};
t2235 = ct{815};
t2241 = ct{816};
t2242 = ct{817};
t2243 = ct{818};
t2244 = ct{819};
t2245 = ct{820};
t2246 = ct{821};
t2247 = ct{822};
t2249 = ct{823};
t2250 = ct{824};
t2256 = ct{825};
t2257 = ct{826};
t2259 = ct{827};
t226 = ct{828};
t2260 = ct{829};
t2261 = ct{830};
t2262 = ct{831};
t2263 = ct{832};
t2264 = ct{833};
t2265 = ct{834};
t2267 = ct{835};
t2268 = ct{836};
t2270 = ct{837};
t2271 = ct{838};
t2278 = ct{839};
t2279 = ct{840};
t2281 = ct{841};
t2282 = ct{842};
t2283 = ct{843};
t2284 = ct{844};
t2286 = ct{845};
t2289 = ct{846};
t229 = ct{847};
t2291 = ct{848};
t2292 = ct{849};
t2293 = ct{850};
t2294 = ct{851};
t2295 = ct{852};
t2296 = ct{853};
t23 = ct{854};
t2300 = ct{855};
t2304 = ct{856};
t2305 = ct{857};
t2306 = ct{858};
t2307 = ct{859};
t2308 = ct{860};
t2311 = ct{861};
t2314 = ct{862};
t2317 = ct{863};
t2319 = ct{864};
t232 = ct{865};
t2320 = ct{866};
t2321 = ct{867};
t2322 = ct{868};
t2324 = ct{869};
t2325 = ct{870};
t2326 = ct{871};
t2327 = ct{872};
t2329 = ct{873};
t233 = ct{874};
t2330 = ct{875};
t2331 = ct{876};
t2332 = ct{877};
t2339 = ct{878};
t2340 = ct{879};
t2344 = ct{880};
t2345 = ct{881};
t2346 = ct{882};
t2348 = ct{883};
t2349 = ct{884};
t2351 = ct{885};
t2352 = ct{886};
t2353 = ct{887};
t2354 = ct{888};
t2355 = ct{889};
t2356 = ct{890};
t2357 = ct{891};
t2358 = ct{892};
t2359 = ct{893};
t2361 = ct{894};
t2363 = ct{895};
t2365 = ct{896};
t2366 = ct{897};
t2367 = ct{898};
t2368 = ct{899};
t2369 = ct{900};
t2370 = ct{901};
t2371 = ct{902};
t2372 = ct{903};
t2373 = ct{904};
t2374 = ct{905};
t2375 = ct{906};
t2376 = ct{907};
t2377 = ct{908};
t2378 = ct{909};
t2379 = ct{910};
t2380 = ct{911};
t2381 = ct{912};
t2382 = ct{913};
t2384 = ct{914};
t2385 = ct{915};
t2387 = ct{916};
t2388 = ct{917};
t2392 = ct{918};
t2393 = ct{919};
t2394 = ct{920};
t2395 = ct{921};
t2396 = ct{922};
t2397 = ct{923};
t2398 = ct{924};
t2399 = ct{925};
t24 = ct{926};
t2400 = ct{927};
t2401 = ct{928};
t2402 = ct{929};
t2403 = ct{930};
t2405 = ct{931};
t2406 = ct{932};
t2407 = ct{933};
t2409 = ct{934};
t2411 = ct{935};
t2412 = ct{936};
t2414 = ct{937};
t2415 = ct{938};
t2416 = ct{939};
t2418 = ct{940};
t2420 = ct{941};
t2421 = ct{942};
t2423 = ct{943};
t2424 = ct{944};
t2427 = ct{945};
t2428 = ct{946};
t2429 = ct{947};
t243 = ct{948};
t2432 = ct{949};
t2433 = ct{950};
t2434 = ct{951};
t2438 = ct{952};
t244 = ct{953};
t2440 = ct{954};
t2441 = ct{955};
t2442 = ct{956};
t2447 = ct{957};
t2448 = ct{958};
t2449 = ct{959};
t245 = ct{960};
t2450 = ct{961};
t2451 = ct{962};
t2452 = ct{963};
t2453 = ct{964};
t2454 = ct{965};
t2455 = ct{966};
t2457 = ct{967};
t2459 = ct{968};
t2460 = ct{969};
t2463 = ct{970};
t2467 = ct{971};
t247 = ct{972};
t2471 = ct{973};
t2472 = ct{974};
t2473 = ct{975};
t2475 = ct{976};
t2476 = ct{977};
t2477 = ct{978};
t2478 = ct{979};
t2479 = ct{980};
t248 = ct{981};
t2484 = ct{982};
t2486 = ct{983};
t2488 = ct{984};
t2489 = ct{985};
t249 = ct{986};
t2490 = ct{987};
t2491 = ct{988};
t2492 = ct{989};
t2493 = ct{990};
t2494 = ct{991};
t2497 = ct{992};
t2498 = ct{993};
t2499 = ct{994};
t25 = ct{995};
t2500 = ct{996};
t2501 = ct{997};
t2502 = ct{998};
t2503 = ct{999};
t2504 = ct{1000};
t2506 = ct{1001};
t2507 = ct{1002};
t2508 = ct{1003};
t2509 = ct{1004};
t2511 = ct{1005};
t2512 = ct{1006};
t2513 = ct{1007};
t2517 = ct{1008};
t2520 = ct{1009};
t2521 = ct{1010};
t2522 = ct{1011};
t2523 = ct{1012};
t2525 = ct{1013};
t2526 = ct{1014};
t2527 = ct{1015};
t2529 = ct{1016};
t2530 = ct{1017};
t2532 = ct{1018};
t2533 = ct{1019};
t2534 = ct{1020};
t2535 = ct{1021};
t2536 = ct{1022};
t2541 = ct{1023};
t2543 = ct{1024};
t2546 = ct{1025};
t2548 = ct{1026};
t2549 = ct{1027};
t255 = ct{1028};
t2550 = ct{1029};
t2551 = ct{1030};
t2555 = ct{1031};
t2557 = ct{1032};
t2558 = ct{1033};
t2559 = ct{1034};
t256 = ct{1035};
t2562 = ct{1036};
t2566 = ct{1037};
t2569 = ct{1038};
t2573 = ct{1039};
t2574 = ct{1040};
t2576 = ct{1041};
t2578 = ct{1042};
t2580 = ct{1043};
t2582 = ct{1044};
t2583 = ct{1045};
t2584 = ct{1046};
t2585 = ct{1047};
t2586 = ct{1048};
t2587 = ct{1049};
t2588 = ct{1050};
t2589 = ct{1051};
t2590 = ct{1052};
t2592 = ct{1053};
t2593 = ct{1054};
t2595 = ct{1055};
t2599 = ct{1056};
t26 = ct{1057};
t2604 = ct{1058};
t2606 = ct{1059};
t2607 = ct{1060};
t2608 = ct{1061};
t2609 = ct{1062};
t2610 = ct{1063};
t2611 = ct{1064};
t2619 = ct{1065};
t2620 = ct{1066};
t2621 = ct{1067};
t2622 = ct{1068};
t2624 = ct{1069};
t2625 = ct{1070};
t2628 = ct{1071};
t2629 = ct{1072};
t2630 = ct{1073};
t2631 = ct{1074};
t2632 = ct{1075};
t2636 = ct{1076};
t2642 = ct{1077};
t2644 = ct{1078};
t2645 = ct{1079};
t2646 = ct{1080};
t2647 = ct{1081};
t2648 = ct{1082};
t2651 = ct{1083};
t2652 = ct{1084};
t2653 = ct{1085};
t2654 = ct{1086};
t2655 = ct{1087};
t2656 = ct{1088};
t2658 = ct{1089};
t2659 = ct{1090};
t2661 = ct{1091};
t2664 = ct{1092};
t2666 = ct{1093};
t2673 = ct{1094};
t2675 = ct{1095};
t2677 = ct{1096};
t2678 = ct{1097};
t2679 = ct{1098};
t2680 = ct{1099};
t2681 = ct{1100};
t2682 = ct{1101};
t2684 = ct{1102};
t2686 = ct{1103};
t2687 = ct{1104};
t2689 = ct{1105};
t2690 = ct{1106};
t2696 = ct{1107};
t2697 = ct{1108};
t2699 = ct{1109};
t27 = ct{1110};
t2701 = ct{1111};
t2702 = ct{1112};
t2703 = ct{1113};
t2704 = ct{1114};
t2705 = ct{1115};
t2707 = ct{1116};
t2708 = ct{1117};
t2709 = ct{1118};
t2710 = ct{1119};
t2711 = ct{1120};
t2712 = ct{1121};
t2713 = ct{1122};
t2715 = ct{1123};
t2716 = ct{1124};
t2717 = ct{1125};
t2718 = ct{1126};
t2719 = ct{1127};
t2720 = ct{1128};
t2721 = ct{1129};
t2722 = ct{1130};
t2723 = ct{1131};
t2724 = ct{1132};
t2725 = ct{1133};
t2727 = ct{1134};
t2731 = ct{1135};
t2734 = ct{1136};
t2737 = ct{1137};
t2738 = ct{1138};
t2740 = ct{1139};
t2743 = ct{1140};
t2744 = ct{1141};
t2745 = ct{1142};
t2747 = ct{1143};
t2749 = ct{1144};
t2750 = ct{1145};
t2751 = ct{1146};
t2752 = ct{1147};
t2754 = ct{1148};
t2755 = ct{1149};
t2757 = ct{1150};
t2759 = ct{1151};
t2760 = ct{1152};
t2761 = ct{1153};
t2762 = ct{1154};
t2764 = ct{1155};
t2765 = ct{1156};
t2766 = ct{1157};
t2768 = ct{1158};
t2769 = ct{1159};
t2772 = ct{1160};
t2775 = ct{1161};
t2776 = ct{1162};
t2777 = ct{1163};
t2779 = ct{1164};
t2780 = ct{1165};
t2781 = ct{1166};
t2782 = ct{1167};
t2789 = ct{1168};
t279 = ct{1169};
t2790 = ct{1170};
t2795 = ct{1171};
t2796 = ct{1172};
t2797 = ct{1173};
t2798 = ct{1174};
t2799 = ct{1175};
t2800 = ct{1176};
t2801 = ct{1177};
t2802 = ct{1178};
t2804 = ct{1179};
t2806 = ct{1180};
t2807 = ct{1181};
t2808 = ct{1182};
t2810 = ct{1183};
t2812 = ct{1184};
t2813 = ct{1185};
t2815 = ct{1186};
t2816 = ct{1187};
t2817 = ct{1188};
t2818 = ct{1189};
t2819 = ct{1190};
t2820 = ct{1191};
t2823 = ct{1192};
t2825 = ct{1193};
t2826 = ct{1194};
t2827 = ct{1195};
t2828 = ct{1196};
t2829 = ct{1197};
t283 = ct{1198};
t2830 = ct{1199};
t2833 = ct{1200};
t2835 = ct{1201};
t2836 = ct{1202};
t2837 = ct{1203};
t2838 = ct{1204};
t2839 = ct{1205};
t2840 = ct{1206};
t2841 = ct{1207};
t2842 = ct{1208};
t2843 = ct{1209};
t2848 = ct{1210};
t2849 = ct{1211};
t2853 = ct{1212};
t2854 = ct{1213};
t2855 = ct{1214};
t2856 = ct{1215};
t2857 = ct{1216};
t2858 = ct{1217};
t2859 = ct{1218};
t2860 = ct{1219};
t2862 = ct{1220};
t2863 = ct{1221};
t2865 = ct{1222};
t2867 = ct{1223};
t2868 = ct{1224};
t2871 = ct{1225};
t2876 = ct{1226};
t2877 = ct{1227};
t2878 = ct{1228};
t2879 = ct{1229};
t2880 = ct{1230};
t2881 = ct{1231};
t2882 = ct{1232};
t2883 = ct{1233};
t2884 = ct{1234};
t2885 = ct{1235};
t2891 = ct{1236};
t2892 = ct{1237};
t2893 = ct{1238};
t2894 = ct{1239};
t2895 = ct{1240};
t2897 = ct{1241};
t2899 = ct{1242};
t29 = ct{1243};
t2900 = ct{1244};
t2901 = ct{1245};
t2910 = ct{1246};
t2911 = ct{1247};
t2912 = ct{1248};
t2913 = ct{1249};
t2914 = ct{1250};
t2915 = ct{1251};
t2916 = ct{1252};
t2917 = ct{1253};
t2919 = ct{1254};
t2925 = ct{1255};
t2927 = ct{1256};
t2928 = ct{1257};
t2929 = ct{1258};
t2933 = ct{1259};
t2934 = ct{1260};
t2935 = ct{1261};
t2936 = ct{1262};
t2937 = ct{1263};
t2940 = ct{1264};
t2942 = ct{1265};
t2944 = ct{1266};
t2946 = ct{1267};
t2947 = ct{1268};
t2948 = ct{1269};
t2949 = ct{1270};
t2951 = ct{1271};
t2953 = ct{1272};
t2954 = ct{1273};
t2956 = ct{1274};
t2959 = ct{1275};
t2961 = ct{1276};
t2966 = ct{1277};
t2967 = ct{1278};
t2968 = ct{1279};
t2970 = ct{1280};
t2971 = ct{1281};
t2974 = ct{1282};
t2975 = ct{1283};
t2978 = ct{1284};
t2979 = ct{1285};
t2982 = ct{1286};
t2983 = ct{1287};
t2985 = ct{1288};
t2988 = ct{1289};
t2989 = ct{1290};
t299 = ct{1291};
t2991 = ct{1292};
t2992 = ct{1293};
